simulink model "IEEE118_FULL_seed17_GFOL_RL_percgfor091_PyStable"  (R2023a)
(part 2 of 3)

  To Workspace_NET.vn102d : ToWorkspace  VariableName=vn102d  SampleTime=sim_config.Tsample
  To Workspace_NET.vn102q : ToWorkspace  VariableName=vn102q  SampleTime=sim_config.Tsample
  To Workspace_NET.vn103d : ToWorkspace  VariableName=vn103d  SampleTime=sim_config.Tsample
  To Workspace_NET.vn103q : ToWorkspace  VariableName=vn103q  SampleTime=sim_config.Tsample
  To Workspace_NET.vn104d : ToWorkspace  VariableName=vn104d  SampleTime=sim_config.Tsample
  To Workspace_NET.vn104q : ToWorkspace  VariableName=vn104q  SampleTime=sim_config.Tsample
  To Workspace_NET.vn105d : ToWorkspace  VariableName=vn105d  SampleTime=sim_config.Tsample
  To Workspace_NET.vn105q : ToWorkspace  VariableName=vn105q  SampleTime=sim_config.Tsample
  To Workspace_NET.vn106d : ToWorkspace  VariableName=vn106d  SampleTime=sim_config.Tsample
  To Workspace_NET.vn106q : ToWorkspace  VariableName=vn106q  SampleTime=sim_config.Tsample
  To Workspace_NET.vn107d : ToWorkspace  VariableName=vn107d  SampleTime=sim_config.Tsample
  To Workspace_NET.vn107q : ToWorkspace  VariableName=vn107q  SampleTime=sim_config.Tsample
  To Workspace_NET.vn108d : ToWorkspace  VariableName=vn108d  SampleTime=sim_config.Tsample
  To Workspace_NET.vn108q : ToWorkspace  VariableName=vn108q  SampleTime=sim_config.Tsample
  To Workspace_NET.vn109d : ToWorkspace  VariableName=vn109d  SampleTime=sim_config.Tsample
  To Workspace_NET.vn109q : ToWorkspace  VariableName=vn109q  SampleTime=sim_config.Tsample
  To Workspace_NET.vn110d : ToWorkspace  VariableName=vn110d  SampleTime=sim_config.Tsample
  To Workspace_NET.vn110q : ToWorkspace  VariableName=vn110q  SampleTime=sim_config.Tsample
  To Workspace_NET.vn112d : ToWorkspace  VariableName=vn112d  SampleTime=sim_config.Tsample
  To Workspace_NET.vn112q : ToWorkspace  VariableName=vn112q  SampleTime=sim_config.Tsample
  To Workspace_NET.vn113d : ToWorkspace  VariableName=vn113d  SampleTime=sim_config.Tsample
  To Workspace_NET.vn113q : ToWorkspace  VariableName=vn113q  SampleTime=sim_config.Tsample
  To Workspace_NET.vn114d : ToWorkspace  VariableName=vn114d  SampleTime=sim_config.Tsample
  To Workspace_NET.vn114q : ToWorkspace  VariableName=vn114q  SampleTime=sim_config.Tsample
  To Workspace_NET.vn115d : ToWorkspace  VariableName=vn115d  SampleTime=sim_config.Tsample
  To Workspace_NET.vn115q : ToWorkspace  VariableName=vn115q  SampleTime=sim_config.Tsample
  To Workspace_NET.vn117d : ToWorkspace  VariableName=vn117d  SampleTime=sim_config.Tsample
  To Workspace_NET.vn117q : ToWorkspace  VariableName=vn117q  SampleTime=sim_config.Tsample
  To Workspace_NET.vn118d : ToWorkspace  VariableName=vn118d  SampleTime=sim_config.Tsample
  To Workspace_NET.vn118q : ToWorkspace  VariableName=vn118q  SampleTime=sim_config.Tsample
  To Workspace_NET.vn11d : ToWorkspace  VariableName=vn11d  SampleTime=sim_config.Tsample
  To Workspace_NET.vn11q : ToWorkspace  VariableName=vn11q  SampleTime=sim_config.Tsample
  To Workspace_NET.vn12d : ToWorkspace  VariableName=vn12d  SampleTime=sim_config.Tsample
  To Workspace_NET.vn12q : ToWorkspace  VariableName=vn12q  SampleTime=sim_config.Tsample
  To Workspace_NET.vn13d : ToWorkspace  VariableName=vn13d  SampleTime=sim_config.Tsample
  To Workspace_NET.vn13q : ToWorkspace  VariableName=vn13q  SampleTime=sim_config.Tsample
  To Workspace_NET.vn14d : ToWorkspace  VariableName=vn14d  SampleTime=sim_config.Tsample
  To Workspace_NET.vn14q : ToWorkspace  VariableName=vn14q  SampleTime=sim_config.Tsample
  To Workspace_NET.vn15d : ToWorkspace  VariableName=vn15d  SampleTime=sim_config.Tsample
  To Workspace_NET.vn15q : ToWorkspace  VariableName=vn15q  SampleTime=sim_config.Tsample
  To Workspace_NET.vn16d : ToWorkspace  VariableName=vn16d  SampleTime=sim_config.Tsample
  To Workspace_NET.vn16q : ToWorkspace  VariableName=vn16q  SampleTime=sim_config.Tsample
  To Workspace_NET.vn17d : ToWorkspace  VariableName=vn17d  SampleTime=sim_config.Tsample
  To Workspace_NET.vn17q : ToWorkspace  VariableName=vn17q  SampleTime=sim_config.Tsample
  To Workspace_NET.vn18d : ToWorkspace  VariableName=vn18d  SampleTime=sim_config.Tsample
  To Workspace_NET.vn18q : ToWorkspace  VariableName=vn18q  SampleTime=sim_config.Tsample
  To Workspace_NET.vn19d : ToWorkspace  VariableName=vn19d  SampleTime=sim_config.Tsample
  To Workspace_NET.vn19q : ToWorkspace  VariableName=vn19q  SampleTime=sim_config.Tsample
  To Workspace_NET.vn1d : ToWorkspace  VariableName=vn1d  SampleTime=sim_config.Tsample
  To Workspace_NET.vn1q : ToWorkspace  VariableName=vn1q  SampleTime=sim_config.Tsample
  To Workspace_NET.vn20d : ToWorkspace  VariableName=vn20d  SampleTime=sim_config.Tsample
  To Workspace_NET.vn20q : ToWorkspace  VariableName=vn20q  SampleTime=sim_config.Tsample
  To Workspace_NET.vn21d : ToWorkspace  VariableName=vn21d  SampleTime=sim_config.Tsample
  To Workspace_NET.vn21q : ToWorkspace  VariableName=vn21q  SampleTime=sim_config.Tsample
  To Workspace_NET.vn22d : ToWorkspace  VariableName=vn22d  SampleTime=sim_config.Tsample
  To Workspace_NET.vn22q : ToWorkspace  VariableName=vn22q  SampleTime=sim_config.Tsample
  To Workspace_NET.vn23d : ToWorkspace  VariableName=vn23d  SampleTime=sim_config.Tsample
  To Workspace_NET.vn23q : ToWorkspace  VariableName=vn23q  SampleTime=sim_config.Tsample
  To Workspace_NET.vn24d : ToWorkspace  VariableName=vn24d  SampleTime=sim_config.Tsample
  To Workspace_NET.vn24q : ToWorkspace  VariableName=vn24q  SampleTime=sim_config.Tsample
  To Workspace_NET.vn25d : ToWorkspace  VariableName=vn25d  SampleTime=sim_config.Tsample
  To Workspace_NET.vn25q : ToWorkspace  VariableName=vn25q  SampleTime=sim_config.Tsample
  To Workspace_NET.vn26d : ToWorkspace  VariableName=vn26d  SampleTime=sim_config.Tsample
  To Workspace_NET.vn26q : ToWorkspace  VariableName=vn26q  SampleTime=sim_config.Tsample
  To Workspace_NET.vn27d : ToWorkspace  VariableName=vn27d  SampleTime=sim_config.Tsample
  To Workspace_NET.vn27q : ToWorkspace  VariableName=vn27q  SampleTime=sim_config.Tsample
  To Workspace_NET.vn28d : ToWorkspace  VariableName=vn28d  SampleTime=sim_config.Tsample
  To Workspace_NET.vn28q : ToWorkspace  VariableName=vn28q  SampleTime=sim_config.Tsample
  To Workspace_NET.vn29d : ToWorkspace  VariableName=vn29d  SampleTime=sim_config.Tsample
  To Workspace_NET.vn29q : ToWorkspace  VariableName=vn29q  SampleTime=sim_config.Tsample
  To Workspace_NET.vn2d : ToWorkspace  VariableName=vn2d  SampleTime=sim_config.Tsample
  To Workspace_NET.vn2q : ToWorkspace  VariableName=vn2q  SampleTime=sim_config.Tsample
  To Workspace_NET.vn30d : ToWorkspace  VariableName=vn30d  SampleTime=sim_config.Tsample
  To Workspace_NET.vn30q : ToWorkspace  VariableName=vn30q  SampleTime=sim_config.Tsample
  To Workspace_NET.vn31d : ToWorkspace  VariableName=vn31d  SampleTime=sim_config.Tsample
  To Workspace_NET.vn31q : ToWorkspace  VariableName=vn31q  SampleTime=sim_config.Tsample
  To Workspace_NET.vn32d : ToWorkspace  VariableName=vn32d  SampleTime=sim_config.Tsample
  To Workspace_NET.vn32q : ToWorkspace  VariableName=vn32q  SampleTime=sim_config.Tsample
  To Workspace_NET.vn33d : ToWorkspace  VariableName=vn33d  SampleTime=sim_config.Tsample
  To Workspace_NET.vn33q : ToWorkspace  VariableName=vn33q  SampleTime=sim_config.Tsample
  To Workspace_NET.vn34d : ToWorkspace  VariableName=vn34d  SampleTime=sim_config.Tsample
  To Workspace_NET.vn34q : ToWorkspace  VariableName=vn34q  SampleTime=sim_config.Tsample
  To Workspace_NET.vn35d : ToWorkspace  VariableName=vn35d  SampleTime=sim_config.Tsample
  To Workspace_NET.vn35q : ToWorkspace  VariableName=vn35q  SampleTime=sim_config.Tsample
  To Workspace_NET.vn36d : ToWorkspace  VariableName=vn36d  SampleTime=sim_config.Tsample
  To Workspace_NET.vn36q : ToWorkspace  VariableName=vn36q  SampleTime=sim_config.Tsample
  To Workspace_NET.vn37d : ToWorkspace  VariableName=vn37d  SampleTime=sim_config.Tsample
  To Workspace_NET.vn37q : ToWorkspace  VariableName=vn37q  SampleTime=sim_config.Tsample
  To Workspace_NET.vn38d : ToWorkspace  VariableName=vn38d  SampleTime=sim_config.Tsample
  To Workspace_NET.vn38q : ToWorkspace  VariableName=vn38q  SampleTime=sim_config.Tsample
  To Workspace_NET.vn39d : ToWorkspace  VariableName=vn39d  SampleTime=sim_config.Tsample
  To Workspace_NET.vn39q : ToWorkspace  VariableName=vn39q  SampleTime=sim_config.Tsample
  To Workspace_NET.vn3d : ToWorkspace  VariableName=vn3d  SampleTime=sim_config.Tsample
  To Workspace_NET.vn3q : ToWorkspace  VariableName=vn3q  SampleTime=sim_config.Tsample
  To Workspace_NET.vn40d : ToWorkspace  VariableName=vn40d  SampleTime=sim_config.Tsample
  To Workspace_NET.vn40q : ToWorkspace  VariableName=vn40q  SampleTime=sim_config.Tsample
  To Workspace_NET.vn41d : ToWorkspace  VariableName=vn41d  SampleTime=sim_config.Tsample
  To Workspace_NET.vn41q : ToWorkspace  VariableName=vn41q  SampleTime=sim_config.Tsample
  To Workspace_NET.vn42d : ToWorkspace  VariableName=vn42d  SampleTime=sim_config.Tsample
  To Workspace_NET.vn42q : ToWorkspace  VariableName=vn42q  SampleTime=sim_config.Tsample
  To Workspace_NET.vn43d : ToWorkspace  VariableName=vn43d  SampleTime=sim_config.Tsample
  To Workspace_NET.vn43q : ToWorkspace  VariableName=vn43q  SampleTime=sim_config.Tsample
  To Workspace_NET.vn44d : ToWorkspace  VariableName=vn44d  SampleTime=sim_config.Tsample
  To Workspace_NET.vn44q : ToWorkspace  VariableName=vn44q  SampleTime=sim_config.Tsample
  To Workspace_NET.vn45d : ToWorkspace  VariableName=vn45d  SampleTime=sim_config.Tsample
  To Workspace_NET.vn45q : ToWorkspace  VariableName=vn45q  SampleTime=sim_config.Tsample
  To Workspace_NET.vn46d : ToWorkspace  VariableName=vn46d  SampleTime=sim_config.Tsample
  To Workspace_NET.vn46q : ToWorkspace  VariableName=vn46q  SampleTime=sim_config.Tsample
  To Workspace_NET.vn47d : ToWorkspace  VariableName=vn47d  SampleTime=sim_config.Tsample
  To Workspace_NET.vn47q : ToWorkspace  VariableName=vn47q  SampleTime=sim_config.Tsample
  To Workspace_NET.vn48d : ToWorkspace  VariableName=vn48d  SampleTime=sim_config.Tsample
  To Workspace_NET.vn48q : ToWorkspace  VariableName=vn48q  SampleTime=sim_config.Tsample
  To Workspace_NET.vn49d : ToWorkspace  VariableName=vn49d  SampleTime=sim_config.Tsample
  To Workspace_NET.vn49q : ToWorkspace  VariableName=vn49q  SampleTime=sim_config.Tsample
  To Workspace_NET.vn4d : ToWorkspace  VariableName=vn4d  SampleTime=sim_config.Tsample
  To Workspace_NET.vn4q : ToWorkspace  VariableName=vn4q  SampleTime=sim_config.Tsample
  To Workspace_NET.vn50d : ToWorkspace  VariableName=vn50d  SampleTime=sim_config.Tsample
  To Workspace_NET.vn50q : ToWorkspace  VariableName=vn50q  SampleTime=sim_config.Tsample
  To Workspace_NET.vn51d : ToWorkspace  VariableName=vn51d  SampleTime=sim_config.Tsample
  To Workspace_NET.vn51q : ToWorkspace  VariableName=vn51q  SampleTime=sim_config.Tsample
  To Workspace_NET.vn52d : ToWorkspace  VariableName=vn52d  SampleTime=sim_config.Tsample
  To Workspace_NET.vn52q : ToWorkspace  VariableName=vn52q  SampleTime=sim_config.Tsample
  To Workspace_NET.vn53d : ToWorkspace  VariableName=vn53d  SampleTime=sim_config.Tsample
  To Workspace_NET.vn53q : ToWorkspace  VariableName=vn53q  SampleTime=sim_config.Tsample
  To Workspace_NET.vn54d : ToWorkspace  VariableName=vn54d  SampleTime=sim_config.Tsample
  To Workspace_NET.vn54q : ToWorkspace  VariableName=vn54q  SampleTime=sim_config.Tsample
  To Workspace_NET.vn55d : ToWorkspace  VariableName=vn55d  SampleTime=sim_config.Tsample
  To Workspace_NET.vn55q : ToWorkspace  VariableName=vn55q  SampleTime=sim_config.Tsample
  To Workspace_NET.vn56d : ToWorkspace  VariableName=vn56d  SampleTime=sim_config.Tsample
  To Workspace_NET.vn56q : ToWorkspace  VariableName=vn56q  SampleTime=sim_config.Tsample
  To Workspace_NET.vn57d : ToWorkspace  VariableName=vn57d  SampleTime=sim_config.Tsample
  To Workspace_NET.vn57q : ToWorkspace  VariableName=vn57q  SampleTime=sim_config.Tsample
  To Workspace_NET.vn58d : ToWorkspace  VariableName=vn58d  SampleTime=sim_config.Tsample
  To Workspace_NET.vn58q : ToWorkspace  VariableName=vn58q  SampleTime=sim_config.Tsample
  To Workspace_NET.vn59d : ToWorkspace  VariableName=vn59d  SampleTime=sim_config.Tsample
  To Workspace_NET.vn59q : ToWorkspace  VariableName=vn59q  SampleTime=sim_config.Tsample
  To Workspace_NET.vn5d : ToWorkspace  VariableName=vn5d  SampleTime=sim_config.Tsample
  To Workspace_NET.vn5q : ToWorkspace  VariableName=vn5q  SampleTime=sim_config.Tsample
  To Workspace_NET.vn60d : ToWorkspace  VariableName=vn60d  SampleTime=sim_config.Tsample
  To Workspace_NET.vn60q : ToWorkspace  VariableName=vn60q  SampleTime=sim_config.Tsample
  To Workspace_NET.vn61d : ToWorkspace  VariableName=vn61d  SampleTime=sim_config.Tsample
  To Workspace_NET.vn61q : ToWorkspace  VariableName=vn61q  SampleTime=sim_config.Tsample
  To Workspace_NET.vn62d : ToWorkspace  VariableName=vn62d  SampleTime=sim_config.Tsample
  To Workspace_NET.vn62q : ToWorkspace  VariableName=vn62q  SampleTime=sim_config.Tsample
  To Workspace_NET.vn63d : ToWorkspace  VariableName=vn63d  SampleTime=sim_config.Tsample
  To Workspace_NET.vn63q : ToWorkspace  VariableName=vn63q  SampleTime=sim_config.Tsample
  To Workspace_NET.vn64d : ToWorkspace  VariableName=vn64d  SampleTime=sim_config.Tsample
  To Workspace_NET.vn64q : ToWorkspace  VariableName=vn64q  SampleTime=sim_config.Tsample
  To Workspace_NET.vn65d : ToWorkspace  VariableName=vn65d  SampleTime=sim_config.Tsample
  To Workspace_NET.vn65q : ToWorkspace  VariableName=vn65q  SampleTime=sim_config.Tsample
  To Workspace_NET.vn66d : ToWorkspace  VariableName=vn66d  SampleTime=sim_config.Tsample
  To Workspace_NET.vn66q : ToWorkspace  VariableName=vn66q  SampleTime=sim_config.Tsample
  To Workspace_NET.vn67d : ToWorkspace  VariableName=vn67d  SampleTime=sim_config.Tsample
  To Workspace_NET.vn67q : ToWorkspace  VariableName=vn67q  SampleTime=sim_config.Tsample
  To Workspace_NET.vn68d : ToWorkspace  VariableName=vn68d  SampleTime=sim_config.Tsample
  To Workspace_NET.vn68q : ToWorkspace  VariableName=vn68q  SampleTime=sim_config.Tsample
  To Workspace_NET.vn69d : ToWorkspace  VariableName=vn69d  SampleTime=sim_config.Tsample
  To Workspace_NET.vn69q : ToWorkspace  VariableName=vn69q  SampleTime=sim_config.Tsample
  To Workspace_NET.vn6d : ToWorkspace  VariableName=vn6d  SampleTime=sim_config.Tsample
  To Workspace_NET.vn6q : ToWorkspace  VariableName=vn6q  SampleTime=sim_config.Tsample
  To Workspace_NET.vn70d : ToWorkspace  VariableName=vn70d  SampleTime=sim_config.Tsample
  To Workspace_NET.vn70q : ToWorkspace  VariableName=vn70q  SampleTime=sim_config.Tsample
  To Workspace_NET.vn71d : ToWorkspace  VariableName=vn71d  SampleTime=sim_config.Tsample
  To Workspace_NET.vn71q : ToWorkspace  VariableName=vn71q  SampleTime=sim_config.Tsample
  To Workspace_NET.vn72d : ToWorkspace  VariableName=vn72d  SampleTime=sim_config.Tsample
  To Workspace_NET.vn72q : ToWorkspace  VariableName=vn72q  SampleTime=sim_config.Tsample
  To Workspace_NET.vn73d : ToWorkspace  VariableName=vn73d  SampleTime=sim_config.Tsample
  To Workspace_NET.vn73q : ToWorkspace  VariableName=vn73q  SampleTime=sim_config.Tsample
  To Workspace_NET.vn74d : ToWorkspace  VariableName=vn74d  SampleTime=sim_config.Tsample
  To Workspace_NET.vn74q : ToWorkspace  VariableName=vn74q  SampleTime=sim_config.Tsample
  To Workspace_NET.vn75d : ToWorkspace  VariableName=vn75d  SampleTime=sim_config.Tsample
  To Workspace_NET.vn75q : ToWorkspace  VariableName=vn75q  SampleTime=sim_config.Tsample
  To Workspace_NET.vn76d : ToWorkspace  VariableName=vn76d  SampleTime=sim_config.Tsample
  To Workspace_NET.vn76q : ToWorkspace  VariableName=vn76q  SampleTime=sim_config.Tsample
  To Workspace_NET.vn77d : ToWorkspace  VariableName=vn77d  SampleTime=sim_config.Tsample
  To Workspace_NET.vn77q : ToWorkspace  VariableName=vn77q  SampleTime=sim_config.Tsample
  To Workspace_NET.vn78d : ToWorkspace  VariableName=vn78d  SampleTime=sim_config.Tsample
  To Workspace_NET.vn78q : ToWorkspace  VariableName=vn78q  SampleTime=sim_config.Tsample
  To Workspace_NET.vn79d : ToWorkspace  VariableName=vn79d  SampleTime=sim_config.Tsample
  To Workspace_NET.vn79q : ToWorkspace  VariableName=vn79q  SampleTime=sim_config.Tsample
  To Workspace_NET.vn7d : ToWorkspace  VariableName=vn7d  SampleTime=sim_config.Tsample
  To Workspace_NET.vn7q : ToWorkspace  VariableName=vn7q  SampleTime=sim_config.Tsample
  To Workspace_NET.vn80d : ToWorkspace  VariableName=vn80d  SampleTime=sim_config.Tsample
  To Workspace_NET.vn80q : ToWorkspace  VariableName=vn80q  SampleTime=sim_config.Tsample
  To Workspace_NET.vn81d : ToWorkspace  VariableName=vn81d  SampleTime=sim_config.Tsample
  To Workspace_NET.vn81q : ToWorkspace  VariableName=vn81q  SampleTime=sim_config.Tsample
  To Workspace_NET.vn82d : ToWorkspace  VariableName=vn82d  SampleTime=sim_config.Tsample
  To Workspace_NET.vn82q : ToWorkspace  VariableName=vn82q  SampleTime=sim_config.Tsample
  To Workspace_NET.vn83d : ToWorkspace  VariableName=vn83d  SampleTime=sim_config.Tsample
  To Workspace_NET.vn83q : ToWorkspace  VariableName=vn83q  SampleTime=sim_config.Tsample
  To Workspace_NET.vn84d : ToWorkspace  VariableName=vn84d  SampleTime=sim_config.Tsample
  To Workspace_NET.vn84q : ToWorkspace  VariableName=vn84q  SampleTime=sim_config.Tsample
  To Workspace_NET.vn85d : ToWorkspace  VariableName=vn85d  SampleTime=sim_config.Tsample
  To Workspace_NET.vn85q : ToWorkspace  VariableName=vn85q  SampleTime=sim_config.Tsample
  To Workspace_NET.vn86d : ToWorkspace  VariableName=vn86d  SampleTime=sim_config.Tsample
  To Workspace_NET.vn86q : ToWorkspace  VariableName=vn86q  SampleTime=sim_config.Tsample
  To Workspace_NET.vn88d : ToWorkspace  VariableName=vn88d  SampleTime=sim_config.Tsample
  To Workspace_NET.vn88q : ToWorkspace  VariableName=vn88q  SampleTime=sim_config.Tsample
  To Workspace_NET.vn89d : ToWorkspace  VariableName=vn89d  SampleTime=sim_config.Tsample
  To Workspace_NET.vn89q : ToWorkspace  VariableName=vn89q  SampleTime=sim_config.Tsample
  To Workspace_NET.vn8d : ToWorkspace  VariableName=vn8d  SampleTime=sim_config.Tsample
  To Workspace_NET.vn8q : ToWorkspace  VariableName=vn8q  SampleTime=sim_config.Tsample
  To Workspace_NET.vn90d : ToWorkspace  VariableName=vn90d  SampleTime=sim_config.Tsample
  To Workspace_NET.vn90q : ToWorkspace  VariableName=vn90q  SampleTime=sim_config.Tsample
  To Workspace_NET.vn91d : ToWorkspace  VariableName=vn91d  SampleTime=sim_config.Tsample
  To Workspace_NET.vn91q : ToWorkspace  VariableName=vn91q  SampleTime=sim_config.Tsample
  To Workspace_NET.vn92d : ToWorkspace  VariableName=vn92d  SampleTime=sim_config.Tsample
  To Workspace_NET.vn92q : ToWorkspace  VariableName=vn92q  SampleTime=sim_config.Tsample
  To Workspace_NET.vn93d : ToWorkspace  VariableName=vn93d  SampleTime=sim_config.Tsample
  To Workspace_NET.vn93q : ToWorkspace  VariableName=vn93q  SampleTime=sim_config.Tsample
  To Workspace_NET.vn94d : ToWorkspace  VariableName=vn94d  SampleTime=sim_config.Tsample
  To Workspace_NET.vn94q : ToWorkspace  VariableName=vn94q  SampleTime=sim_config.Tsample
  To Workspace_NET.vn95d : ToWorkspace  VariableName=vn95d  SampleTime=sim_config.Tsample
  To Workspace_NET.vn95q : ToWorkspace  VariableName=vn95q  SampleTime=sim_config.Tsample
  To Workspace_NET.vn96d : ToWorkspace  VariableName=vn96d  SampleTime=sim_config.Tsample
  To Workspace_NET.vn96q : ToWorkspace  VariableName=vn96q  SampleTime=sim_config.Tsample
  To Workspace_NET.vn97d : ToWorkspace  VariableName=vn97d  SampleTime=sim_config.Tsample
  To Workspace_NET.vn97q : ToWorkspace  VariableName=vn97q  SampleTime=sim_config.Tsample
  To Workspace_NET.vn98d : ToWorkspace  VariableName=vn98d  SampleTime=sim_config.Tsample
  To Workspace_NET.vn98q : ToWorkspace  VariableName=vn98q  SampleTime=sim_config.Tsample
  To Workspace_NET.vn99d : ToWorkspace  VariableName=vn99d  SampleTime=sim_config.Tsample
  To Workspace_NET.vn99q : ToWorkspace  VariableName=vn99q  SampleTime=sim_config.Tsample
  To Workspace_P_Load1 : ToWorkspace  VariableName=P_Load1  SampleTime=sim_config.Tsample
  To Workspace_P_Load10 : ToWorkspace  VariableName=P_Load10  SampleTime=sim_config.Tsample
  To Workspace_P_Load11 : ToWorkspace  VariableName=P_Load11  SampleTime=sim_config.Tsample
  To Workspace_P_Load12 : ToWorkspace  VariableName=P_Load12  SampleTime=sim_config.Tsample
  To Workspace_P_Load13 : ToWorkspace  VariableName=P_Load13  SampleTime=sim_config.Tsample
  To Workspace_P_Load14 : ToWorkspace  VariableName=P_Load14  SampleTime=sim_config.Tsample
  To Workspace_P_Load15 : ToWorkspace  VariableName=P_Load15  SampleTime=sim_config.Tsample
  To Workspace_P_Load16 : ToWorkspace  VariableName=P_Load16  SampleTime=sim_config.Tsample
  To Workspace_P_Load17 : ToWorkspace  VariableName=P_Load17  SampleTime=sim_config.Tsample
  To Workspace_P_Load18 : ToWorkspace  VariableName=P_Load18  SampleTime=sim_config.Tsample
  To Workspace_P_Load19 : ToWorkspace  VariableName=P_Load19  SampleTime=sim_config.Tsample
  To Workspace_P_Load2 : ToWorkspace  VariableName=P_Load2  SampleTime=sim_config.Tsample
  To Workspace_P_Load20 : ToWorkspace  VariableName=P_Load20  SampleTime=sim_config.Tsample
  To Workspace_P_Load21 : ToWorkspace  VariableName=P_Load21  SampleTime=sim_config.Tsample
  To Workspace_P_Load22 : ToWorkspace  VariableName=P_Load22  SampleTime=sim_config.Tsample
  To Workspace_P_Load23 : ToWorkspace  VariableName=P_Load23  SampleTime=sim_config.Tsample
  To Workspace_P_Load24 : ToWorkspace  VariableName=P_Load24  SampleTime=sim_config.Tsample
  To Workspace_P_Load25 : ToWorkspace  VariableName=P_Load25  SampleTime=sim_config.Tsample
  To Workspace_P_Load26 : ToWorkspace  VariableName=P_Load26  SampleTime=sim_config.Tsample
  To Workspace_P_Load27 : ToWorkspace  VariableName=P_Load27  SampleTime=sim_config.Tsample
  To Workspace_P_Load28 : ToWorkspace  VariableName=P_Load28  SampleTime=sim_config.Tsample
  To Workspace_P_Load29 : ToWorkspace  VariableName=P_Load29  SampleTime=sim_config.Tsample
  To Workspace_P_Load3 : ToWorkspace  VariableName=P_Load3  SampleTime=sim_config.Tsample
  To Workspace_P_Load30 : ToWorkspace  VariableName=P_Load30  SampleTime=sim_config.Tsample
  To Workspace_P_Load31 : ToWorkspace  VariableName=P_Load31  SampleTime=sim_config.Tsample
  To Workspace_P_Load32 : ToWorkspace  VariableName=P_Load32  SampleTime=sim_config.Tsample
  To Workspace_P_Load33 : ToWorkspace  VariableName=P_Load33  SampleTime=sim_config.Tsample
  To Workspace_P_Load34 : ToWorkspace  VariableName=P_Load34  SampleTime=sim_config.Tsample
  To Workspace_P_Load35 : ToWorkspace  VariableName=P_Load35  SampleTime=sim_config.Tsample
  To Workspace_P_Load36 : ToWorkspace  VariableName=P_Load36  SampleTime=sim_config.Tsample
  To Workspace_P_Load37 : ToWorkspace  VariableName=P_Load37  SampleTime=sim_config.Tsample
  To Workspace_P_Load38 : ToWorkspace  VariableName=P_Load38  SampleTime=sim_config.Tsample
  To Workspace_P_Load39 : ToWorkspace  VariableName=P_Load39  SampleTime=sim_config.Tsample
  To Workspace_P_Load4 : ToWorkspace  VariableName=P_Load4  SampleTime=sim_config.Tsample
  To Workspace_P_Load40 : ToWorkspace  VariableName=P_Load40  SampleTime=sim_config.Tsample
  To Workspace_P_Load41 : ToWorkspace  VariableName=P_Load41  SampleTime=sim_config.Tsample
  To Workspace_P_Load42 : ToWorkspace  VariableName=P_Load42  SampleTime=sim_config.Tsample
  To Workspace_P_Load43 : ToWorkspace  VariableName=P_Load43  SampleTime=sim_config.Tsample
  To Workspace_P_Load44 : ToWorkspace  VariableName=P_Load44  SampleTime=sim_config.Tsample
  To Workspace_P_Load45 : ToWorkspace  VariableName=P_Load45  SampleTime=sim_config.Tsample
  To Workspace_P_Load46 : ToWorkspace  VariableName=P_Load46  SampleTime=sim_config.Tsample
  To Workspace_P_Load47 : ToWorkspace  VariableName=P_Load47  SampleTime=sim_config.Tsample
  To Workspace_P_Load48 : ToWorkspace  VariableName=P_Load48  SampleTime=sim_config.Tsample
  To Workspace_P_Load49 : ToWorkspace  VariableName=P_Load49  SampleTime=sim_config.Tsample
  To Workspace_P_Load5 : ToWorkspace  VariableName=P_Load5  SampleTime=sim_config.Tsample
  To Workspace_P_Load50 : ToWorkspace  VariableName=P_Load50  SampleTime=sim_config.Tsample
  To Workspace_P_Load51 : ToWorkspace  VariableName=P_Load51  SampleTime=sim_config.Tsample
  To Workspace_P_Load52 : ToWorkspace  VariableName=P_Load52  SampleTime=sim_config.Tsample
  To Workspace_P_Load53 : ToWorkspace  VariableName=P_Load53  SampleTime=sim_config.Tsample
  To Workspace_P_Load54 : ToWorkspace  VariableName=P_Load54  SampleTime=sim_config.Tsample
  To Workspace_P_Load55 : ToWorkspace  VariableName=P_Load55  SampleTime=sim_config.Tsample
  To Workspace_P_Load56 : ToWorkspace  VariableName=P_Load56  SampleTime=sim_config.Tsample
  To Workspace_P_Load57 : ToWorkspace  VariableName=P_Load57  SampleTime=sim_config.Tsample
  To Workspace_P_Load58 : ToWorkspace  VariableName=P_Load58  SampleTime=sim_config.Tsample
  To Workspace_P_Load59 : ToWorkspace  VariableName=P_Load59  SampleTime=sim_config.Tsample
  To Workspace_P_Load6 : ToWorkspace  VariableName=P_Load6  SampleTime=sim_config.Tsample
  To Workspace_P_Load60 : ToWorkspace  VariableName=P_Load60  SampleTime=sim_config.Tsample
  To Workspace_P_Load61 : ToWorkspace  VariableName=P_Load61  SampleTime=sim_config.Tsample
  To Workspace_P_Load62 : ToWorkspace  VariableName=P_Load62  SampleTime=sim_config.Tsample
  To Workspace_P_Load63 : ToWorkspace  VariableName=P_Load63  SampleTime=sim_config.Tsample
  To Workspace_P_Load64 : ToWorkspace  VariableName=P_Load64  SampleTime=sim_config.Tsample
  To Workspace_P_Load65 : ToWorkspace  VariableName=P_Load65  SampleTime=sim_config.Tsample
  To Workspace_P_Load66 : ToWorkspace  VariableName=P_Load66  SampleTime=sim_config.Tsample
  To Workspace_P_Load67 : ToWorkspace  VariableName=P_Load67  SampleTime=sim_config.Tsample
  To Workspace_P_Load68 : ToWorkspace  VariableName=P_Load68  SampleTime=sim_config.Tsample
  To Workspace_P_Load69 : ToWorkspace  VariableName=P_Load69  SampleTime=sim_config.Tsample
  To Workspace_P_Load7 : ToWorkspace  VariableName=P_Load7  SampleTime=sim_config.Tsample
  To Workspace_P_Load70 : ToWorkspace  VariableName=P_Load70  SampleTime=sim_config.Tsample
  To Workspace_P_Load71 : ToWorkspace  VariableName=P_Load71  SampleTime=sim_config.Tsample
  To Workspace_P_Load72 : ToWorkspace  VariableName=P_Load72  SampleTime=sim_config.Tsample
  To Workspace_P_Load73 : ToWorkspace  VariableName=P_Load73  SampleTime=sim_config.Tsample
  To Workspace_P_Load74 : ToWorkspace  VariableName=P_Load74  SampleTime=sim_config.Tsample
  To Workspace_P_Load75 : ToWorkspace  VariableName=P_Load75  SampleTime=sim_config.Tsample
  To Workspace_P_Load76 : ToWorkspace  VariableName=P_Load76  SampleTime=sim_config.Tsample
  To Workspace_P_Load77 : ToWorkspace  VariableName=P_Load77  SampleTime=sim_config.Tsample
  To Workspace_P_Load78 : ToWorkspace  VariableName=P_Load78  SampleTime=sim_config.Tsample
  To Workspace_P_Load79 : ToWorkspace  VariableName=P_Load79  SampleTime=sim_config.Tsample
  To Workspace_P_Load8 : ToWorkspace  VariableName=P_Load8  SampleTime=sim_config.Tsample
  To Workspace_P_Load80 : ToWorkspace  VariableName=P_Load80  SampleTime=sim_config.Tsample
  To Workspace_P_Load81 : ToWorkspace  VariableName=P_Load81  SampleTime=sim_config.Tsample
  To Workspace_P_Load82 : ToWorkspace  VariableName=P_Load82  SampleTime=sim_config.Tsample
  To Workspace_P_Load83 : ToWorkspace  VariableName=P_Load83  SampleTime=sim_config.Tsample
  To Workspace_P_Load84 : ToWorkspace  VariableName=P_Load84  SampleTime=sim_config.Tsample
  To Workspace_P_Load85 : ToWorkspace  VariableName=P_Load85  SampleTime=sim_config.Tsample
  To Workspace_P_Load86 : ToWorkspace  VariableName=P_Load86  SampleTime=sim_config.Tsample
  To Workspace_P_Load87 : ToWorkspace  VariableName=P_Load87  SampleTime=sim_config.Tsample
  To Workspace_P_Load88 : ToWorkspace  VariableName=P_Load88  SampleTime=sim_config.Tsample
  To Workspace_P_Load89 : ToWorkspace  VariableName=P_Load89  SampleTime=sim_config.Tsample
  To Workspace_P_Load9 : ToWorkspace  VariableName=P_Load9  SampleTime=sim_config.Tsample
  To Workspace_P_Load90 : ToWorkspace  VariableName=P_Load90  SampleTime=sim_config.Tsample
  To Workspace_P_Load91 : ToWorkspace  VariableName=P_Load91  SampleTime=sim_config.Tsample
  To Workspace_P_SG1 : ToWorkspace  VariableName=P_SG1  SampleTime=sim_config.Tsample
  To Workspace_P_SG10 : ToWorkspace  VariableName=P_SG10  SampleTime=sim_config.Tsample
  To Workspace_P_SG11 : ToWorkspace  VariableName=P_SG11  SampleTime=sim_config.Tsample
  To Workspace_P_SG12 : ToWorkspace  VariableName=P_SG12  SampleTime=sim_config.Tsample
  To Workspace_P_SG13 : ToWorkspace  VariableName=P_SG13  SampleTime=sim_config.Tsample
  To Workspace_P_SG14 : ToWorkspace  VariableName=P_SG14  SampleTime=sim_config.Tsample
  To Workspace_P_SG15 : ToWorkspace  VariableName=P_SG15  SampleTime=sim_config.Tsample
  To Workspace_P_SG16 : ToWorkspace  VariableName=P_SG16  SampleTime=sim_config.Tsample
  To Workspace_P_SG17 : ToWorkspace  VariableName=P_SG17  SampleTime=sim_config.Tsample
  To Workspace_P_SG18 : ToWorkspace  VariableName=P_SG18  SampleTime=sim_config.Tsample
  To Workspace_P_SG19 : ToWorkspace  VariableName=P_SG19  SampleTime=sim_config.Tsample
  To Workspace_P_SG2 : ToWorkspace  VariableName=P_SG2  SampleTime=sim_config.Tsample
  To Workspace_P_SG20 : ToWorkspace  VariableName=P_SG20  SampleTime=sim_config.Tsample
  To Workspace_P_SG21 : ToWorkspace  VariableName=P_SG21  SampleTime=sim_config.Tsample
  To Workspace_P_SG22 : ToWorkspace  VariableName=P_SG22  SampleTime=sim_config.Tsample
  To Workspace_P_SG23 : ToWorkspace  VariableName=P_SG23  SampleTime=sim_config.Tsample
  To Workspace_P_SG24 : ToWorkspace  VariableName=P_SG24  SampleTime=sim_config.Tsample
  To Workspace_P_SG25 : ToWorkspace  VariableName=P_SG25  SampleTime=sim_config.Tsample
  To Workspace_P_SG26 : ToWorkspace  VariableName=P_SG26  SampleTime=sim_config.Tsample
  To Workspace_P_SG3 : ToWorkspace  VariableName=P_SG3  SampleTime=sim_config.Tsample
  To Workspace_P_SG4 : ToWorkspace  VariableName=P_SG4  SampleTime=sim_config.Tsample
  To Workspace_P_SG5 : ToWorkspace  VariableName=P_SG5  SampleTime=sim_config.Tsample
  To Workspace_P_SG6 : ToWorkspace  VariableName=P_SG6  SampleTime=sim_config.Tsample
  To Workspace_P_SG7 : ToWorkspace  VariableName=P_SG7  SampleTime=sim_config.Tsample
  To Workspace_P_SG8 : ToWorkspace  VariableName=P_SG8  SampleTime=sim_config.Tsample
  To Workspace_P_SG9 : ToWorkspace  VariableName=P_SG9  SampleTime=sim_config.Tsample
  To Workspace_P_VSC1 : ToWorkspace  VariableName=P_VSC1  SampleTime=sim_config.Tsample
  To Workspace_P_VSC10 : ToWorkspace  VariableName=P_VSC10  SampleTime=sim_config.Tsample
  To Workspace_P_VSC11 : ToWorkspace  VariableName=P_VSC11  SampleTime=sim_config.Tsample
  To Workspace_P_VSC12 : ToWorkspace  VariableName=P_VSC12  SampleTime=sim_config.Tsample
  To Workspace_P_VSC13 : ToWorkspace  VariableName=P_VSC13  SampleTime=sim_config.Tsample
  To Workspace_P_VSC14 : ToWorkspace  VariableName=P_VSC14  SampleTime=sim_config.Tsample
  To Workspace_P_VSC15 : ToWorkspace  VariableName=P_VSC15  SampleTime=sim_config.Tsample
  To Workspace_P_VSC16 : ToWorkspace  VariableName=P_VSC16  SampleTime=sim_config.Tsample
  To Workspace_P_VSC17 : ToWorkspace  VariableName=P_VSC17  SampleTime=sim_config.Tsample
  To Workspace_P_VSC18 : ToWorkspace  VariableName=P_VSC18  SampleTime=sim_config.Tsample
  To Workspace_P_VSC19 : ToWorkspace  VariableName=P_VSC19  SampleTime=sim_config.Tsample
  To Workspace_P_VSC2 : ToWorkspace  VariableName=P_VSC2  SampleTime=sim_config.Tsample
  To Workspace_P_VSC20 : ToWorkspace  VariableName=P_VSC20  SampleTime=sim_config.Tsample
  To Workspace_P_VSC3 : ToWorkspace  VariableName=P_VSC3  SampleTime=sim_config.Tsample
  To Workspace_P_VSC4 : ToWorkspace  VariableName=P_VSC4  SampleTime=sim_config.Tsample
  To Workspace_P_VSC5 : ToWorkspace  VariableName=P_VSC5  SampleTime=sim_config.Tsample
  To Workspace_P_VSC6 : ToWorkspace  VariableName=P_VSC6  SampleTime=sim_config.Tsample
  To Workspace_P_VSC7 : ToWorkspace  VariableName=P_VSC7  SampleTime=sim_config.Tsample
  To Workspace_P_VSC8 : ToWorkspace  VariableName=P_VSC8  SampleTime=sim_config.Tsample
  To Workspace_P_VSC9 : ToWorkspace  VariableName=P_VSC9  SampleTime=sim_config.Tsample
  To Workspace_Q_Load1 : ToWorkspace  VariableName=Q_Load1  SampleTime=sim_config.Tsample
  To Workspace_Q_Load10 : ToWorkspace  VariableName=Q_Load10  SampleTime=sim_config.Tsample
  To Workspace_Q_Load11 : ToWorkspace  VariableName=Q_Load11  SampleTime=sim_config.Tsample
  To Workspace_Q_Load12 : ToWorkspace  VariableName=Q_Load12  SampleTime=sim_config.Tsample
  To Workspace_Q_Load13 : ToWorkspace  VariableName=Q_Load13  SampleTime=sim_config.Tsample
  To Workspace_Q_Load14 : ToWorkspace  VariableName=Q_Load14  SampleTime=sim_config.Tsample
  To Workspace_Q_Load15 : ToWorkspace  VariableName=Q_Load15  SampleTime=sim_config.Tsample
  To Workspace_Q_Load16 : ToWorkspace  VariableName=Q_Load16  SampleTime=sim_config.Tsample
  To Workspace_Q_Load17 : ToWorkspace  VariableName=Q_Load17  SampleTime=sim_config.Tsample
  To Workspace_Q_Load18 : ToWorkspace  VariableName=Q_Load18  SampleTime=sim_config.Tsample
  To Workspace_Q_Load19 : ToWorkspace  VariableName=Q_Load19  SampleTime=sim_config.Tsample
  To Workspace_Q_Load2 : ToWorkspace  VariableName=Q_Load2  SampleTime=sim_config.Tsample
  To Workspace_Q_Load20 : ToWorkspace  VariableName=Q_Load20  SampleTime=sim_config.Tsample
  To Workspace_Q_Load21 : ToWorkspace  VariableName=Q_Load21  SampleTime=sim_config.Tsample
  To Workspace_Q_Load22 : ToWorkspace  VariableName=Q_Load22  SampleTime=sim_config.Tsample
  To Workspace_Q_Load23 : ToWorkspace  VariableName=Q_Load23  SampleTime=sim_config.Tsample
  To Workspace_Q_Load24 : ToWorkspace  VariableName=Q_Load24  SampleTime=sim_config.Tsample
  To Workspace_Q_Load25 : ToWorkspace  VariableName=Q_Load25  SampleTime=sim_config.Tsample
  To Workspace_Q_Load26 : ToWorkspace  VariableName=Q_Load26  SampleTime=sim_config.Tsample
  To Workspace_Q_Load27 : ToWorkspace  VariableName=Q_Load27  SampleTime=sim_config.Tsample
  To Workspace_Q_Load28 : ToWorkspace  VariableName=Q_Load28  SampleTime=sim_config.Tsample
  To Workspace_Q_Load29 : ToWorkspace  VariableName=Q_Load29  SampleTime=sim_config.Tsample
  To Workspace_Q_Load3 : ToWorkspace  VariableName=Q_Load3  SampleTime=sim_config.Tsample
  To Workspace_Q_Load30 : ToWorkspace  VariableName=Q_Load30  SampleTime=sim_config.Tsample
  To Workspace_Q_Load31 : ToWorkspace  VariableName=Q_Load31  SampleTime=sim_config.Tsample
  To Workspace_Q_Load32 : ToWorkspace  VariableName=Q_Load32  SampleTime=sim_config.Tsample
  To Workspace_Q_Load33 : ToWorkspace  VariableName=Q_Load33  SampleTime=sim_config.Tsample
  To Workspace_Q_Load34 : ToWorkspace  VariableName=Q_Load34  SampleTime=sim_config.Tsample
  To Workspace_Q_Load35 : ToWorkspace  VariableName=Q_Load35  SampleTime=sim_config.Tsample
  To Workspace_Q_Load36 : ToWorkspace  VariableName=Q_Load36  SampleTime=sim_config.Tsample
  To Workspace_Q_Load37 : ToWorkspace  VariableName=Q_Load37  SampleTime=sim_config.Tsample
  To Workspace_Q_Load38 : ToWorkspace  VariableName=Q_Load38  SampleTime=sim_config.Tsample
  To Workspace_Q_Load39 : ToWorkspace  VariableName=Q_Load39  SampleTime=sim_config.Tsample
  To Workspace_Q_Load4 : ToWorkspace  VariableName=Q_Load4  SampleTime=sim_config.Tsample
  To Workspace_Q_Load40 : ToWorkspace  VariableName=Q_Load40  SampleTime=sim_config.Tsample
  To Workspace_Q_Load41 : ToWorkspace  VariableName=Q_Load41  SampleTime=sim_config.Tsample
  To Workspace_Q_Load42 : ToWorkspace  VariableName=Q_Load42  SampleTime=sim_config.Tsample
  To Workspace_Q_Load43 : ToWorkspace  VariableName=Q_Load43  SampleTime=sim_config.Tsample
  To Workspace_Q_Load44 : ToWorkspace  VariableName=Q_Load44  SampleTime=sim_config.Tsample
  To Workspace_Q_Load45 : ToWorkspace  VariableName=Q_Load45  SampleTime=sim_config.Tsample
  To Workspace_Q_Load46 : ToWorkspace  VariableName=Q_Load46  SampleTime=sim_config.Tsample
  To Workspace_Q_Load47 : ToWorkspace  VariableName=Q_Load47  SampleTime=sim_config.Tsample
  To Workspace_Q_Load48 : ToWorkspace  VariableName=Q_Load48  SampleTime=sim_config.Tsample
  To Workspace_Q_Load49 : ToWorkspace  VariableName=Q_Load49  SampleTime=sim_config.Tsample
  To Workspace_Q_Load5 : ToWorkspace  VariableName=Q_Load5  SampleTime=sim_config.Tsample
  To Workspace_Q_Load50 : ToWorkspace  VariableName=Q_Load50  SampleTime=sim_config.Tsample
  To Workspace_Q_Load51 : ToWorkspace  VariableName=Q_Load51  SampleTime=sim_config.Tsample
  To Workspace_Q_Load52 : ToWorkspace  VariableName=Q_Load52  SampleTime=sim_config.Tsample
  To Workspace_Q_Load53 : ToWorkspace  VariableName=Q_Load53  SampleTime=sim_config.Tsample
  To Workspace_Q_Load54 : ToWorkspace  VariableName=Q_Load54  SampleTime=sim_config.Tsample
  To Workspace_Q_Load55 : ToWorkspace  VariableName=Q_Load55  SampleTime=sim_config.Tsample
  To Workspace_Q_Load56 : ToWorkspace  VariableName=Q_Load56  SampleTime=sim_config.Tsample
  To Workspace_Q_Load57 : ToWorkspace  VariableName=Q_Load57  SampleTime=sim_config.Tsample
  To Workspace_Q_Load58 : ToWorkspace  VariableName=Q_Load58  SampleTime=sim_config.Tsample
  To Workspace_Q_Load59 : ToWorkspace  VariableName=Q_Load59  SampleTime=sim_config.Tsample
  To Workspace_Q_Load6 : ToWorkspace  VariableName=Q_Load6  SampleTime=sim_config.Tsample
  To Workspace_Q_Load60 : ToWorkspace  VariableName=Q_Load60  SampleTime=sim_config.Tsample
  To Workspace_Q_Load61 : ToWorkspace  VariableName=Q_Load61  SampleTime=sim_config.Tsample
  To Workspace_Q_Load62 : ToWorkspace  VariableName=Q_Load62  SampleTime=sim_config.Tsample
  To Workspace_Q_Load63 : ToWorkspace  VariableName=Q_Load63  SampleTime=sim_config.Tsample
  To Workspace_Q_Load64 : ToWorkspace  VariableName=Q_Load64  SampleTime=sim_config.Tsample
  To Workspace_Q_Load65 : ToWorkspace  VariableName=Q_Load65  SampleTime=sim_config.Tsample
  To Workspace_Q_Load66 : ToWorkspace  VariableName=Q_Load66  SampleTime=sim_config.Tsample
  To Workspace_Q_Load67 : ToWorkspace  VariableName=Q_Load67  SampleTime=sim_config.Tsample
  To Workspace_Q_Load68 : ToWorkspace  VariableName=Q_Load68  SampleTime=sim_config.Tsample
  To Workspace_Q_Load69 : ToWorkspace  VariableName=Q_Load69  SampleTime=sim_config.Tsample
  To Workspace_Q_Load7 : ToWorkspace  VariableName=Q_Load7  SampleTime=sim_config.Tsample
  To Workspace_Q_Load70 : ToWorkspace  VariableName=Q_Load70  SampleTime=sim_config.Tsample
  To Workspace_Q_Load71 : ToWorkspace  VariableName=Q_Load71  SampleTime=sim_config.Tsample
  To Workspace_Q_Load72 : ToWorkspace  VariableName=Q_Load72  SampleTime=sim_config.Tsample
  To Workspace_Q_Load73 : ToWorkspace  VariableName=Q_Load73  SampleTime=sim_config.Tsample
  To Workspace_Q_Load74 : ToWorkspace  VariableName=Q_Load74  SampleTime=sim_config.Tsample
  To Workspace_Q_Load75 : ToWorkspace  VariableName=Q_Load75  SampleTime=sim_config.Tsample
  To Workspace_Q_Load76 : ToWorkspace  VariableName=Q_Load76  SampleTime=sim_config.Tsample
  To Workspace_Q_Load77 : ToWorkspace  VariableName=Q_Load77  SampleTime=sim_config.Tsample
  To Workspace_Q_Load78 : ToWorkspace  VariableName=Q_Load78  SampleTime=sim_config.Tsample
  To Workspace_Q_Load79 : ToWorkspace  VariableName=Q_Load79  SampleTime=sim_config.Tsample
  To Workspace_Q_Load8 : ToWorkspace  VariableName=Q_Load8  SampleTime=sim_config.Tsample
  To Workspace_Q_Load80 : ToWorkspace  VariableName=Q_Load80  SampleTime=sim_config.Tsample
  To Workspace_Q_Load81 : ToWorkspace  VariableName=Q_Load81  SampleTime=sim_config.Tsample
  To Workspace_Q_Load82 : ToWorkspace  VariableName=Q_Load82  SampleTime=sim_config.Tsample
  To Workspace_Q_Load83 : ToWorkspace  VariableName=Q_Load83  SampleTime=sim_config.Tsample
  To Workspace_Q_Load84 : ToWorkspace  VariableName=Q_Load84  SampleTime=sim_config.Tsample
  To Workspace_Q_Load85 : ToWorkspace  VariableName=Q_Load85  SampleTime=sim_config.Tsample
  To Workspace_Q_Load86 : ToWorkspace  VariableName=Q_Load86  SampleTime=sim_config.Tsample
  To Workspace_Q_Load87 : ToWorkspace  VariableName=Q_Load87  SampleTime=sim_config.Tsample
  To Workspace_Q_Load88 : ToWorkspace  VariableName=Q_Load88  SampleTime=sim_config.Tsample
  To Workspace_Q_Load89 : ToWorkspace  VariableName=Q_Load89  SampleTime=sim_config.Tsample
  To Workspace_Q_Load9 : ToWorkspace  VariableName=Q_Load9  SampleTime=sim_config.Tsample
  To Workspace_Q_Load90 : ToWorkspace  VariableName=Q_Load90  SampleTime=sim_config.Tsample
  To Workspace_Q_Load91 : ToWorkspace  VariableName=Q_Load91  SampleTime=sim_config.Tsample
  To Workspace_Q_SG1 : ToWorkspace  VariableName=Q_SG1  SampleTime=sim_config.Tsample
  To Workspace_Q_SG10 : ToWorkspace  VariableName=Q_SG10  SampleTime=sim_config.Tsample
  To Workspace_Q_SG11 : ToWorkspace  VariableName=Q_SG11  SampleTime=sim_config.Tsample
  To Workspace_Q_SG12 : ToWorkspace  VariableName=Q_SG12  SampleTime=sim_config.Tsample
  To Workspace_Q_SG13 : ToWorkspace  VariableName=Q_SG13  SampleTime=sim_config.Tsample
  To Workspace_Q_SG14 : ToWorkspace  VariableName=Q_SG14  SampleTime=sim_config.Tsample
  To Workspace_Q_SG15 : ToWorkspace  VariableName=Q_SG15  SampleTime=sim_config.Tsample
  To Workspace_Q_SG16 : ToWorkspace  VariableName=Q_SG16  SampleTime=sim_config.Tsample
  To Workspace_Q_SG17 : ToWorkspace  VariableName=Q_SG17  SampleTime=sim_config.Tsample
  To Workspace_Q_SG18 : ToWorkspace  VariableName=Q_SG18  SampleTime=sim_config.Tsample
  To Workspace_Q_SG19 : ToWorkspace  VariableName=Q_SG19  SampleTime=sim_config.Tsample
  To Workspace_Q_SG2 : ToWorkspace  VariableName=Q_SG2  SampleTime=sim_config.Tsample
  To Workspace_Q_SG20 : ToWorkspace  VariableName=Q_SG20  SampleTime=sim_config.Tsample
  To Workspace_Q_SG21 : ToWorkspace  VariableName=Q_SG21  SampleTime=sim_config.Tsample
  To Workspace_Q_SG22 : ToWorkspace  VariableName=Q_SG22  SampleTime=sim_config.Tsample
  To Workspace_Q_SG23 : ToWorkspace  VariableName=Q_SG23  SampleTime=sim_config.Tsample
  To Workspace_Q_SG24 : ToWorkspace  VariableName=Q_SG24  SampleTime=sim_config.Tsample
  To Workspace_Q_SG25 : ToWorkspace  VariableName=Q_SG25  SampleTime=sim_config.Tsample
  To Workspace_Q_SG26 : ToWorkspace  VariableName=Q_SG26  SampleTime=sim_config.Tsample
  To Workspace_Q_SG3 : ToWorkspace  VariableName=Q_SG3  SampleTime=sim_config.Tsample
  To Workspace_Q_SG4 : ToWorkspace  VariableName=Q_SG4  SampleTime=sim_config.Tsample
  To Workspace_Q_SG5 : ToWorkspace  VariableName=Q_SG5  SampleTime=sim_config.Tsample
  To Workspace_Q_SG6 : ToWorkspace  VariableName=Q_SG6  SampleTime=sim_config.Tsample
  To Workspace_Q_SG7 : ToWorkspace  VariableName=Q_SG7  SampleTime=sim_config.Tsample
  To Workspace_Q_SG8 : ToWorkspace  VariableName=Q_SG8  SampleTime=sim_config.Tsample
  To Workspace_Q_SG9 : ToWorkspace  VariableName=Q_SG9  SampleTime=sim_config.Tsample
  To Workspace_Q_VSC1 : ToWorkspace  VariableName=Q_VSC1  SampleTime=sim_config.Tsample
  To Workspace_Q_VSC10 : ToWorkspace  VariableName=Q_VSC10  SampleTime=sim_config.Tsample
  To Workspace_Q_VSC11 : ToWorkspace  VariableName=Q_VSC11  SampleTime=sim_config.Tsample
  To Workspace_Q_VSC12 : ToWorkspace  VariableName=Q_VSC12  SampleTime=sim_config.Tsample
  To Workspace_Q_VSC13 : ToWorkspace  VariableName=Q_VSC13  SampleTime=sim_config.Tsample
  To Workspace_Q_VSC14 : ToWorkspace  VariableName=Q_VSC14  SampleTime=sim_config.Tsample
  To Workspace_Q_VSC15 : ToWorkspace  VariableName=Q_VSC15  SampleTime=sim_config.Tsample
  To Workspace_Q_VSC16 : ToWorkspace  VariableName=Q_VSC16  SampleTime=sim_config.Tsample
  To Workspace_Q_VSC17 : ToWorkspace  VariableName=Q_VSC17  SampleTime=sim_config.Tsample
  To Workspace_Q_VSC18 : ToWorkspace  VariableName=Q_VSC18  SampleTime=sim_config.Tsample
  To Workspace_Q_VSC19 : ToWorkspace  VariableName=Q_VSC19  SampleTime=sim_config.Tsample
  To Workspace_Q_VSC2 : ToWorkspace  VariableName=Q_VSC2  SampleTime=sim_config.Tsample
  To Workspace_Q_VSC20 : ToWorkspace  VariableName=Q_VSC20  SampleTime=sim_config.Tsample
  To Workspace_Q_VSC3 : ToWorkspace  VariableName=Q_VSC3  SampleTime=sim_config.Tsample
  To Workspace_Q_VSC4 : ToWorkspace  VariableName=Q_VSC4  SampleTime=sim_config.Tsample
  To Workspace_Q_VSC5 : ToWorkspace  VariableName=Q_VSC5  SampleTime=sim_config.Tsample
  To Workspace_Q_VSC6 : ToWorkspace  VariableName=Q_VSC6  SampleTime=sim_config.Tsample
  To Workspace_Q_VSC7 : ToWorkspace  VariableName=Q_VSC7  SampleTime=sim_config.Tsample
  To Workspace_Q_VSC8 : ToWorkspace  VariableName=Q_VSC8  SampleTime=sim_config.Tsample
  To Workspace_Q_VSC9 : ToWorkspace  VariableName=Q_VSC9  SampleTime=sim_config.Tsample
  VSC-1 : myLibrary/GFOL_RL  T_VSC_global=T_VSC  initVSC_global=init_VSC  num=1
  VSC-10 : myLibrary/GFOL_RL  T_VSC_global=T_VSC  initVSC_global=init_VSC  num=10
  VSC-11 : myLibrary/GFOR  T_VSC_global=T_VSC  initVSC_global=init_VSC  num=11
  VSC-12 : myLibrary/GFOR  T_VSC_global=T_VSC  initVSC_global=init_VSC  num=12
  VSC-13 : myLibrary/GFOR  T_VSC_global=T_VSC  initVSC_global=init_VSC  num=13
  VSC-14 : myLibrary/GFOR  T_VSC_global=T_VSC  initVSC_global=init_VSC  num=14
  VSC-15 : myLibrary/GFOR  T_VSC_global=T_VSC  initVSC_global=init_VSC  num=15
  VSC-16 : myLibrary/GFOR  T_VSC_global=T_VSC  initVSC_global=init_VSC  num=16
  VSC-17 : myLibrary/GFOR  T_VSC_global=T_VSC  initVSC_global=init_VSC  num=17
  VSC-18 : myLibrary/GFOR  T_VSC_global=T_VSC  initVSC_global=init_VSC  num=18
  VSC-19 : myLibrary/GFOR  T_VSC_global=T_VSC  initVSC_global=init_VSC  num=19
  VSC-2 : myLibrary/GFOL_RL  T_VSC_global=T_VSC  initVSC_global=init_VSC  num=2
  VSC-20 : myLibrary/GFOR  T_VSC_global=T_VSC  initVSC_global=init_VSC  num=20
  VSC-3 : myLibrary/GFOL_RL  T_VSC_global=T_VSC  initVSC_global=init_VSC  num=3
  VSC-4 : myLibrary/GFOL_RL  T_VSC_global=T_VSC  initVSC_global=init_VSC  num=4
  VSC-5 : myLibrary/GFOL_RL  T_VSC_global=T_VSC  initVSC_global=init_VSC  num=5
  VSC-6 : myLibrary/GFOL_RL  T_VSC_global=T_VSC  initVSC_global=init_VSC  num=6
  VSC-7 : myLibrary/GFOL_RL  T_VSC_global=T_VSC  initVSC_global=init_VSC  num=7
  VSC-8 : myLibrary/GFOL_RL  T_VSC_global=T_VSC  initVSC_global=init_VSC  num=8
  VSC-9 : myLibrary/GFOL_RL  T_VSC_global=T_VSC  initVSC_global=init_VSC  num=9
  clock : Clock
  display : Display
  mtx{,1..112} (113 alike) : Product  Multiplication=Matrix(*)
  powergui : spspowerguiLib/powergui  Priority=1  SimulationMode=Discrete  SampleTime=sim_config.Ts  frequency=60  Iterations=50  frequencyindice=60  Pbase=100e6  ErrMax=1e-4  UnitsV=kV  UnitsW=MW  buscounter=0  FunctionMessages=off  echomessages=off  EnableUseOfTLC=off  CurrentSourceSwitches=off  DisableSnubberDevices=off  DisableRonSwitches=off  DisableVfSwitches=off  DisplayEquations=off  AutomaticDiscreteSolvers=off  SolverType=Tustin/Backward Euler (TBE)  Interpol=off  ExternalGateDelay=off  methode=off  Ts=100  x0status=blocks  SPID=on  SwTol=0  HookPort=off  NonlinearTolerance=1e-4  nMaxIteration=100  ContinueOnMaxIteration=off  RestoreLinks=warning  ResistiveCurrentMeasurement=off  Frange=[0:2:500]  Ylog=off  Xlog=on  ShowGrid=off  save=off  variable=ZData  structure=0  ZoomFFT=off  StartTime=0.0  cycles=1  DisplayStyle=1  fundamental=60  FreqAxis=off  MaxFrequency=1000  frequencyindicesteady=1  RmsSteady=1  display=off
  qd{,1..249} (250 alike) : myLibrary/qd transform  SystemSampleTime=-1  VariantActivationTime=update diagram  Latency=0  AutoFrameSizeCalculation=off
  tag scope: V_fn_100=global, V_fn_101=global, V_fn_102=global, V_fn_103=global, V_fn_104=global, V_fn_105=global, V_fn_106=global, V_fn_107=global, V_fn_108=global, V_fn_109=global, V_fn_110=global, V_fn_112=global, V_fn_113=global, V_fn_114=global, V_fn_115=global, V_fn_117=global, V_fn_118=global, V_fn_11=global, V_fn_12=global, V_fn_13=global, V_fn_14=global, V_fn_15=global, V_fn_16=global, V_fn_17=global, V_fn_18=global, V_fn_19=global, V_fn_1=global, V_fn_20=global, V_fn_21=global, V_fn_22=global, V_fn_23=global, V_fn_24=global, V_fn_25=global, V_fn_26=global, V_fn_27=global, V_fn_28=global, V_fn_29=global, V_fn_2=global, V_fn_30=global, V_fn_31=global, V_fn_32=global, V_fn_33=global, V_fn_34=global, V_fn_35=global, V_fn_36=global, V_fn_37=global, V_fn_38=global, V_fn_39=global, V_fn_3=global, V_fn_40=global, V_fn_41=global, V_fn_42=global, V_fn_43=global, V_fn_44=global, V_fn_45=global, V_fn_46=global, V_fn_47=global, V_fn_48=global, V_fn_49=global, V_fn_4=global, V_fn_50=global, V_fn_51=global, V_fn_52=global, V_fn_53=global, V_fn_54=global, V_fn_55=global, V_fn_56=global, V_fn_57=global, V_fn_58=global, V_fn_59=global, V_fn_5=global, V_fn_60=global, V_fn_61=global, V_fn_62=global, V_fn_63=global, V_fn_64=global, V_fn_65=global, V_fn_66=global, V_fn_67=global, V_fn_68=global, V_fn_69=global, V_fn_6=global, V_fn_70=global, V_fn_71=global, V_fn_72=global, V_fn_73=global, V_fn_74=global, V_fn_75=global, V_fn_76=global, V_fn_77=global, V_fn_78=global, V_fn_79=global, V_fn_7=global, V_fn_80=global, V_fn_81=global, V_fn_82=global, V_fn_83=global, V_fn_84=global, V_fn_85=global, V_fn_86=global, V_fn_88=global, V_fn_89=global, V_fn_8=global, V_fn_90=global, V_fn_91=global, V_fn_92=global, V_fn_93=global, V_fn_94=global, V_fn_95=global, V_fn_96=global, V_fn_97=global, V_fn_98=global, V_fn_99=global, angle_ref=global
  wires:
  clock/1 -> display/1
  [theta_SG10] -> [angle_ref]
  [V_ll_1] -> Scope/1
  [V_ll_2] -> Scope1/1
  [V_ll_3] -> Scope2/1
  [V_ll_4] -> Scope3/1
  [V_ll_5] -> Scope4/1
  [V_ll_6] -> Scope5/1
  [V_ll_7] -> Scope6/1
  [V_ll_8] -> Scope7/1
  [V_ll_11] -> Scope8/1
  [V_ll_12] -> Scope9/1
  [V_ll_13] -> Scope10/1
  [V_ll_14] -> Scope11/1
  [V_ll_15] -> Scope12/1
  [V_ll_16] -> Scope13/1
  [V_ll_17] -> Scope14/1
  [V_ll_18] -> Scope15/1
  [V_ll_19] -> Scope16/1
  [V_ll_20] -> Scope17/1
  [V_ll_21] -> Scope18/1
  [V_ll_22] -> Scope19/1
  [V_ll_23] -> Scope20/1
  [V_ll_24] -> Scope21/1
  [V_ll_25] -> Scope22/1
  [V_ll_26] -> Scope23/1
  [V_ll_27] -> Scope24/1
  [V_ll_28] -> Scope25/1
  [V_ll_29] -> Scope26/1
  [V_ll_30] -> Scope27/1
  [V_ll_31] -> Scope28/1
  [V_ll_32] -> Scope29/1
  [V_ll_33] -> Scope30/1
  [V_ll_34] -> Scope31/1
  [V_ll_35] -> Scope32/1
  [V_ll_36] -> Scope33/1
  [V_ll_37] -> Scope34/1
  [V_ll_38] -> Scope35/1
  [V_ll_39] -> Scope36/1
  [V_ll_40] -> Scope37/1
  [V_ll_41] -> Scope38/1
  [V_ll_42] -> Scope39/1
  [V_ll_43] -> Scope40/1
  [V_ll_44] -> Scope41/1
  [V_ll_45] -> Scope42/1
  [V_ll_46] -> Scope43/1
  [V_ll_47] -> Scope44/1
  [V_ll_48] -> Scope45/1
  [V_ll_49] -> Scope46/1
  [V_ll_50] -> Scope47/1
  [V_ll_51] -> Scope48/1
  [V_ll_52] -> Scope49/1
  [V_ll_53] -> Scope50/1
  [V_ll_54] -> Scope51/1
  [V_ll_55] -> Scope52/1
  [V_ll_56] -> Scope53/1
  [V_ll_57] -> Scope54/1
  [V_ll_58] -> Scope55/1
  [V_ll_59] -> Scope56/1
  [V_ll_60] -> Scope57/1
  [V_ll_61] -> Scope58/1
  [V_ll_62] -> Scope59/1
  [V_ll_63] -> Scope60/1
  [V_ll_64] -> Scope61/1
  [V_ll_65] -> Scope62/1
  [V_ll_66] -> Scope63/1
  [V_ll_67] -> Scope64/1
  [V_ll_68] -> Scope65/1
  [V_ll_69] -> Scope66/1
  [V_ll_70] -> Scope67/1
  [V_ll_71] -> Scope68/1
  [V_ll_72] -> Scope69/1
  [V_ll_73] -> Scope70/1
  [V_ll_74] -> Scope71/1
  [V_ll_75] -> Scope72/1
  [V_ll_76] -> Scope73/1
  [V_ll_77] -> Scope74/1
  [V_ll_78] -> Scope75/1
  [V_ll_79] -> Scope76/1
  [V_ll_80] -> Scope77/1
  [V_ll_81] -> Scope78/1
  [V_ll_82] -> Scope79/1
  [V_ll_83] -> Scope80/1
  [V_ll_84] -> Scope81/1
  [V_ll_85] -> Scope82/1
  [V_ll_86] -> Scope83/1
  [V_ll_88] -> Scope84/1
  [V_ll_89] -> Scope85/1
  [V_ll_90] -> Scope86/1
  [V_ll_91] -> Scope87/1
  [V_ll_92] -> Scope88/1
  [V_ll_93] -> Scope89/1
  [V_ll_94] -> Scope90/1
  [V_ll_95] -> Scope91/1
  [V_ll_96] -> Scope92/1
  [V_ll_97] -> Scope93/1
  [V_ll_98] -> Scope94/1
  [V_ll_99] -> Scope95/1
  [V_ll_100] -> Scope96/1
  [V_ll_101] -> Scope97/1
  [V_ll_102] -> Scope98/1
  [V_ll_103] -> Scope99/1
  [V_ll_104] -> Scope100/1
  [V_ll_105] -> Scope101/1
  [V_ll_106] -> Scope102/1
  [V_ll_107] -> Scope103/1
  [V_ll_108] -> Scope104/1
  [V_ll_109] -> Scope105/1
  [V_ll_110] -> Scope106/1
  [V_ll_112] -> Scope107/1
  [V_ll_113] -> Scope108/1
  [V_ll_114] -> Scope109/1
  [V_ll_115] -> Scope110/1
  [V_ll_117] -> Scope111/1
  [V_ll_118] -> Scope112/1
  [V_ll_1] -> Demux/1
  Demux/1 -> Mux/1
  Demux/2 -> Mux/2
  Mux/1 -> mtx/2
  Constant/1 -> mtx/1
  mtx/1 -> [V_fn_1], Scope113/1
  [V_ll_2] -> Demux1/1
  Demux1/1 -> Mux1/1
  Demux1/2 -> Mux1/2
  Mux1/1 -> mtx1/2
  Constant1/1 -> mtx1/1
  mtx1/1 -> [V_fn_2], Scope114/1
  [V_ll_3] -> Demux2/1
  Demux2/1 -> Mux2/1
  Demux2/2 -> Mux2/2
  Mux2/1 -> mtx2/2
  Constant2/1 -> mtx2/1
  mtx2/1 -> [V_fn_3], Scope115/1
  [V_ll_4] -> Demux3/1
  Demux3/1 -> Mux3/1
  Demux3/2 -> Mux3/2
  Mux3/1 -> mtx3/2
  Constant3/1 -> mtx3/1
  mtx3/1 -> [V_fn_4], Scope116/1
  [V_ll_5] -> Demux4/1
  Demux4/1 -> Mux4/1
  Demux4/2 -> Mux4/2
  Mux4/1 -> mtx4/2
  Constant4/1 -> mtx4/1
  mtx4/1 -> [V_fn_5], Scope117/1
  [V_ll_6] -> Demux5/1
  Demux5/1 -> Mux5/1
  Demux5/2 -> Mux5/2
  Mux5/1 -> mtx5/2
  Constant5/1 -> mtx5/1
  mtx5/1 -> [V_fn_6], Scope118/1
  [V_ll_7] -> Demux6/1
  Demux6/1 -> Mux6/1
  Demux6/2 -> Mux6/2
  Mux6/1 -> mtx6/2
  Constant6/1 -> mtx6/1
  mtx6/1 -> [V_fn_7], Scope119/1
  [V_ll_8] -> Demux7/1
  Demux7/1 -> Mux7/1
  Demux7/2 -> Mux7/2
  Mux7/1 -> mtx7/2
  Constant7/1 -> mtx7/1
  mtx7/1 -> [V_fn_8], Scope120/1
  [V_ll_11] -> Demux8/1
  Demux8/1 -> Mux8/1
  Demux8/2 -> Mux8/2
  Mux8/1 -> mtx8/2
  Constant8/1 -> mtx8/1
  mtx8/1 -> [V_fn_11], Scope121/1
  [V_ll_12] -> Demux9/1
  Demux9/1 -> Mux9/1
  Demux9/2 -> Mux9/2
  Mux9/1 -> mtx9/2
  Constant9/1 -> mtx9/1
  mtx9/1 -> [V_fn_12], Scope122/1
  [V_ll_13] -> Demux10/1
  Demux10/1 -> Mux10/1
  Demux10/2 -> Mux10/2
  Mux10/1 -> mtx10/2
  Constant10/1 -> mtx10/1
  mtx10/1 -> [V_fn_13], Scope123/1
  [V_ll_14] -> Demux11/1
  Demux11/1 -> Mux11/1
  Demux11/2 -> Mux11/2
  Mux11/1 -> mtx11/2
  Constant11/1 -> mtx11/1
  mtx11/1 -> [V_fn_14], Scope124/1
  [V_ll_15] -> Demux12/1
  Demux12/1 -> Mux12/1
  Demux12/2 -> Mux12/2
  Mux12/1 -> mtx12/2
  Constant12/1 -> mtx12/1
  mtx12/1 -> [V_fn_15], Scope125/1
  [V_ll_16] -> Demux13/1
  Demux13/1 -> Mux13/1
  Demux13/2 -> Mux13/2
  Mux13/1 -> mtx13/2
  Constant13/1 -> mtx13/1
  mtx13/1 -> [V_fn_16], Scope126/1
  [V_ll_17] -> Demux14/1
  Demux14/1 -> Mux14/1
  Demux14/2 -> Mux14/2
  Mux14/1 -> mtx14/2
  Constant14/1 -> mtx14/1
  mtx14/1 -> [V_fn_17], Scope127/1
  [V_ll_18] -> Demux15/1
  Demux15/1 -> Mux15/1
  Demux15/2 -> Mux15/2
  Mux15/1 -> mtx15/2
  Constant15/1 -> mtx15/1
  mtx15/1 -> [V_fn_18], Scope128/1
  [V_ll_19] -> Demux16/1
  Demux16/1 -> Mux16/1
  Demux16/2 -> Mux16/2
  Mux16/1 -> mtx16/2
  Constant16/1 -> mtx16/1
  mtx16/1 -> [V_fn_19], Scope129/1
  [V_ll_20] -> Demux17/1
  Demux17/1 -> Mux17/1
  Demux17/2 -> Mux17/2
  Mux17/1 -> mtx17/2
  Constant17/1 -> mtx17/1
  mtx17/1 -> [V_fn_20], Scope130/1
  [V_ll_21] -> Demux18/1
  Demux18/1 -> Mux18/1
  Demux18/2 -> Mux18/2
  Mux18/1 -> mtx18/2
  Constant18/1 -> mtx18/1
  mtx18/1 -> [V_fn_21], Scope131/1
  [V_ll_22] -> Demux19/1
  Demux19/1 -> Mux19/1
  Demux19/2 -> Mux19/2
  Mux19/1 -> mtx19/2
  Constant19/1 -> mtx19/1
  mtx19/1 -> [V_fn_22], Scope132/1
  [V_ll_23] -> Demux20/1
  Demux20/1 -> Mux20/1
  Demux20/2 -> Mux20/2
  Mux20/1 -> mtx20/2
  Constant20/1 -> mtx20/1
  mtx20/1 -> [V_fn_23], Scope133/1
  [V_ll_24] -> Demux21/1
  Demux21/1 -> Mux21/1
  Demux21/2 -> Mux21/2
  Mux21/1 -> mtx21/2
  Constant21/1 -> mtx21/1
  mtx21/1 -> [V_fn_24], Scope134/1
  [V_ll_25] -> Demux22/1
  Demux22/1 -> Mux22/1
  Demux22/2 -> Mux22/2
  Mux22/1 -> mtx22/2
  Constant22/1 -> mtx22/1
  mtx22/1 -> [V_fn_25], Scope135/1
  [V_ll_26] -> Demux23/1
  Demux23/1 -> Mux23/1
  Demux23/2 -> Mux23/2
  Mux23/1 -> mtx23/2
  Constant23/1 -> mtx23/1
  mtx23/1 -> [V_fn_26], Scope136/1
  [V_ll_27] -> Demux24/1
  Demux24/1 -> Mux24/1
  Demux24/2 -> Mux24/2
  Mux24/1 -> mtx24/2
  Constant24/1 -> mtx24/1
  mtx24/1 -> [V_fn_27], Scope137/1
  [V_ll_28] -> Demux25/1
  Demux25/1 -> Mux25/1
  Demux25/2 -> Mux25/2
  Mux25/1 -> mtx25/2
  Constant25/1 -> mtx25/1
  mtx25/1 -> [V_fn_28], Scope138/1
  [V_ll_29] -> Demux26/1
  Demux26/1 -> Mux26/1
  Demux26/2 -> Mux26/2
  Mux26/1 -> mtx26/2
  Constant26/1 -> mtx26/1
  mtx26/1 -> [V_fn_29], Scope139/1
  [V_ll_30] -> Demux27/1
  Demux27/1 -> Mux27/1
  Demux27/2 -> Mux27/2
  Mux27/1 -> mtx27/2
  Constant27/1 -> mtx27/1
  mtx27/1 -> [V_fn_30], Scope140/1
  [V_ll_31] -> Demux28/1
  Demux28/1 -> Mux28/1
  Demux28/2 -> Mux28/2
  Mux28/1 -> mtx28/2
  Constant28/1 -> mtx28/1
  mtx28/1 -> [V_fn_31], Scope141/1
  [V_ll_32] -> Demux29/1
  Demux29/1 -> Mux29/1
  Demux29/2 -> Mux29/2
  Mux29/1 -> mtx29/2
  Constant29/1 -> mtx29/1
  mtx29/1 -> [V_fn_32], Scope142/1
  [V_ll_33] -> Demux30/1
  Demux30/1 -> Mux30/1
  Demux30/2 -> Mux30/2
  Mux30/1 -> mtx30/2
  Constant30/1 -> mtx30/1
  mtx30/1 -> [V_fn_33], Scope143/1
  [V_ll_34] -> Demux31/1
  Demux31/1 -> Mux31/1
  Demux31/2 -> Mux31/2
  Mux31/1 -> mtx31/2
  Constant31/1 -> mtx31/1
  mtx31/1 -> [V_fn_34], Scope144/1
  [V_ll_35] -> Demux32/1
  Demux32/1 -> Mux32/1
  Demux32/2 -> Mux32/2
  Mux32/1 -> mtx32/2
  Constant32/1 -> mtx32/1
  mtx32/1 -> [V_fn_35], Scope145/1
  [V_ll_36] -> Demux33/1
  Demux33/1 -> Mux33/1
  Demux33/2 -> Mux33/2
  Mux33/1 -> mtx33/2
  Constant33/1 -> mtx33/1
  mtx33/1 -> [V_fn_36], Scope146/1
  [V_ll_37] -> Demux34/1
  Demux34/1 -> Mux34/1
  Demux34/2 -> Mux34/2
  Mux34/1 -> mtx34/2
  Constant34/1 -> mtx34/1
  mtx34/1 -> [V_fn_37], Scope147/1
  [V_ll_38] -> Demux35/1
  Demux35/1 -> Mux35/1
  Demux35/2 -> Mux35/2
  Mux35/1 -> mtx35/2
  Constant35/1 -> mtx35/1
  mtx35/1 -> [V_fn_38], Scope148/1
  [V_ll_39] -> Demux36/1
  Demux36/1 -> Mux36/1
  Demux36/2 -> Mux36/2
  Mux36/1 -> mtx36/2
  Constant36/1 -> mtx36/1
  mtx36/1 -> [V_fn_39], Scope149/1
  [V_ll_40] -> Demux37/1
  Demux37/1 -> Mux37/1
  Demux37/2 -> Mux37/2
  Mux37/1 -> mtx37/2
  Constant37/1 -> mtx37/1
  mtx37/1 -> [V_fn_40], Scope150/1
  [V_ll_41] -> Demux38/1
  Demux38/1 -> Mux38/1
  Demux38/2 -> Mux38/2
  Mux38/1 -> mtx38/2
  Constant38/1 -> mtx38/1
  mtx38/1 -> [V_fn_41], Scope151/1
  [V_ll_42] -> Demux39/1
  Demux39/1 -> Mux39/1
  Demux39/2 -> Mux39/2
  Mux39/1 -> mtx39/2
  Constant39/1 -> mtx39/1
  mtx39/1 -> [V_fn_42], Scope152/1
  [V_ll_43] -> Demux40/1
  Demux40/1 -> Mux40/1
  Demux40/2 -> Mux40/2
  Mux40/1 -> mtx40/2
  Constant40/1 -> mtx40/1
  mtx40/1 -> [V_fn_43], Scope153/1
  [V_ll_44] -> Demux41/1
  Demux41/1 -> Mux41/1
  Demux41/2 -> Mux41/2
  Mux41/1 -> mtx41/2
  Constant41/1 -> mtx41/1
  mtx41/1 -> [V_fn_44], Scope154/1
  [V_ll_45] -> Demux42/1
  Demux42/1 -> Mux42/1
  Demux42/2 -> Mux42/2
  Mux42/1 -> mtx42/2
  Constant42/1 -> mtx42/1
  mtx42/1 -> [V_fn_45], Scope155/1
  [V_ll_46] -> Demux43/1
  Demux43/1 -> Mux43/1
  Demux43/2 -> Mux43/2
  Mux43/1 -> mtx43/2
  Constant43/1 -> mtx43/1
  mtx43/1 -> [V_fn_46], Scope156/1
  [V_ll_47] -> Demux44/1
  Demux44/1 -> Mux44/1
  Demux44/2 -> Mux44/2
  Mux44/1 -> mtx44/2
  Constant44/1 -> mtx44/1
  mtx44/1 -> [V_fn_47], Scope157/1
  [V_ll_48] -> Demux45/1
  Demux45/1 -> Mux45/1
  Demux45/2 -> Mux45/2
  Mux45/1 -> mtx45/2
  Constant45/1 -> mtx45/1
  mtx45/1 -> [V_fn_48], Scope158/1
  [V_ll_49] -> Demux46/1
  Demux46/1 -> Mux46/1
  Demux46/2 -> Mux46/2
  Mux46/1 -> mtx46/2
  Constant46/1 -> mtx46/1
  mtx46/1 -> [V_fn_49], Scope159/1
  [V_ll_50] -> Demux47/1
  Demux47/1 -> Mux47/1
  Demux47/2 -> Mux47/2
  Mux47/1 -> mtx47/2
  Constant47/1 -> mtx47/1
  mtx47/1 -> [V_fn_50], Scope160/1
  [V_ll_51] -> Demux48/1
  Demux48/1 -> Mux48/1
  Demux48/2 -> Mux48/2
  Mux48/1 -> mtx48/2
  Constant48/1 -> mtx48/1
  mtx48/1 -> [V_fn_51], Scope161/1
  [V_ll_52] -> Demux49/1
  Demux49/1 -> Mux49/1
  Demux49/2 -> Mux49/2
  Mux49/1 -> mtx49/2
  Constant49/1 -> mtx49/1
  mtx49/1 -> [V_fn_52], Scope162/1
  [V_ll_53] -> Demux50/1
  Demux50/1 -> Mux50/1
  Demux50/2 -> Mux50/2
  Mux50/1 -> mtx50/2
  Constant50/1 -> mtx50/1
  mtx50/1 -> [V_fn_53], Scope163/1
  [V_ll_54] -> Demux51/1
  Demux51/1 -> Mux51/1
  Demux51/2 -> Mux51/2
  Mux51/1 -> mtx51/2
  Constant51/1 -> mtx51/1
  mtx51/1 -> [V_fn_54], Scope164/1
  [V_ll_55] -> Demux52/1
  Demux52/1 -> Mux52/1
  Demux52/2 -> Mux52/2
  Mux52/1 -> mtx52/2
  Constant52/1 -> mtx52/1
  mtx52/1 -> [V_fn_55], Scope165/1
  [V_ll_56] -> Demux53/1
  Demux53/1 -> Mux53/1
  Demux53/2 -> Mux53/2
  Mux53/1 -> mtx53/2
  Constant53/1 -> mtx53/1
  mtx53/1 -> [V_fn_56], Scope166/1
  [V_ll_57] -> Demux54/1
  Demux54/1 -> Mux54/1
  Demux54/2 -> Mux54/2
  Mux54/1 -> mtx54/2
  Constant54/1 -> mtx54/1
  mtx54/1 -> [V_fn_57], Scope167/1
  [V_ll_58] -> Demux55/1
  Demux55/1 -> Mux55/1
  Demux55/2 -> Mux55/2
  Mux55/1 -> mtx55/2
  Constant55/1 -> mtx55/1
  mtx55/1 -> [V_fn_58], Scope168/1
  [V_ll_59] -> Demux56/1
  Demux56/1 -> Mux56/1
  Demux56/2 -> Mux56/2
  Mux56/1 -> mtx56/2
  Constant56/1 -> mtx56/1
  mtx56/1 -> [V_fn_59], Scope169/1
  [V_ll_60] -> Demux57/1
  Demux57/1 -> Mux57/1
  Demux57/2 -> Mux57/2
  Mux57/1 -> mtx57/2
  Constant57/1 -> mtx57/1
  mtx57/1 -> [V_fn_60], Scope170/1
  [V_ll_61] -> Demux58/1
  Demux58/1 -> Mux58/1
  Demux58/2 -> Mux58/2
  Mux58/1 -> mtx58/2
  Constant58/1 -> mtx58/1
  mtx58/1 -> [V_fn_61], Scope171/1
  [V_ll_62] -> Demux59/1
  Demux59/1 -> Mux59/1
  Demux59/2 -> Mux59/2
  Mux59/1 -> mtx59/2
  Constant59/1 -> mtx59/1
  mtx59/1 -> [V_fn_62], Scope172/1
  [V_ll_63] -> Demux60/1
  Demux60/1 -> Mux60/1
  Demux60/2 -> Mux60/2
  Mux60/1 -> mtx60/2
  Constant60/1 -> mtx60/1
  mtx60/1 -> [V_fn_63], Scope173/1
  [V_ll_64] -> Demux61/1
  Demux61/1 -> Mux61/1
  Demux61/2 -> Mux61/2
  Mux61/1 -> mtx61/2
  Constant61/1 -> mtx61/1
  mtx61/1 -> [V_fn_64], Scope174/1
  [V_ll_65] -> Demux62/1
  Demux62/1 -> Mux62/1
  Demux62/2 -> Mux62/2
  Mux62/1 -> mtx62/2
  Constant62/1 -> mtx62/1
  mtx62/1 -> [V_fn_65], Scope175/1
  [V_ll_66] -> Demux63/1
  Demux63/1 -> Mux63/1
  Demux63/2 -> Mux63/2
  Mux63/1 -> mtx63/2
  Constant63/1 -> mtx63/1
  mtx63/1 -> [V_fn_66], Scope176/1
  [V_ll_67] -> Demux64/1
  Demux64/1 -> Mux64/1
  Demux64/2 -> Mux64/2
  Mux64/1 -> mtx64/2
  Constant64/1 -> mtx64/1
  mtx64/1 -> [V_fn_67], Scope177/1
  [V_ll_68] -> Demux65/1
  Demux65/1 -> Mux65/1
  Demux65/2 -> Mux65/2
  Mux65/1 -> mtx65/2
  Constant65/1 -> mtx65/1
  mtx65/1 -> [V_fn_68], Scope178/1
  [V_ll_69] -> Demux66/1
  Demux66/1 -> Mux66/1
  Demux66/2 -> Mux66/2
  Mux66/1 -> mtx66/2
  Constant66/1 -> mtx66/1
  mtx66/1 -> [V_fn_69], Scope179/1
  [V_ll_70] -> Demux67/1
  Demux67/1 -> Mux67/1
  Demux67/2 -> Mux67/2
  Mux67/1 -> mtx67/2
  Constant67/1 -> mtx67/1
  mtx67/1 -> [V_fn_70], Scope180/1
  [V_ll_71] -> Demux68/1
  Demux68/1 -> Mux68/1
  Demux68/2 -> Mux68/2
  Mux68/1 -> mtx68/2
  Constant68/1 -> mtx68/1
  mtx68/1 -> [V_fn_71], Scope181/1
  [V_ll_72] -> Demux69/1
  Demux69/1 -> Mux69/1
  Demux69/2 -> Mux69/2
  Mux69/1 -> mtx69/2
  Constant69/1 -> mtx69/1
  mtx69/1 -> [V_fn_72], Scope182/1
  [V_ll_73] -> Demux70/1
  Demux70/1 -> Mux70/1
  Demux70/2 -> Mux70/2
  Mux70/1 -> mtx70/2
  Constant70/1 -> mtx70/1
  mtx70/1 -> [V_fn_73], Scope183/1
  [V_ll_74] -> Demux71/1
  Demux71/1 -> Mux71/1
  Demux71/2 -> Mux71/2
  Mux71/1 -> mtx71/2
  Constant71/1 -> mtx71/1
  mtx71/1 -> [V_fn_74], Scope184/1
  [V_ll_75] -> Demux72/1
  Demux72/1 -> Mux72/1
  Demux72/2 -> Mux72/2
  Mux72/1 -> mtx72/2
  Constant72/1 -> mtx72/1
  mtx72/1 -> [V_fn_75], Scope185/1
  [V_ll_76] -> Demux73/1
  Demux73/1 -> Mux73/1
  Demux73/2 -> Mux73/2
  Mux73/1 -> mtx73/2
  Constant73/1 -> mtx73/1
  mtx73/1 -> [V_fn_76], Scope186/1
  [V_ll_77] -> Demux74/1
  Demux74/1 -> Mux74/1
  Demux74/2 -> Mux74/2
  Mux74/1 -> mtx74/2
  Constant74/1 -> mtx74/1
  mtx74/1 -> [V_fn_77], Scope187/1
  [V_ll_78] -> Demux75/1
  Demux75/1 -> Mux75/1
  Demux75/2 -> Mux75/2
  Mux75/1 -> mtx75/2
  Constant75/1 -> mtx75/1
  mtx75/1 -> [V_fn_78], Scope188/1
  [V_ll_79] -> Demux76/1
  Demux76/1 -> Mux76/1
  Demux76/2 -> Mux76/2
  Mux76/1 -> mtx76/2
  Constant76/1 -> mtx76/1
  mtx76/1 -> [V_fn_79], Scope189/1
  [V_ll_80] -> Demux77/1
  Demux77/1 -> Mux77/1
  Demux77/2 -> Mux77/2
  Mux77/1 -> mtx77/2
  Constant77/1 -> mtx77/1
  mtx77/1 -> [V_fn_80], Scope190/1
  [V_ll_81] -> Demux78/1
  Demux78/1 -> Mux78/1
  Demux78/2 -> Mux78/2
  Mux78/1 -> mtx78/2
  Constant78/1 -> mtx78/1
  mtx78/1 -> [V_fn_81], Scope191/1
  [V_ll_82] -> Demux79/1
  Demux79/1 -> Mux79/1
  Demux79/2 -> Mux79/2
  Mux79/1 -> mtx79/2
  Constant79/1 -> mtx79/1
  mtx79/1 -> [V_fn_82], Scope192/1
  [V_ll_83] -> Demux80/1
  Demux80/1 -> Mux80/1
  Demux80/2 -> Mux80/2
  Mux80/1 -> mtx80/2
  Constant80/1 -> mtx80/1
  mtx80/1 -> [V_fn_83], Scope193/1
  [V_ll_84] -> Demux81/1
  Demux81/1 -> Mux81/1
  Demux81/2 -> Mux81/2
  Mux81/1 -> mtx81/2
  Constant81/1 -> mtx81/1
  mtx81/1 -> [V_fn_84], Scope194/1
  [V_ll_85] -> Demux82/1
  Demux82/1 -> Mux82/1
  Demux82/2 -> Mux82/2
  Mux82/1 -> mtx82/2
  Constant82/1 -> mtx82/1
  mtx82/1 -> [V_fn_85], Scope195/1
  [V_ll_86] -> Demux83/1
  Demux83/1 -> Mux83/1
  Demux83/2 -> Mux83/2
  Mux83/1 -> mtx83/2
  Constant83/1 -> mtx83/1
  mtx83/1 -> [V_fn_86], Scope196/1
  [V_ll_88] -> Demux84/1
  Demux84/1 -> Mux84/1
  Demux84/2 -> Mux84/2
  Mux84/1 -> mtx84/2
  Constant84/1 -> mtx84/1
  mtx84/1 -> [V_fn_88], Scope197/1
  [V_ll_89] -> Demux85/1
  Demux85/1 -> Mux85/1
  Demux85/2 -> Mux85/2
  Mux85/1 -> mtx85/2
  Constant85/1 -> mtx85/1
  mtx85/1 -> [V_fn_89], Scope198/1
  [V_ll_90] -> Demux86/1
  Demux86/1 -> Mux86/1
  Demux86/2 -> Mux86/2
  Mux86/1 -> mtx86/2
  Constant86/1 -> mtx86/1
  mtx86/1 -> [V_fn_90], Scope199/1
  [V_ll_91] -> Demux87/1
  Demux87/1 -> Mux87/1
  Demux87/2 -> Mux87/2
  Mux87/1 -> mtx87/2
  Constant87/1 -> mtx87/1
  mtx87/1 -> [V_fn_91], Scope200/1
  [V_ll_92] -> Demux88/1
  Demux88/1 -> Mux88/1
  Demux88/2 -> Mux88/2
  Mux88/1 -> mtx88/2
  Constant88/1 -> mtx88/1
  mtx88/1 -> [V_fn_92], Scope201/1
  [V_ll_93] -> Demux89/1
  Demux89/1 -> Mux89/1
  Demux89/2 -> Mux89/2
  Mux89/1 -> mtx89/2
  Constant89/1 -> mtx89/1
  mtx89/1 -> [V_fn_93], Scope202/1
  [V_ll_94] -> Demux90/1
  Demux90/1 -> Mux90/1
  Demux90/2 -> Mux90/2
  Mux90/1 -> mtx90/2
  Constant90/1 -> mtx90/1
  mtx90/1 -> [V_fn_94], Scope203/1
  [V_ll_95] -> Demux91/1
  Demux91/1 -> Mux91/1
  Demux91/2 -> Mux91/2
  Mux91/1 -> mtx91/2
  Constant91/1 -> mtx91/1
  mtx91/1 -> [V_fn_95], Scope204/1
  [V_ll_96] -> Demux92/1
  Demux92/1 -> Mux92/1
  Demux92/2 -> Mux92/2
  Mux92/1 -> mtx92/2
  Constant92/1 -> mtx92/1
  mtx92/1 -> [V_fn_96], Scope205/1
  [V_ll_97] -> Demux93/1
  Demux93/1 -> Mux93/1
  Demux93/2 -> Mux93/2
  Mux93/1 -> mtx93/2
  Constant93/1 -> mtx93/1
  mtx93/1 -> [V_fn_97], Scope206/1
  [V_ll_98] -> Demux94/1
  Demux94/1 -> Mux94/1
  Demux94/2 -> Mux94/2
  Mux94/1 -> mtx94/2
  Constant94/1 -> mtx94/1
  mtx94/1 -> [V_fn_98], Scope207/1
  [V_ll_99] -> Demux95/1
  Demux95/1 -> Mux95/1
  Demux95/2 -> Mux95/2
  Mux95/1 -> mtx95/2
  Constant95/1 -> mtx95/1
  mtx95/1 -> [V_fn_99], Scope208/1
  [V_ll_100] -> Demux96/1
  Demux96/1 -> Mux96/1
  Demux96/2 -> Mux96/2
  Mux96/1 -> mtx96/2
  Constant96/1 -> mtx96/1
  mtx96/1 -> [V_fn_100], Scope209/1
  [V_ll_101] -> Demux97/1
  Demux97/1 -> Mux97/1
  Demux97/2 -> Mux97/2
  Mux97/1 -> mtx97/2
  Constant97/1 -> mtx97/1
  mtx97/1 -> [V_fn_101], Scope210/1
  [V_ll_102] -> Demux98/1
  Demux98/1 -> Mux98/1
  Demux98/2 -> Mux98/2
  Mux98/1 -> mtx98/2
  Constant98/1 -> mtx98/1
  mtx98/1 -> [V_fn_102], Scope211/1
  [V_ll_103] -> Demux99/1
  Demux99/1 -> Mux99/1
  Demux99/2 -> Mux99/2
  Mux99/1 -> mtx99/2
  Constant99/1 -> mtx99/1
  mtx99/1 -> [V_fn_103], Scope212/1
  [V_ll_104] -> Demux100/1
  Demux100/1 -> Mux100/1
  Demux100/2 -> Mux100/2
  Mux100/1 -> mtx100/2
  Constant100/1 -> mtx100/1
  mtx100/1 -> [V_fn_104], Scope213/1
  [V_ll_105] -> Demux101/1
  Demux101/1 -> Mux101/1
  Demux101/2 -> Mux101/2
  Mux101/1 -> mtx101/2
  Constant101/1 -> mtx101/1
  mtx101/1 -> [V_fn_105], Scope214/1
  [V_ll_106] -> Demux102/1
  Demux102/1 -> Mux102/1
  Demux102/2 -> Mux102/2
  Mux102/1 -> mtx102/2
  Constant102/1 -> mtx102/1
  mtx102/1 -> [V_fn_106], Scope215/1
  [V_ll_107] -> Demux103/1
  Demux103/1 -> Mux103/1
  Demux103/2 -> Mux103/2
  Mux103/1 -> mtx103/2
  Constant103/1 -> mtx103/1
  mtx103/1 -> [V_fn_107], Scope216/1
  [V_ll_108] -> Demux104/1
  Demux104/1 -> Mux104/1
  Demux104/2 -> Mux104/2
  Mux104/1 -> mtx104/2
  Constant104/1 -> mtx104/1
  mtx104/1 -> [V_fn_108], Scope217/1
  [V_ll_109] -> Demux105/1
  Demux105/1 -> Mux105/1
  Demux105/2 -> Mux105/2
  Mux105/1 -> mtx105/2
  Constant105/1 -> mtx105/1
  mtx105/1 -> [V_fn_109], Scope218/1
  [V_ll_110] -> Demux106/1
  Demux106/1 -> Mux106/1
  Demux106/2 -> Mux106/2
  Mux106/1 -> mtx106/2
  Constant106/1 -> mtx106/1
  mtx106/1 -> [V_fn_110], Scope219/1
  [V_ll_112] -> Demux107/1
  Demux107/1 -> Mux107/1
  Demux107/2 -> Mux107/2
  Mux107/1 -> mtx107/2
  Constant107/1 -> mtx107/1
  mtx107/1 -> [V_fn_112], Scope220/1
  [V_ll_113] -> Demux108/1
  Demux108/1 -> Mux108/1
  Demux108/2 -> Mux108/2
  Mux108/1 -> mtx108/2
  Constant108/1 -> mtx108/1
  mtx108/1 -> [V_fn_113], Scope221/1
  [V_ll_114] -> Demux109/1
  Demux109/1 -> Mux109/1
  Demux109/2 -> Mux109/2
  Mux109/1 -> mtx109/2
  Constant109/1 -> mtx109/1
  mtx109/1 -> [V_fn_114], Scope222/1
  [V_ll_115] -> Demux110/1
  Demux110/1 -> Mux110/1
  Demux110/2 -> Mux110/2
  Mux110/1 -> mtx110/2
  Constant110/1 -> mtx110/1
  mtx110/1 -> [V_fn_115], Scope223/1
  [V_ll_117] -> Demux111/1
  Demux111/1 -> Mux111/1
  Demux111/2 -> Mux111/2
  Mux111/1 -> mtx111/2
  Constant111/1 -> mtx111/1
  mtx111/1 -> [V_fn_117], Scope224/1
  [V_ll_118] -> Demux112/1
  Demux112/1 -> Mux112/1
  Demux112/2 -> Mux112/2
  Mux112/1 -> mtx112/2
  Constant112/1 -> mtx112/1
  mtx112/1 -> [V_fn_118], Scope225/1
  [V_fn_1] -> Power/1
  [I_Load1] -> Power/2
  Power/1 -> To Workspace_P_Load1/1, Scope226/1, Scope228/1
  Power/2 -> To Workspace_Q_Load1/1, Scope227/1, Scope228/2
  [V_fn_12] -> Power1/1
  [I_SG1] -> Power1/2
  Power1/1 -> To Workspace_P_SG1/1, Scope229/1, Scope231/1
  Power1/2 -> To Workspace_Q_SG1/1, Scope230/1, Scope231/2
  [V_fn_19] -> Power2/1
  [I_VSC1] -> Power2/2
  Power2/1 -> To Workspace_P_VSC1/1, Scope232/1, Scope234/1
  Power2/2 -> To Workspace_Q_VSC1/1, Scope233/1, Scope234/2
  [V_fn_2] -> Power3/1
  [I_Load2] -> Power3/2
  Power3/1 -> To Workspace_P_Load2/1, Scope235/1, Scope237/1
  Power3/2 -> To Workspace_Q_Load2/1, Scope236/1, Scope237/2
  [V_fn_19] -> Power4/1
  [I_SG2] -> Power4/2
  Power4/1 -> To Workspace_P_SG2/1, Scope238/1, Scope240/1
  Power4/2 -> To Workspace_Q_SG2/1, Scope239/1, Scope240/2
  [V_fn_31] -> Power5/1
  [I_VSC2] -> Power5/2
  Power5/1 -> To Workspace_P_VSC2/1, Scope241/1, Scope243/1
  Power5/2 -> To Workspace_Q_VSC2/1, Scope242/1, Scope243/2
  [V_fn_3] -> Power6/1
  [I_Load3] -> Power6/2
  Power6/1 -> To Workspace_P_Load3/1, Scope244/1, Scope246/1
  Power6/2 -> To Workspace_Q_Load3/1, Scope245/1, Scope246/2
  [V_fn_32] -> Power7/1
  [I_SG3] -> Power7/2
  Power7/1 -> To Workspace_P_SG3/1, Scope247/1, Scope249/1
  Power7/2 -> To Workspace_Q_SG3/1, Scope248/1, Scope249/2
  [V_fn_32] -> Power8/1
  [I_VSC3] -> Power8/2
  Power8/1 -> To Workspace_P_VSC3/1, Scope250/1, Scope252/1
  Power8/2 -> To Workspace_Q_VSC3/1, Scope251/1, Scope252/2
  [V_fn_4] -> Power9/1
  [I_Load4] -> Power9/2
  Power9/1 -> To Workspace_P_Load4/1, Scope253/1, Scope255/1
  Power9/2 -> To Workspace_Q_Load4/1, Scope254/1, Scope255/2
  [V_fn_34] -> Power10/1
  [I_SG4] -> Power10/2
  Power10/1 -> To Workspace_P_SG4/1, Scope256/1, Scope258/1
  Power10/2 -> To Workspace_Q_SG4/1, Scope257/1, Scope258/2
  [V_fn_54] -> Power11/1
  [I_VSC4] -> Power11/2
  Power11/1 -> To Workspace_P_VSC4/1, Scope259/1, Scope261/1
  Power11/2 -> To Workspace_Q_VSC4/1, Scope260/1, Scope261/2
  [V_fn_6] -> Power12/1
  [I_Load5] -> Power12/2
  Power12/1 -> To Workspace_P_Load5/1, Scope262/1, Scope264/1
  Power12/2 -> To Workspace_Q_Load5/1, Scope263/1, Scope264/2
  [V_fn_36] -> Power13/1
  [I_SG5] -> Power13/2
  Power13/1 -> To Workspace_P_SG5/1, Scope265/1, Scope267/1
  Power13/2 -> To Workspace_Q_SG5/1, Scope266/1, Scope267/2
  [V_fn_76] -> Power14/1
  [I_VSC5] -> Power14/2
  Power14/1 -> To Workspace_P_VSC5/1, Scope268/1, Scope270/1
  Power14/2 -> To Workspace_Q_VSC5/1, Scope269/1, Scope270/2
  [V_fn_7] -> Power15/1
  [I_Load6] -> Power15/2
  Power15/1 -> To Workspace_P_Load6/1, Scope271/1, Scope273/1
  Power15/2 -> To Workspace_Q_Load6/1, Scope272/1, Scope273/2
  [V_fn_40] -> Power16/1
  [I_SG6] -> Power16/2
  Power16/1 -> To Workspace_P_SG6/1, Scope274/1, Scope276/1
  Power16/2 -> To Workspace_Q_SG6/1, Scope275/1, Scope276/2
  [V_fn_92] -> Power17/1
  [I_VSC6] -> Power17/2
  Power17/1 -> To Workspace_P_VSC6/1, Scope277/1, Scope279/1
  Power17/2 -> To Workspace_Q_VSC6/1, Scope278/1, Scope279/2
  [V_fn_11] -> Power18/1
  [I_Load7] -> Power18/2
  Power18/1 -> To Workspace_P_Load7/1, Scope280/1, Scope282/1
  Power18/2 -> To Workspace_Q_Load7/1, Scope281/1, Scope282/2
  [V_fn_46] -> Power19/1
  [I_SG7] -> Power19/2
  Power19/1 -> To Workspace_P_SG7/1, Scope283/1, Scope285/1
  Power19/2 -> To Workspace_Q_SG7/1, Scope284/1, Scope285/2
  [V_fn_100] -> Power20/1
  [I_VSC7] -> Power20/2
  Power20/1 -> To Workspace_P_VSC7/1, Scope286/1, Scope288/1
  Power20/2 -> To Workspace_Q_VSC7/1, Scope287/1, Scope288/2
  [V_fn_12] -> Power21/1
  [I_Load8] -> Power21/2
  Power21/1 -> To Workspace_P_Load8/1, Scope289/1, Scope291/1
  Power21/2 -> To Workspace_Q_Load8/1, Scope290/1, Scope291/2
  [V_fn_49] -> Power22/1
  [I_SG8] -> Power22/2
  Power22/1 -> To Workspace_P_SG8/1, Scope292/1, Scope294/1
  Power22/2 -> To Workspace_Q_SG8/1, Scope293/1, Scope294/2
  [V_fn_105] -> Power23/1
  [I_VSC8] -> Power23/2
  Power23/1 -> To Workspace_P_VSC8/1, Scope295/1, Scope297/1
  Power23/2 -> To Workspace_Q_VSC8/1, Scope296/1, Scope297/2
  [V_fn_13] -> Power24/1
  [I_Load9] -> Power24/2
  Power24/1 -> To Workspace_P_Load9/1, Scope298/1, Scope300/1
  Power24/2 -> To Workspace_Q_Load9/1, Scope299/1, Scope300/2
  [V_fn_54] -> Power25/1
  [I_SG9] -> Power25/2
  Power25/1 -> To Workspace_P_SG9/1, Scope301/1, Scope303/1
  Power25/2 -> To Workspace_Q_SG9/1, Scope302/1, Scope303/2
  [V_fn_110] -> Power26/1
  [I_VSC9] -> Power26/2
  Power26/1 -> To Workspace_P_VSC9/1, Scope304/1, Scope306/1
  Power26/2 -> To Workspace_Q_VSC9/1, Scope305/1, Scope306/2
  [V_fn_14] -> Power27/1
  [I_Load10] -> Power27/2
  Power27/1 -> To Workspace_P_Load10/1, Scope307/1, Scope309/1
  Power27/2 -> To Workspace_Q_Load10/1, Scope308/1, Scope309/2
  [V_fn_59] -> Power28/1
  [I_SG10] -> Power28/2
  Power28/1 -> To Workspace_P_SG10/1, Scope310/1, Scope312/1
  Power28/2 -> To Workspace_Q_SG10/1, Scope311/1, Scope312/2
  [V_fn_112] -> Power29/1
  [I_VSC10] -> Power29/2
  Power29/1 -> To Workspace_P_VSC10/1, Scope313/1, Scope315/1
  Power29/2 -> To Workspace_Q_VSC10/1, Scope314/1, Scope315/2
  [V_fn_15] -> Power30/1
  [I_Load11] -> Power30/2
  Power30/1 -> To Workspace_P_Load11/1, Scope316/1, Scope318/1
  Power30/2 -> To Workspace_Q_Load11/1, Scope317/1, Scope318/2
  [V_fn_19] -> Power31/1
  [I_VSC11] -> Power31/2
  Power31/1 -> To Workspace_P_VSC11/1, Scope319/1, Scope321/1
  Power31/2 -> To Workspace_Q_VSC11/1, Scope320/1, Scope321/2
  [V_fn_65] -> Power32/1
  [I_SG11] -> Power32/2
  Power32/1 -> To Workspace_P_SG11/1, Scope322/1, Scope324/1
  Power32/2 -> To Workspace_Q_SG11/1, Scope323/1, Scope324/2
  [V_fn_16] -> Power33/1
  [I_Load12] -> Power33/2
  Power33/1 -> To Workspace_P_Load12/1, Scope325/1, Scope327/1
  Power33/2 -> To Workspace_Q_Load12/1, Scope326/1, Scope327/2
  [V_fn_31] -> Power34/1
  [I_VSC12] -> Power34/2
  Power34/1 -> To Workspace_P_VSC12/1, Scope328/1, Scope330/1
  Power34/2 -> To Workspace_Q_VSC12/1, Scope329/1, Scope330/2
  [V_fn_70] -> Power35/1
  [I_SG12] -> Power35/2
  Power35/1 -> To Workspace_P_SG12/1, Scope331/1, Scope333/1
  Power35/2 -> To Workspace_Q_SG12/1, Scope332/1, Scope333/2
  [V_fn_17] -> Power36/1
  [I_Load13] -> Power36/2
  Power36/1 -> To Workspace_P_Load13/1, Scope334/1, Scope336/1
  Power36/2 -> To Workspace_Q_Load13/1, Scope335/1, Scope336/2
  [V_fn_32] -> Power37/1
  [I_VSC13] -> Power37/2
  Power37/1 -> To Workspace_P_VSC13/1, Scope337/1, Scope339/1
  Power37/2 -> To Workspace_Q_VSC13/1, Scope338/1, Scope339/2
  [V_fn_72] -> Power38/1
  [I_SG13] -> Power38/2
  Power38/1 -> To Workspace_P_SG13/1, Scope340/1, Scope342/1
  Power38/2 -> To Workspace_Q_SG13/1, Scope341/1, Scope342/2
  [V_fn_18] -> Power39/1
  [I_Load14] -> Power39/2
  Power39/1 -> To Workspace_P_Load14/1, Scope343/1, Scope345/1
  Power39/2 -> To Workspace_Q_Load14/1, Scope344/1, Scope345/2
  [V_fn_54] -> Power40/1
  [I_VSC14] -> Power40/2
  Power40/1 -> To Workspace_P_VSC14/1, Scope346/1, Scope348/1
  Power40/2 -> To Workspace_Q_VSC14/1, Scope347/1, Scope348/2
  [V_fn_73] -> Power41/1
  [I_SG14] -> Power41/2
  Power41/1 -> To Workspace_P_SG14/1, Scope349/1, Scope351/1
  Power41/2 -> To Workspace_Q_SG14/1, Scope350/1, Scope351/2
  [V_fn_19] -> Power42/1
  [I_Load15] -> Power42/2
  Power42/1 -> To Workspace_P_Load15/1, Scope352/1, Scope354/1
  Power42/2 -> To Workspace_Q_Load15/1, Scope353/1, Scope354/2
  [V_fn_76] -> Power43/1
  [I_SG15] -> Power43/2
  Power43/1 -> To Workspace_P_SG15/1, Scope355/1, Scope357/1
  Power43/2 -> To Workspace_Q_SG15/1, Scope356/1, Scope357/2
  [V_fn_76] -> Power44/1
  [I_VSC15] -> Power44/2
  Power44/1 -> To Workspace_P_VSC15/1, Scope358/1, Scope360/1
  Power44/2 -> To Workspace_Q_VSC15/1, Scope359/1, Scope360/2
  [V_fn_20] -> Power45/1
  [I_Load16] -> Power45/2
  Power45/1 -> To Workspace_P_Load16/1, Scope361/1, Scope363/1
  Power45/2 -> To Workspace_Q_Load16/1, Scope362/1, Scope363/2
  [V_fn_77] -> Power46/1
  [I_SG16] -> Power46/2
  Power46/1 -> To Workspace_P_SG16/1, Scope364/1, Scope366/1
  Power46/2 -> To Workspace_Q_SG16/1, Scope365/1, Scope366/2
  [V_fn_92] -> Power47/1
  [I_VSC16] -> Power47/2
  Power47/1 -> To Workspace_P_VSC16/1, Scope367/1, Scope369/1
  Power47/2 -> To Workspace_Q_VSC16/1, Scope368/1, Scope369/2
  [V_fn_21] -> Power48/1
  [I_Load17] -> Power48/2
  Power48/1 -> To Workspace_P_Load17/1, Scope370/1, Scope372/1
  Power48/2 -> To Workspace_Q_Load17/1, Scope371/1, Scope372/2
  [V_fn_80] -> Power49/1
  [I_SG17] -> Power49/2
  Power49/1 -> To Workspace_P_SG17/1, Scope373/1, Scope375/1
  Power49/2 -> To Workspace_Q_SG17/1, Scope374/1, Scope375/2
  [V_fn_100] -> Power50/1
  [I_VSC17] -> Power50/2
  Power50/1 -> To Workspace_P_VSC17/1, Scope376/1, Scope378/1
  Power50/2 -> To Workspace_Q_VSC17/1, Scope377/1, Scope378/2
  [V_fn_22] -> Power51/1
  [I_Load18] -> Power51/2
  Power51/1 -> To Workspace_P_Load18/1, Scope379/1, Scope381/1
  Power51/2 -> To Workspace_Q_Load18/1, Scope380/1, Scope381/2
  [V_fn_85] -> Power52/1
  [I_SG18] -> Power52/2
  Power52/1 -> To Workspace_P_SG18/1, Scope382/1, Scope384/1
  Power52/2 -> To Workspace_Q_SG18/1, Scope383/1, Scope384/2
  [V_fn_105] -> Power53/1
  [I_VSC18] -> Power53/2
  Power53/1 -> To Workspace_P_VSC18/1, Scope385/1, Scope387/1
  Power53/2 -> To Workspace_Q_VSC18/1, Scope386/1, Scope387/2
  [V_fn_23] -> Power54/1
  [I_Load19] -> Power54/2
  Power54/1 -> To Workspace_P_Load19/1, Scope388/1, Scope390/1
  Power54/2 -> To Workspace_Q_Load19/1, Scope389/1, Scope390/2
  [V_fn_89] -> Power55/1
  [I_SG19] -> Power55/2
  Power55/1 -> To Workspace_P_SG19/1, Scope391/1, Scope393/1
  Power55/2 -> To Workspace_Q_SG19/1, Scope392/1, Scope393/2
  [V_fn_110] -> Power56/1
  [I_VSC19] -> Power56/2
  Power56/1 -> To Workspace_P_VSC19/1, Scope394/1, Scope396/1
  Power56/2 -> To Workspace_Q_VSC19/1, Scope395/1, Scope396/2
  [V_fn_27] -> Power57/1
  [I_Load20] -> Power57/2
  Power57/1 -> To Workspace_P_Load20/1, Scope397/1, Scope399/1
  Power57/2 -> To Workspace_Q_Load20/1, Scope398/1, Scope399/2
  [V_fn_90] -> Power58/1
  [I_SG20] -> Power58/2
  Power58/1 -> To Workspace_P_SG20/1, Scope400/1, Scope402/1
  Power58/2 -> To Workspace_Q_SG20/1, Scope401/1, Scope402/2
  [V_fn_112] -> Power59/1
  [I_VSC20] -> Power59/2
  Power59/1 -> To Workspace_P_VSC20/1, Scope403/1, Scope405/1
  Power59/2 -> To Workspace_Q_VSC20/1, Scope404/1, Scope405/2
  [V_fn_28] -> Power60/1
  [I_Load21] -> Power60/2
  Power60/1 -> To Workspace_P_Load21/1, Scope406/1, Scope408/1
  Power60/2 -> To Workspace_Q_Load21/1, Scope407/1, Scope408/2
  [V_fn_92] -> Power61/1
  [I_SG21] -> Power61/2
  Power61/1 -> To Workspace_P_SG21/1, Scope409/1, Scope411/1
  Power61/2 -> To Workspace_Q_SG21/1, Scope410/1, Scope411/2
  [V_fn_29] -> Power62/1
  [I_Load22] -> Power62/2
  Power62/1 -> To Workspace_P_Load22/1, Scope412/1, Scope414/1
  Power62/2 -> To Workspace_Q_Load22/1, Scope413/1, Scope414/2
  [V_fn_100] -> Power63/1
  [I_SG22] -> Power63/2
  Power63/1 -> To Workspace_P_SG22/1, Scope415/1, Scope417/1
  Power63/2 -> To Workspace_Q_SG22/1, Scope416/1, Scope417/2
  [V_fn_31] -> Power64/1
  [I_Load23] -> Power64/2
  Power64/1 -> To Workspace_P_Load23/1, Scope418/1, Scope420/1
  Power64/2 -> To Workspace_Q_Load23/1, Scope419/1, Scope420/2
  [V_fn_105] -> Power65/1
  [I_SG23] -> Power65/2
  Power65/1 -> To Workspace_P_SG23/1, Scope421/1, Scope423/1
  Power65/2 -> To Workspace_Q_SG23/1, Scope422/1, Scope423/2
  [V_fn_32] -> Power66/1
  [I_Load24] -> Power66/2
  Power66/1 -> To Workspace_P_Load24/1, Scope424/1, Scope426/1
  Power66/2 -> To Workspace_Q_Load24/1, Scope425/1, Scope426/2
  [V_fn_107] -> Power67/1
  [I_SG24] -> Power67/2
  Power67/1 -> To Workspace_P_SG24/1, Scope427/1, Scope429/1
  Power67/2 -> To Workspace_Q_SG24/1, Scope428/1, Scope429/2
  [V_fn_33] -> Power68/1
  [I_Load25] -> Power68/2
  Power68/1 -> To Workspace_P_Load25/1, Scope430/1, Scope432/1
  Power68/2 -> To Workspace_Q_Load25/1, Scope431/1, Scope432/2
  [V_fn_112] -> Power69/1
  [I_SG25] -> Power69/2
  Power69/1 -> To Workspace_P_SG25/1, Scope433/1, Scope435/1
  Power69/2 -> To Workspace_Q_SG25/1, Scope434/1, Scope435/2
  [V_fn_34] -> Power70/1
  [I_Load26] -> Power70/2
  Power70/1 -> To Workspace_P_Load26/1, Scope436/1, Scope438/1
  Power70/2 -> To Workspace_Q_Load26/1, Scope437/1, Scope438/2
  [V_fn_113] -> Power71/1
  [I_SG26] -> Power71/2
  Power71/1 -> To Workspace_P_SG26/1, Scope439/1, Scope441/1
  Power71/2 -> To Workspace_Q_SG26/1, Scope440/1, Scope441/2
  [V_fn_35] -> Power72/1
  [I_Load27] -> Power72/2
  Power72/1 -> To Workspace_P_Load27/1, Scope442/1, Scope444/1
  Power72/2 -> To Workspace_Q_Load27/1, Scope443/1, Scope444/2
  [V_fn_36] -> Power73/1
  [I_Load28] -> Power73/2
  Power73/1 -> To Workspace_P_Load28/1, Scope445/1, Scope447/1
  Power73/2 -> To Workspace_Q_Load28/1, Scope446/1, Scope447/2
  [V_fn_37] -> Power74/1
  [I_Load29] -> Power74/2
  Power74/1 -> To Workspace_P_Load29/1, Scope448/1, Scope450/1
  Power74/2 -> To Workspace_Q_Load29/1, Scope449/1, Scope450/2
  [V_fn_40] -> Power75/1
  [I_Load30] -> Power75/2
  Power75/1 -> To Workspace_P_Load30/1, Scope451/1, Scope453/1
  Power75/2 -> To Workspace_Q_Load30/1, Scope452/1, Scope453/2
  [V_fn_41] -> Power76/1
  [I_Load31] -> Power76/2
  Power76/1 -> To Workspace_P_Load31/1, Scope454/1, Scope456/1
  Power76/2 -> To Workspace_Q_Load31/1, Scope455/1, Scope456/2
  [V_fn_42] -> Power77/1
  [I_Load32] -> Power77/2
  Power77/1 -> To Workspace_P_Load32/1, Scope457/1, Scope459/1
  Power77/2 -> To Workspace_Q_Load32/1, Scope458/1, Scope459/2
  [V_fn_43] -> Power78/1
  [I_Load33] -> Power78/2
  Power78/1 -> To Workspace_P_Load33/1, Scope460/1, Scope462/1
  Power78/2 -> To Workspace_Q_Load33/1, Scope461/1, Scope462/2
  [V_fn_44] -> Power79/1
  [I_Load34] -> Power79/2
  Power79/1 -> To Workspace_P_Load34/1, Scope463/1, Scope465/1
  Power79/2 -> To Workspace_Q_Load34/1, Scope464/1, Scope465/2
  [V_fn_45] -> Power80/1
  [I_Load35] -> Power80/2
  Power80/1 -> To Workspace_P_Load35/1, Scope466/1, Scope468/1
  Power80/2 -> To Workspace_Q_Load35/1, Scope467/1, Scope468/2
  [V_fn_46] -> Power81/1
  [I_Load36] -> Power81/2
  Power81/1 -> To Workspace_P_Load36/1, Scope469/1, Scope471/1
  Power81/2 -> To Workspace_Q_Load36/1, Scope470/1, Scope471/2
  [V_fn_47] -> Power82/1
  [I_Load37] -> Power82/2
  Power82/1 -> To Workspace_P_Load37/1, Scope472/1, Scope474/1
  Power82/2 -> To Workspace_Q_Load37/1, Scope473/1, Scope474/2
  [V_fn_48] -> Power83/1
  [I_Load38] -> Power83/2
  Power83/1 -> To Workspace_P_Load38/1, Scope475/1, Scope477/1
  Power83/2 -> To Workspace_Q_Load38/1, Scope476/1, Scope477/2
  [V_fn_49] -> Power84/1
  [I_Load39] -> Power84/2
  Power84/1 -> To Workspace_P_Load39/1, Scope478/1, Scope480/1
  Power84/2 -> To Workspace_Q_Load39/1, Scope479/1, Scope480/2
  [V_fn_50] -> Power85/1
  [I_Load40] -> Power85/2
  Power85/1 -> To Workspace_P_Load40/1, Scope481/1, Scope483/1
  Power85/2 -> To Workspace_Q_Load40/1, Scope482/1, Scope483/2
  [V_fn_51] -> Power86/1
  [I_Load41] -> Power86/2
  Power86/1 -> To Workspace_P_Load41/1, Scope484/1, Scope486/1
  Power86/2 -> To Workspace_Q_Load41/1, Scope485/1, Scope486/2
  [V_fn_52] -> Power87/1
  [I_Load42] -> Power87/2
  Power87/1 -> To Workspace_P_Load42/1, Scope487/1, Scope489/1
  Power87/2 -> To Workspace_Q_Load42/1, Scope488/1, Scope489/2
  [V_fn_53] -> Power88/1
  [I_Load43] -> Power88/2
  Power88/1 -> To Workspace_P_Load43/1, Scope490/1, Scope492/1
  Power88/2 -> To Workspace_Q_Load43/1, Scope491/1, Scope492/2
  [V_fn_54] -> Power89/1
  [I_Load44] -> Power89/2
  Power89/1 -> To Workspace_P_Load44/1, Scope493/1, Scope495/1
  Power89/2 -> To Workspace_Q_Load44/1, Scope494/1, Scope495/2
  [V_fn_55] -> Power90/1
  [I_Load45] -> Power90/2
  Power90/1 -> To Workspace_P_Load45/1, Scope496/1, Scope498/1
  Power90/2 -> To Workspace_Q_Load45/1, Scope497/1, Scope498/2
  [V_fn_56] -> Power91/1
  [I_Load46] -> Power91/2
  Power91/1 -> To Workspace_P_Load46/1, Scope499/1, Scope501/1
  Power91/2 -> To Workspace_Q_Load46/1, Scope500/1, Scope501/2
  [V_fn_57] -> Power92/1
  [I_Load47] -> Power92/2
  Power92/1 -> To Workspace_P_Load47/1, Scope502/1, Scope504/1
  Power92/2 -> To Workspace_Q_Load47/1, Scope503/1, Scope504/2
  [V_fn_58] -> Power93/1
  [I_Load48] -> Power93/2
  Power93/1 -> To Workspace_P_Load48/1, Scope505/1, Scope507/1
  Power93/2 -> To Workspace_Q_Load48/1, Scope506/1, Scope507/2
  [V_fn_59] -> Power94/1
  [I_Load49] -> Power94/2
  Power94/1 -> To Workspace_P_Load49/1, Scope508/1, Scope510/1
  Power94/2 -> To Workspace_Q_Load49/1, Scope509/1, Scope510/2
  [V_fn_60] -> Power95/1
  [I_Load50] -> Power95/2
  Power95/1 -> To Workspace_P_Load50/1, Scope511/1, Scope513/1
  Power95/2 -> To Workspace_Q_Load50/1, Scope512/1, Scope513/2
  [V_fn_62] -> Power96/1
  [I_Load51] -> Power96/2
  Power96/1 -> To Workspace_P_Load51/1, Scope514/1, Scope516/1
  Power96/2 -> To Workspace_Q_Load51/1, Scope515/1, Scope516/2
  [V_fn_66] -> Power97/1
  [I_Load52] -> Power97/2
  Power97/1 -> To Workspace_P_Load52/1, Scope517/1, Scope519/1
  Power97/2 -> To Workspace_Q_Load52/1, Scope518/1, Scope519/2
  [V_fn_67] -> Power98/1
  [I_Load53] -> Power98/2
  Power98/1 -> To Workspace_P_Load53/1, Scope520/1, Scope522/1
  Power98/2 -> To Workspace_Q_Load53/1, Scope521/1, Scope522/2
  [V_fn_70] -> Power99/1
  [I_Load54] -> Power99/2
  Power99/1 -> To Workspace_P_Load54/1, Scope523/1, Scope525/1
  Power99/2 -> To Workspace_Q_Load54/1, Scope524/1, Scope525/2
  [V_fn_74] -> Power100/1
  [I_Load55] -> Power100/2
  Power100/1 -> To Workspace_P_Load55/1, Scope526/1, Scope528/1
  Power100/2 -> To Workspace_Q_Load55/1, Scope527/1, Scope528/2
  [V_fn_75] -> Power101/1
  [I_Load56] -> Power101/2
  Power101/1 -> To Workspace_P_Load56/1, Scope529/1, Scope531/1
  Power101/2 -> To Workspace_Q_Load56/1, Scope530/1, Scope531/2
  [V_fn_76] -> Power102/1
  [I_Load57] -> Power102/2
  Power102/1 -> To Workspace_P_Load57/1, Scope532/1, Scope534/1
  Power102/2 -> To Workspace_Q_Load57/1, Scope533/1, Scope534/2
  [V_fn_77] -> Power103/1
  [I_Load58] -> Power103/2
  Power103/1 -> To Workspace_P_Load58/1, Scope535/1, Scope537/1
  Power103/2 -> To Workspace_Q_Load58/1, Scope536/1, Scope537/2
  [V_fn_78] -> Power104/1
  [I_Load59] -> Power104/2
  Power104/1 -> To Workspace_P_Load59/1, Scope538/1, Scope540/1
  Power104/2 -> To Workspace_Q_Load59/1, Scope539/1, Scope540/2
  [V_fn_79] -> Power105/1
  [I_Load60] -> Power105/2
  Power105/1 -> To Workspace_P_Load60/1, Scope541/1, Scope543/1
  Power105/2 -> To Workspace_Q_Load60/1, Scope542/1, Scope543/2
  [V_fn_80] -> Power106/1
  [I_Load61] -> Power106/2
  Power106/1 -> To Workspace_P_Load61/1, Scope544/1, Scope546/1
  Power106/2 -> To Workspace_Q_Load61/1, Scope545/1, Scope546/2
  [V_fn_82] -> Power107/1
  [I_Load62] -> Power107/2
  Power107/1 -> To Workspace_P_Load62/1, Scope547/1, Scope549/1
  Power107/2 -> To Workspace_Q_Load62/1, Scope548/1, Scope549/2
  [V_fn_83] -> Power108/1
  [I_Load63] -> Power108/2
  Power108/1 -> To Workspace_P_Load63/1, Scope550/1, Scope552/1
  Power108/2 -> To Workspace_Q_Load63/1, Scope551/1, Scope552/2
  [V_fn_84] -> Power109/1
  [I_Load64] -> Power109/2
  Power109/1 -> To Workspace_P_Load64/1, Scope553/1, Scope555/1
  Power109/2 -> To Workspace_Q_Load64/1, Scope554/1, Scope555/2
  [V_fn_85] -> Power110/1
  [I_Load65] -> Power110/2
  Power110/1 -> To Workspace_P_Load65/1, Scope556/1, Scope558/1
  Power110/2 -> To Workspace_Q_Load65/1, Scope557/1, Scope558/2
  [V_fn_86] -> Power111/1
  [I_Load66] -> Power111/2
  Power111/1 -> To Workspace_P_Load66/1, Scope559/1, Scope561/1
  Power111/2 -> To Workspace_Q_Load66/1, Scope560/1, Scope561/2
  [V_fn_88] -> Power112/1
  [I_Load67] -> Power112/2
  Power112/1 -> To Workspace_P_Load67/1, Scope562/1, Scope564/1
  Power112/2 -> To Workspace_Q_Load67/1, Scope563/1, Scope564/2
  [V_fn_90] -> Power113/1
  [I_Load68] -> Power113/2
  Power113/1 -> To Workspace_P_Load68/1, Scope565/1, Scope567/1
  Power113/2 -> To Workspace_Q_Load68/1, Scope566/1, Scope567/2
  [V_fn_92] -> Power114/1
  [I_Load69] -> Power114/2
  Power114/1 -> To Workspace_P_Load69/1, Scope568/1, Scope570/1
  Power114/2 -> To Workspace_Q_Load69/1, Scope569/1, Scope570/2
  [V_fn_93] -> Power115/1
  [I_Load70] -> Power115/2
  Power115/1 -> To Workspace_P_Load70/1, Scope571/1, Scope573/1
  Power115/2 -> To Workspace_Q_Load70/1, Scope572/1, Scope573/2
  [V_fn_94] -> Power116/1
  [I_Load71] -> Power116/2
  Power116/1 -> To Workspace_P_Load71/1, Scope574/1, Scope576/1
  Power116/2 -> To Workspace_Q_Load71/1, Scope575/1, Scope576/2
  [V_fn_95] -> Power117/1
  [I_Load72] -> Power117/2
  Power117/1 -> To Workspace_P_Load72/1, Scope577/1, Scope579/1
  Power117/2 -> To Workspace_Q_Load72/1, Scope578/1, Scope579/2
  [V_fn_96] -> Power118/1
  [I_Load73] -> Power118/2
  Power118/1 -> To Workspace_P_Load73/1, Scope580/1, Scope582/1
  Power118/2 -> To Workspace_Q_Load73/1, Scope581/1, Scope582/2
  [V_fn_97] -> Power119/1
  [I_Load74] -> Power119/2
  Power119/1 -> To Workspace_P_Load74/1, Scope583/1, Scope585/1
  Power119/2 -> To Workspace_Q_Load74/1, Scope584/1, Scope585/2
  [V_fn_98] -> Power120/1
  [I_Load75] -> Power120/2
  Power120/1 -> To Workspace_P_Load75/1, Scope586/1, Scope588/1
  Power120/2 -> To Workspace_Q_Load75/1, Scope587/1, Scope588/2
  [V_fn_100] -> Power121/1
  [I_Load76] -> Power121/2
  Power121/1 -> To Workspace_P_Load76/1, Scope589/1, Scope591/1
  Power121/2 -> To Workspace_Q_Load76/1, Scope590/1, Scope591/2
  [V_fn_101] -> Power122/1
  [I_Load77] -> Power122/2
  Power122/1 -> To Workspace_P_Load77/1, Scope592/1, Scope594/1
  Power122/2 -> To Workspace_Q_Load77/1, Scope593/1, Scope594/2
  [V_fn_102] -> Power123/1
  [I_Load78] -> Power123/2
  Power123/1 -> To Workspace_P_Load78/1, Scope595/1, Scope597/1
  Power123/2 -> To Workspace_Q_Load78/1, Scope596/1, Scope597/2
  [V_fn_103] -> Power124/1
  [I_Load79] -> Power124/2
  Power124/1 -> To Workspace_P_Load79/1, Scope598/1, Scope600/1
  Power124/2 -> To Workspace_Q_Load79/1, Scope599/1, Scope600/2
  [V_fn_104] -> Power125/1
  [I_Load80] -> Power125/2
  Power125/1 -> To Workspace_P_Load80/1, Scope601/1, Scope603/1
  Power125/2 -> To Workspace_Q_Load80/1, Scope602/1, Scope603/2
  [V_fn_105] -> Power126/1
  [I_Load81] -> Power126/2
  Power126/1 -> To Workspace_P_Load81/1, Scope604/1, Scope606/1
  Power126/2 -> To Workspace_Q_Load81/1, Scope605/1, Scope606/2
  [V_fn_106] -> Power127/1
  [I_Load82] -> Power127/2
  Power127/1 -> To Workspace_P_Load82/1, Scope607/1, Scope609/1
  Power127/2 -> To Workspace_Q_Load82/1, Scope608/1, Scope609/2
  [V_fn_107] -> Power128/1
  [I_Load83] -> Power128/2
  Power128/1 -> To Workspace_P_Load83/1, Scope610/1, Scope612/1
  Power128/2 -> To Workspace_Q_Load83/1, Scope611/1, Scope612/2
  [V_fn_108] -> Power129/1
  [I_Load84] -> Power129/2
  Power129/1 -> To Workspace_P_Load84/1, Scope613/1, Scope615/1
  Power129/2 -> To Workspace_Q_Load84/1, Scope614/1, Scope615/2
  [V_fn_109] -> Power130/1
  [I_Load85] -> Power130/2
  Power130/1 -> To Workspace_P_Load85/1, Scope616/1, Scope618/1
  Power130/2 -> To Workspace_Q_Load85/1, Scope617/1, Scope618/2
  [V_fn_110] -> Power131/1
  [I_Load86] -> Power131/2
  Power131/1 -> To Workspace_P_Load86/1, Scope619/1, Scope621/1
  Power131/2 -> To Workspace_Q_Load86/1, Scope620/1, Scope621/2
  [V_fn_112] -> Power132/1
  [I_Load87] -> Power132/2
  Power132/1 -> To Workspace_P_Load87/1, Scope622/1, Scope624/1
  Power132/2 -> To Workspace_Q_Load87/1, Scope623/1, Scope624/2
  [V_fn_114] -> Power133/1
  [I_Load88] -> Power133/2
  Power133/1 -> To Workspace_P_Load88/1, Scope625/1, Scope627/1
  Power133/2 -> To Workspace_Q_Load88/1, Scope626/1, Scope627/2
  [V_fn_115] -> Power134/1
  [I_Load89] -> Power134/2
  Power134/1 -> To Workspace_P_Load89/1, Scope628/1, Scope630/1
  Power134/2 -> To Workspace_Q_Load89/1, Scope629/1, Scope630/2
  [V_fn_117] -> Power135/1
  [I_Load90] -> Power135/2
  Power135/1 -> To Workspace_P_Load90/1, Scope631/1, Scope633/1
  Power135/2 -> To Workspace_Q_Load90/1, Scope632/1, Scope633/2
  [V_fn_118] -> Power136/1
  [I_Load91] -> Power136/2
  Power136/1 -> To Workspace_P_Load91/1, Scope634/1, Scope636/1
  Power136/2 -> To Workspace_Q_Load91/1, Scope635/1, Scope636/2
  [V_fn_1] -> qd/1
  [angle_ref] -> qd/2
  qd/1 -> To Workspace_NET.vn1q/1
  qd/2 -> To Workspace_NET.vn1d/1
  [V_fn_2] -> qd1/1
  [angle_ref] -> qd1/2
  qd1/1 -> To Workspace_NET.vn2q/1
  qd1/2 -> To Workspace_NET.vn2d/1
  [V_fn_3] -> qd2/1
  [angle_ref] -> qd2/2
  qd2/1 -> To Workspace_NET.vn3q/1
  qd2/2 -> To Workspace_NET.vn3d/1
  [V_fn_4] -> qd3/1
  [angle_ref] -> qd3/2
  qd3/1 -> To Workspace_NET.vn4q/1
  qd3/2 -> To Workspace_NET.vn4d/1
  [V_fn_5] -> qd4/1
  [angle_ref] -> qd4/2
  qd4/1 -> To Workspace_NET.vn5q/1
  qd4/2 -> To Workspace_NET.vn5d/1
  [V_fn_6] -> qd5/1
  [angle_ref] -> qd5/2
  qd5/1 -> To Workspace_NET.vn6q/1
  qd5/2 -> To Workspace_NET.vn6d/1
  [V_fn_7] -> qd6/1
  [angle_ref] -> qd6/2
  qd6/1 -> To Workspace_NET.vn7q/1
  qd6/2 -> To Workspace_NET.vn7d/1
  [V_fn_8] -> qd7/1
  [angle_ref] -> qd7/2
  qd7/1 -> To Workspace_NET.vn8q/1
  qd7/2 -> To Workspace_NET.vn8d/1
  [V_fn_11] -> qd8/1
  [angle_ref] -> qd8/2
  qd8/1 -> To Workspace_NET.vn11q/1
  qd8/2 -> To Workspace_NET.vn11d/1
  [V_fn_12] -> qd9/1
  [angle_ref] -> qd9/2
  qd9/1 -> To Workspace_NET.vn12q/1
  qd9/2 -> To Workspace_NET.vn12d/1
  [V_fn_13] -> qd10/1
  [angle_ref] -> qd10/2
  qd10/1 -> To Workspace_NET.vn13q/1
  qd10/2 -> To Workspace_NET.vn13d/1
  [V_fn_14] -> qd11/1
  [angle_ref] -> qd11/2
  qd11/1 -> To Workspace_NET.vn14q/1
  qd11/2 -> To Workspace_NET.vn14d/1
  [V_fn_15] -> qd12/1
  [angle_ref] -> qd12/2
  qd12/1 -> To Workspace_NET.vn15q/1
  qd12/2 -> To Workspace_NET.vn15d/1
  [V_fn_16] -> qd13/1
  [angle_ref] -> qd13/2
  qd13/1 -> To Workspace_NET.vn16q/1
  qd13/2 -> To Workspace_NET.vn16d/1
  [V_fn_17] -> qd14/1
  [angle_ref] -> qd14/2
  qd14/1 -> To Workspace_NET.vn17q/1
  qd14/2 -> To Workspace_NET.vn17d/1
  [V_fn_18] -> qd15/1
  [angle_ref] -> qd15/2
  qd15/1 -> To Workspace_NET.vn18q/1
  qd15/2 -> To Workspace_NET.vn18d/1
  [V_fn_19] -> qd16/1
  [angle_ref] -> qd16/2
  qd16/1 -> To Workspace_NET.vn19q/1
  qd16/2 -> To Workspace_NET.vn19d/1
  [V_fn_20] -> qd17/1
  [angle_ref] -> qd17/2
  qd17/1 -> To Workspace_NET.vn20q/1
  qd17/2 -> To Workspace_NET.vn20d/1
  [V_fn_21] -> qd18/1
  [angle_ref] -> qd18/2
  qd18/1 -> To Workspace_NET.vn21q/1
  qd18/2 -> To Workspace_NET.vn21d/1
  [V_fn_22] -> qd19/1
  [angle_ref] -> qd19/2
  qd19/1 -> To Workspace_NET.vn22q/1
  qd19/2 -> To Workspace_NET.vn22d/1
  [V_fn_23] -> qd20/1
  [angle_ref] -> qd20/2
  qd20/1 -> To Workspace_NET.vn23q/1
  qd20/2 -> To Workspace_NET.vn23d/1
  [V_fn_24] -> qd21/1
  [angle_ref] -> qd21/2
  qd21/1 -> To Workspace_NET.vn24q/1
  qd21/2 -> To Workspace_NET.vn24d/1
  [V_fn_25] -> qd22/1
  [angle_ref] -> qd22/2
  qd22/1 -> To Workspace_NET.vn25q/1
  qd22/2 -> To Workspace_NET.vn25d/1
  [V_fn_26] -> qd23/1
  [angle_ref] -> qd23/2
  qd23/1 -> To Workspace_NET.vn26q/1
  qd23/2 -> To Workspace_NET.vn26d/1
  [V_fn_27] -> qd24/1
  [angle_ref] -> qd24/2
  qd24/1 -> To Workspace_NET.vn27q/1
  qd24/2 -> To Workspace_NET.vn27d/1
  [V_fn_28] -> qd25/1
  [angle_ref] -> qd25/2
  qd25/1 -> To Workspace_NET.vn28q/1
  qd25/2 -> To Workspace_NET.vn28d/1
  [V_fn_29] -> qd26/1
  [angle_ref] -> qd26/2
  qd26/1 -> To Workspace_NET.vn29q/1
  qd26/2 -> To Workspace_NET.vn29d/1
  [V_fn_30] -> qd27/1
  [angle_ref] -> qd27/2
  qd27/1 -> To Workspace_NET.vn30q/1
  qd27/2 -> To Workspace_NET.vn30d/1
  [V_fn_31] -> qd28/1
  [angle_ref] -> qd28/2
  qd28/1 -> To Workspace_NET.vn31q/1
  qd28/2 -> To Workspace_NET.vn31d/1
  [V_fn_32] -> qd29/1
  [angle_ref] -> qd29/2
  qd29/1 -> To Workspace_NET.vn32q/1
  qd29/2 -> To Workspace_NET.vn32d/1
  [V_fn_33] -> qd30/1
  [angle_ref] -> qd30/2
  qd30/1 -> To Workspace_NET.vn33q/1
  qd30/2 -> To Workspace_NET.vn33d/1
  [V_fn_34] -> qd31/1
  [angle_ref] -> qd31/2
  qd31/1 -> To Workspace_NET.vn34q/1
  qd31/2 -> To Workspace_NET.vn34d/1
  [V_fn_35] -> qd32/1
  [angle_ref] -> qd32/2
  qd32/1 -> To Workspace_NET.vn35q/1
  qd32/2 -> To Workspace_NET.vn35d/1
  [V_fn_36] -> qd33/1
  [angle_ref] -> qd33/2
  qd33/1 -> To Workspace_NET.vn36q/1
  qd33/2 -> To Workspace_NET.vn36d/1
  [V_fn_37] -> qd34/1
  [angle_ref] -> qd34/2
  qd34/1 -> To Workspace_NET.vn37q/1
  qd34/2 -> To Workspace_NET.vn37d/1
  [V_fn_38] -> qd35/1
  [angle_ref] -> qd35/2
  qd35/1 -> To Workspace_NET.vn38q/1
  qd35/2 -> To Workspace_NET.vn38d/1
  [V_fn_39] -> qd36/1
  [angle_ref] -> qd36/2
  qd36/1 -> To Workspace_NET.vn39q/1
  qd36/2 -> To Workspace_NET.vn39d/1
  [V_fn_40] -> qd37/1
  [angle_ref] -> qd37/2
  qd37/1 -> To Workspace_NET.vn40q/1
  qd37/2 -> To Workspace_NET.vn40d/1
  [V_fn_41] -> qd38/1
  [angle_ref] -> qd38/2
  qd38/1 -> To Workspace_NET.vn41q/1
  qd38/2 -> To Workspace_NET.vn41d/1
  [V_fn_42] -> qd39/1
  [angle_ref] -> qd39/2
  qd39/1 -> To Workspace_NET.vn42q/1
  qd39/2 -> To Workspace_NET.vn42d/1
  [V_fn_43] -> qd40/1
  [angle_ref] -> qd40/2
  qd40/1 -> To Workspace_NET.vn43q/1
  qd40/2 -> To Workspace_NET.vn43d/1
  [V_fn_44] -> qd41/1
  [angle_ref] -> qd41/2
  qd41/1 -> To Workspace_NET.vn44q/1
  qd41/2 -> To Workspace_NET.vn44d/1
  [V_fn_45] -> qd42/1
  [angle_ref] -> qd42/2
  qd42/1 -> To Workspace_NET.vn45q/1
  qd42/2 -> To Workspace_NET.vn45d/1
  [V_fn_46] -> qd43/1
  [angle_ref] -> qd43/2
  qd43/1 -> To Workspace_NET.vn46q/1
  qd43/2 -> To Workspace_NET.vn46d/1
  [V_fn_47] -> qd44/1
  [angle_ref] -> qd44/2
  qd44/1 -> To Workspace_NET.vn47q/1
  qd44/2 -> To Workspace_NET.vn47d/1
  [V_fn_48] -> qd45/1
  [angle_ref] -> qd45/2
  qd45/1 -> To Workspace_NET.vn48q/1
  qd45/2 -> To Workspace_NET.vn48d/1
  [V_fn_49] -> qd46/1
  [angle_ref] -> qd46/2
  qd46/1 -> To Workspace_NET.vn49q/1
  qd46/2 -> To Workspace_NET.vn49d/1
  [V_fn_50] -> qd47/1
  [angle_ref] -> qd47/2
  qd47/1 -> To Workspace_NET.vn50q/1
  qd47/2 -> To Workspace_NET.vn50d/1
  [V_fn_51] -> qd48/1
  [angle_ref] -> qd48/2
  qd48/1 -> To Workspace_NET.vn51q/1
  qd48/2 -> To Workspace_NET.vn51d/1
  [V_fn_52] -> qd49/1
  [angle_ref] -> qd49/2
  qd49/1 -> To Workspace_NET.vn52q/1
  qd49/2 -> To Workspace_NET.vn52d/1
  [V_fn_53] -> qd50/1
  [angle_ref] -> qd50/2
  qd50/1 -> To Workspace_NET.vn53q/1
  qd50/2 -> To Workspace_NET.vn53d/1
  [V_fn_54] -> qd51/1
  [angle_ref] -> qd51/2
  qd51/1 -> To Workspace_NET.vn54q/1
  qd51/2 -> To Workspace_NET.vn54d/1
  [V_fn_55] -> qd52/1
  [angle_ref] -> qd52/2
  qd52/1 -> To Workspace_NET.vn55q/1
  qd52/2 -> To Workspace_NET.vn55d/1
  [V_fn_56] -> qd53/1
  [angle_ref] -> qd53/2
  qd53/1 -> To Workspace_NET.vn56q/1
  qd53/2 -> To Workspace_NET.vn56d/1
  [V_fn_57] -> qd54/1
  [angle_ref] -> qd54/2
  qd54/1 -> To Workspace_NET.vn57q/1
  qd54/2 -> To Workspace_NET.vn57d/1
  [V_fn_58] -> qd55/1
  [angle_ref] -> qd55/2
  qd55/1 -> To Workspace_NET.vn58q/1
  qd55/2 -> To Workspace_NET.vn58d/1
  [V_fn_59] -> qd56/1
  [angle_ref] -> qd56/2
  qd56/1 -> To Workspace_NET.vn59q/1
  qd56/2 -> To Workspace_NET.vn59d/1
  [V_fn_60] -> qd57/1
  [angle_ref] -> qd57/2
  qd57/1 -> To Workspace_NET.vn60q/1
  qd57/2 -> To Workspace_NET.vn60d/1
  [V_fn_61] -> qd58/1
  [angle_ref] -> qd58/2
  qd58/1 -> To Workspace_NET.vn61q/1
  qd58/2 -> To Workspace_NET.vn61d/1
  [V_fn_62] -> qd59/1
  [angle_ref] -> qd59/2
  qd59/1 -> To Workspace_NET.vn62q/1
  qd59/2 -> To Workspace_NET.vn62d/1
  [V_fn_63] -> qd60/1
  [angle_ref] -> qd60/2
  qd60/1 -> To Workspace_NET.vn63q/1
  qd60/2 -> To Workspace_NET.vn63d/1
  [V_fn_64] -> qd61/1
  [angle_ref] -> qd61/2
  qd61/1 -> To Workspace_NET.vn64q/1
  qd61/2 -> To Workspace_NET.vn64d/1
  [V_fn_65] -> qd62/1
  [angle_ref] -> qd62/2
  qd62/1 -> To Workspace_NET.vn65q/1
  qd62/2 -> To Workspace_NET.vn65d/1
  [V_fn_66] -> qd63/1
  [angle_ref] -> qd63/2
  qd63/1 -> To Workspace_NET.vn66q/1
  qd63/2 -> To Workspace_NET.vn66d/1
  [V_fn_67] -> qd64/1
  [angle_ref] -> qd64/2
  qd64/1 -> To Workspace_NET.vn67q/1
  qd64/2 -> To Workspace_NET.vn67d/1
  [V_fn_68] -> qd65/1
  [angle_ref] -> qd65/2
  qd65/1 -> To Workspace_NET.vn68q/1
  qd65/2 -> To Workspace_NET.vn68d/1
  [V_fn_69] -> qd66/1
  [angle_ref] -> qd66/2
  qd66/1 -> To Workspace_NET.vn69q/1
  qd66/2 -> To Workspace_NET.vn69d/1
  [V_fn_70] -> qd67/1
  [angle_ref] -> qd67/2
  qd67/1 -> To Workspace_NET.vn70q/1
  qd67/2 -> To Workspace_NET.vn70d/1
  [V_fn_71] -> qd68/1
  [angle_ref] -> qd68/2
  qd68/1 -> To Workspace_NET.vn71q/1
  qd68/2 -> To Workspace_NET.vn71d/1
  [V_fn_72] -> qd69/1
  [angle_ref] -> qd69/2
  qd69/1 -> To Workspace_NET.vn72q/1
  qd69/2 -> To Workspace_NET.vn72d/1
  [V_fn_73] -> qd70/1
  [angle_ref] -> qd70/2
  qd70/1 -> To Workspace_NET.vn73q/1
  qd70/2 -> To Workspace_NET.vn73d/1
  [V_fn_74] -> qd71/1
  [angle_ref] -> qd71/2
  qd71/1 -> To Workspace_NET.vn74q/1
  qd71/2 -> To Workspace_NET.vn74d/1
  [V_fn_75] -> qd72/1
  [angle_ref] -> qd72/2
  qd72/1 -> To Workspace_NET.vn75q/1
  qd72/2 -> To Workspace_NET.vn75d/1
  [V_fn_76] -> qd73/1
  [angle_ref] -> qd73/2
  qd73/1 -> To Workspace_NET.vn76q/1
  qd73/2 -> To Workspace_NET.vn76d/1
  [V_fn_77] -> qd74/1
  [angle_ref] -> qd74/2
  qd74/1 -> To Workspace_NET.vn77q/1
  qd74/2 -> To Workspace_NET.vn77d/1
  [V_fn_78] -> qd75/1
  [angle_ref] -> qd75/2
  qd75/1 -> To Workspace_NET.vn78q/1
  qd75/2 -> To Workspace_NET.vn78d/1
  [V_fn_79] -> qd76/1
  [angle_ref] -> qd76/2
  qd76/1 -> To Workspace_NET.vn79q/1
  qd76/2 -> To Workspace_NET.vn79d/1
  [V_fn_80] -> qd77/1
  [angle_ref] -> qd77/2
  qd77/1 -> To Workspace_NET.vn80q/1
  qd77/2 -> To Workspace_NET.vn80d/1
  [V_fn_81] -> qd78/1
  [angle_ref] -> qd78/2
  qd78/1 -> To Workspace_NET.vn81q/1
  qd78/2 -> To Workspace_NET.vn81d/1
  [V_fn_82] -> qd79/1
  [angle_ref] -> qd79/2
  qd79/1 -> To Workspace_NET.vn82q/1
  qd79/2 -> To Workspace_NET.vn82d/1
  [V_fn_83] -> qd80/1
  [angle_ref] -> qd80/2
  qd80/1 -> To Workspace_NET.vn83q/1
  qd80/2 -> To Workspace_NET.vn83d/1
  [V_fn_84] -> qd81/1
  [angle_ref] -> qd81/2
  qd81/1 -> To Workspace_NET.vn84q/1
  qd81/2 -> To Workspace_NET.vn84d/1
  [V_fn_85] -> qd82/1
  [angle_ref] -> qd82/2
  qd82/1 -> To Workspace_NET.vn85q/1
  qd82/2 -> To Workspace_NET.vn85d/1
  [V_fn_86] -> qd83/1
  [angle_ref] -> qd83/2
  qd83/1 -> To Workspace_NET.vn86q/1
  qd83/2 -> To Workspace_NET.vn86d/1
  [V_fn_88] -> qd84/1
  [angle_ref] -> qd84/2
  qd84/1 -> To Workspace_NET.vn88q/1
  qd84/2 -> To Workspace_NET.vn88d/1
  [V_fn_89] -> qd85/1
  [angle_ref] -> qd85/2
  qd85/1 -> To Workspace_NET.vn89q/1
  qd85/2 -> To Workspace_NET.vn89d/1
  [V_fn_90] -> qd86/1
  [angle_ref] -> qd86/2
  qd86/1 -> To Workspace_NET.vn90q/1
  qd86/2 -> To Workspace_NET.vn90d/1
  [V_fn_91] -> qd87/1
  [angle_ref] -> qd87/2
  qd87/1 -> To Workspace_NET.vn91q/1
  qd87/2 -> To Workspace_NET.vn91d/1
  [V_fn_92] -> qd88/1
  [angle_ref] -> qd88/2
  qd88/1 -> To Workspace_NET.vn92q/1
  qd88/2 -> To Workspace_NET.vn92d/1
  [V_fn_93] -> qd89/1
  [angle_ref] -> qd89/2
  qd89/1 -> To Workspace_NET.vn93q/1
  qd89/2 -> To Workspace_NET.vn93d/1
  [V_fn_94] -> qd90/1
  [angle_ref] -> qd90/2
  qd90/1 -> To Workspace_NET.vn94q/1
  qd90/2 -> To Workspace_NET.vn94d/1
  [V_fn_95] -> qd91/1
  [angle_ref] -> qd91/2
  qd91/1 -> To Workspace_NET.vn95q/1
  qd91/2 -> To Workspace_NET.vn95d/1
  [V_fn_96] -> qd92/1
  [angle_ref] -> qd92/2
  qd92/1 -> To Workspace_NET.vn96q/1
  qd92/2 -> To Workspace_NET.vn96d/1
  [V_fn_97] -> qd93/1
  [angle_ref] -> qd93/2
  qd93/1 -> To Workspace_NET.vn97q/1
  qd93/2 -> To Workspace_NET.vn97d/1
  [V_fn_98] -> qd94/1
  [angle_ref] -> qd94/2
  qd94/1 -> To Workspace_NET.vn98q/1
  qd94/2 -> To Workspace_NET.vn98d/1
  [V_fn_99] -> qd95/1
  [angle_ref] -> qd95/2
  qd95/1 -> To Workspace_NET.vn99q/1
  qd95/2 -> To Workspace_NET.vn99d/1
  [V_fn_100] -> qd96/1
  [angle_ref] -> qd96/2
  qd96/1 -> To Workspace_NET.vn100q/1
  qd96/2 -> To Workspace_NET.vn100d/1
  [V_fn_101] -> qd97/1
  [angle_ref] -> qd97/2
  qd97/1 -> To Workspace_NET.vn101q/1
  qd97/2 -> To Workspace_NET.vn101d/1
  [V_fn_102] -> qd98/1
  [angle_ref] -> qd98/2
  qd98/1 -> To Workspace_NET.vn102q/1
  qd98/2 -> To Workspace_NET.vn102d/1
  [V_fn_103] -> qd99/1
  [angle_ref] -> qd99/2
  qd99/1 -> To Workspace_NET.vn103q/1
  qd99/2 -> To Workspace_NET.vn103d/1
  [V_fn_104] -> qd100/1
  [angle_ref] -> qd100/2
  qd100/1 -> To Workspace_NET.vn104q/1
  qd100/2 -> To Workspace_NET.vn104d/1
  [V_fn_105] -> qd101/1
  [angle_ref] -> qd101/2
  qd101/1 -> To Workspace_NET.vn105q/1
  qd101/2 -> To Workspace_NET.vn105d/1
  [V_fn_106] -> qd102/1
  [angle_ref] -> qd102/2
  qd102/1 -> To Workspace_NET.vn106q/1
  qd102/2 -> To Workspace_NET.vn106d/1
  [V_fn_107] -> qd103/1
  [angle_ref] -> qd103/2
  qd103/1 -> To Workspace_NET.vn107q/1
  qd103/2 -> To Workspace_NET.vn107d/1
  [V_fn_108] -> qd104/1
  [angle_ref] -> qd104/2
  qd104/1 -> To Workspace_NET.vn108q/1
  qd104/2 -> To Workspace_NET.vn108d/1
  [V_fn_109] -> qd105/1
  [angle_ref] -> qd105/2
  qd105/1 -> To Workspace_NET.vn109q/1
  qd105/2 -> To Workspace_NET.vn109d/1
  [V_fn_110] -> qd106/1
  [angle_ref] -> qd106/2
  qd106/1 -> To Workspace_NET.vn110q/1
  qd106/2 -> To Workspace_NET.vn110d/1
  [V_fn_112] -> qd107/1
  [angle_ref] -> qd107/2
  qd107/1 -> To Workspace_NET.vn112q/1
  qd107/2 -> To Workspace_NET.vn112d/1
  [V_fn_113] -> qd108/1
  [angle_ref] -> qd108/2
  qd108/1 -> To Workspace_NET.vn113q/1
  qd108/2 -> To Workspace_NET.vn113d/1
  [V_fn_114] -> qd109/1
  [angle_ref] -> qd109/2
  qd109/1 -> To Workspace_NET.vn114q/1
  qd109/2 -> To Workspace_NET.vn114d/1
  [V_fn_115] -> qd110/1
  [angle_ref] -> qd110/2
  qd110/1 -> To Workspace_NET.vn115q/1
  qd110/2 -> To Workspace_NET.vn115d/1
  [V_fn_117] -> qd111/1
  [angle_ref] -> qd111/2
  qd111/1 -> To Workspace_NET.vn117q/1
  qd111/2 -> To Workspace_NET.vn117d/1
  [V_fn_118] -> qd112/1
  [angle_ref] -> qd112/2
  qd112/1 -> To Workspace_NET.vn118q/1
  qd112/2 -> To Workspace_NET.vn118d/1
  [I_Load1] -> qd113/1
  [angle_ref] -> qd113/2
  qd113/1 -> To Workspace_I_Load1_q/1
  qd113/2 -> To Workspace_I_Load1_d/1
  [I_SG1] -> qd114/1
  [angle_ref] -> qd114/2
  qd114/1 -> To Workspace_I_SG1_q/1
  qd114/2 -> To Workspace_I_SG1_d/1
  [I_VSC1] -> qd115/1
  [angle_ref] -> qd115/2
  qd115/1 -> To Workspace_I_VSC1_q/1
  qd115/2 -> To Workspace_I_VSC1_d/1
  [I_Load2] -> qd116/1
  [angle_ref] -> qd116/2
  qd116/1 -> To Workspace_I_Load2_q/1
  qd116/2 -> To Workspace_I_Load2_d/1
  [I_SG2] -> qd117/1
  [angle_ref] -> qd117/2
  qd117/1 -> To Workspace_I_SG2_q/1
  qd117/2 -> To Workspace_I_SG2_d/1
  [I_VSC2] -> qd118/1
  [angle_ref] -> qd118/2
  qd118/1 -> To Workspace_I_VSC2_q/1
  qd118/2 -> To Workspace_I_VSC2_d/1
  [I_Load3] -> qd119/1
  [angle_ref] -> qd119/2
  qd119/1 -> To Workspace_I_Load3_q/1
  qd119/2 -> To Workspace_I_Load3_d/1
  [I_SG3] -> qd120/1
  [angle_ref] -> qd120/2
  qd120/1 -> To Workspace_I_SG3_q/1
  qd120/2 -> To Workspace_I_SG3_d/1
  [I_VSC3] -> qd121/1
  [angle_ref] -> qd121/2
  qd121/1 -> To Workspace_I_VSC3_q/1
  qd121/2 -> To Workspace_I_VSC3_d/1
  [I_Load4] -> qd122/1
  [angle_ref] -> qd122/2
  qd122/1 -> To Workspace_I_Load4_q/1
  qd122/2 -> To Workspace_I_Load4_d/1
  [I_SG4] -> qd123/1
  [angle_ref] -> qd123/2
  qd123/1 -> To Workspace_I_SG4_q/1
  qd123/2 -> To Workspace_I_SG4_d/1
  [I_VSC4] -> qd124/1
  [angle_ref] -> qd124/2
  qd124/1 -> To Workspace_I_VSC4_q/1
  qd124/2 -> To Workspace_I_VSC4_d/1
  [I_Load5] -> qd125/1
  [angle_ref] -> qd125/2
  qd125/1 -> To Workspace_I_Load5_q/1
  qd125/2 -> To Workspace_I_Load5_d/1
  [I_SG5] -> qd126/1
  [angle_ref] -> qd126/2
  qd126/1 -> To Workspace_I_SG5_q/1
  qd126/2 -> To Workspace_I_SG5_d/1
  [I_VSC5] -> qd127/1
  [angle_ref] -> qd127/2
  qd127/1 -> To Workspace_I_VSC5_q/1
  qd127/2 -> To Workspace_I_VSC5_d/1
  [I_Load6] -> qd128/1
  [angle_ref] -> qd128/2
  qd128/1 -> To Workspace_I_Load6_q/1
  qd128/2 -> To Workspace_I_Load6_d/1
  [I_SG6] -> qd129/1
  [angle_ref] -> qd129/2
  qd129/1 -> To Workspace_I_SG6_q/1
  qd129/2 -> To Workspace_I_SG6_d/1
  [I_VSC6] -> qd130/1
  [angle_ref] -> qd130/2
  qd130/1 -> To Workspace_I_VSC6_q/1
  qd130/2 -> To Workspace_I_VSC6_d/1
  [I_Load7] -> qd131/1
  [angle_ref] -> qd131/2
  qd131/1 -> To Workspace_I_Load7_q/1
  qd131/2 -> To Workspace_I_Load7_d/1
  [I_SG7] -> qd132/1
  [angle_ref] -> qd132/2
  qd132/1 -> To Workspace_I_SG7_q/1
  qd132/2 -> To Workspace_I_SG7_d/1
  [I_VSC7] -> qd133/1
  [angle_ref] -> qd133/2
  qd133/1 -> To Workspace_I_VSC7_q/1
  qd133/2 -> To Workspace_I_VSC7_d/1
  [I_Load8] -> qd134/1
  [angle_ref] -> qd134/2
  qd134/1 -> To Workspace_I_Load8_q/1
  qd134/2 -> To Workspace_I_Load8_d/1
  [I_SG8] -> qd135/1
  [angle_ref] -> qd135/2
  qd135/1 -> To Workspace_I_SG8_q/1
  qd135/2 -> To Workspace_I_SG8_d/1
  [I_VSC8] -> qd136/1
  [angle_ref] -> qd136/2
  qd136/1 -> To Workspace_I_VSC8_q/1
  qd136/2 -> To Workspace_I_VSC8_d/1
  [I_Load9] -> qd137/1
  [angle_ref] -> qd137/2
  qd137/1 -> To Workspace_I_Load9_q/1
  qd137/2 -> To Workspace_I_Load9_d/1
  [I_SG9] -> qd138/1
  [angle_ref] -> qd138/2
  qd138/1 -> To Workspace_I_SG9_q/1
  qd138/2 -> To Workspace_I_SG9_d/1
  [I_VSC9] -> qd139/1
  [angle_ref] -> qd139/2
  qd139/1 -> To Workspace_I_VSC9_q/1
  qd139/2 -> To Workspace_I_VSC9_d/1
  [I_Load10] -> qd140/1
  [angle_ref] -> qd140/2
  qd140/1 -> To Workspace_I_Load10_q/1
  qd140/2 -> To Workspace_I_Load10_d/1
  [I_SG10] -> qd141/1
  [angle_ref] -> qd141/2
  qd141/1 -> To Workspace_I_SG10_q/1
  qd141/2 -> To Workspace_I_SG10_d/1
  [I_VSC10] -> qd142/1
  [angle_ref] -> qd142/2
  qd142/1 -> To Workspace_I_VSC10_q/1
  qd142/2 -> To Workspace_I_VSC10_d/1
  [I_Load11] -> qd143/1
  [angle_ref] -> qd143/2
  qd143/1 -> To Workspace_I_Load11_q/1
  qd143/2 -> To Workspace_I_Load11_d/1
  [I_VSC11] -> qd144/1
  [angle_ref] -> qd144/2
  qd144/1 -> To Workspace_I_VSC11_q/1
  qd144/2 -> To Workspace_I_VSC11_d/1
  [I_SG11] -> qd145/1
  [angle_ref] -> qd145/2
  qd145/1 -> To Workspace_I_SG11_q/1
  qd145/2 -> To Workspace_I_SG11_d/1
  [I_Load12] -> qd146/1
  [angle_ref] -> qd146/2
  qd146/1 -> To Workspace_I_Load12_q/1
  qd146/2 -> To Workspace_I_Load12_d/1
  [I_VSC12] -> qd147/1
  [angle_ref] -> qd147/2
  qd147/1 -> To Workspace_I_VSC12_q/1
  qd147/2 -> To Workspace_I_VSC12_d/1
  [I_SG12] -> qd148/1
  [angle_ref] -> qd148/2
  qd148/1 -> To Workspace_I_SG12_q/1
  qd148/2 -> To Workspace_I_SG12_d/1
  [I_Load13] -> qd149/1
  [angle_ref] -> qd149/2
  qd149/1 -> To Workspace_I_Load13_q/1
  qd149/2 -> To Workspace_I_Load13_d/1
  [I_VSC13] -> qd150/1
  [angle_ref] -> qd150/2
  qd150/1 -> To Workspace_I_VSC13_q/1
  qd150/2 -> To Workspace_I_VSC13_d/1
  [I_SG13] -> qd151/1
  [angle_ref] -> qd151/2
  qd151/1 -> To Workspace_I_SG13_q/1
  qd151/2 -> To Workspace_I_SG13_d/1
  [I_Load14] -> qd152/1
  [angle_ref] -> qd152/2
  qd152/1 -> To Workspace_I_Load14_q/1
  qd152/2 -> To Workspace_I_Load14_d/1
  [I_VSC14] -> qd153/1
  [angle_ref] -> qd153/2
  qd153/1 -> To Workspace_I_VSC14_q/1
  qd153/2 -> To Workspace_I_VSC14_d/1
  [I_SG14] -> qd154/1
  [angle_ref] -> qd154/2
  qd154/1 -> To Workspace_I_SG14_q/1
  qd154/2 -> To Workspace_I_SG14_d/1
  [I_Load15] -> qd155/1
  [angle_ref] -> qd155/2
  qd155/1 -> To Workspace_I_Load15_q/1
  qd155/2 -> To Workspace_I_Load15_d/1
  [I_SG15] -> qd156/1
  [angle_ref] -> qd156/2
  qd156/1 -> To Workspace_I_SG15_q/1
  qd156/2 -> To Workspace_I_SG15_d/1
  [I_VSC15] -> qd157/1
  [angle_ref] -> qd157/2
  qd157/1 -> To Workspace_I_VSC15_q/1
  qd157/2 -> To Workspace_I_VSC15_d/1
  [I_Load16] -> qd158/1
  [angle_ref] -> qd158/2
  qd158/1 -> To Workspace_I_Load16_q/1
  qd158/2 -> To Workspace_I_Load16_d/1
  [I_SG16] -> qd159/1
  [angle_ref] -> qd159/2
  qd159/1 -> To Workspace_I_SG16_q/1
  qd159/2 -> To Workspace_I_SG16_d/1
  [I_VSC16] -> qd160/1
  [angle_ref] -> qd160/2
  qd160/1 -> To Workspace_I_VSC16_q/1
  qd160/2 -> To Workspace_I_VSC16_d/1
  [I_Load17] -> qd161/1
  [angle_ref] -> qd161/2
  qd161/1 -> To Workspace_I_Load17_q/1
  qd161/2 -> To Workspace_I_Load17_d/1
  [I_SG17] -> qd162/1
  [angle_ref] -> qd162/2
  qd162/1 -> To Workspace_I_SG17_q/1
  qd162/2 -> To Workspace_I_SG17_d/1
  [I_VSC17] -> qd163/1
  [angle_ref] -> qd163/2
  qd163/1 -> To Workspace_I_VSC17_q/1
  qd163/2 -> To Workspace_I_VSC17_d/1
  [I_Load18] -> qd164/1
  [angle_ref] -> qd164/2
  qd164/1 -> To Workspace_I_Load18_q/1
  qd164/2 -> To Workspace_I_Load18_d/1
  [I_SG18] -> qd165/1
  [angle_ref] -> qd165/2
  qd165/1 -> To Workspace_I_SG18_q/1
  qd165/2 -> To Workspace_I_SG18_d/1
  [I_VSC18] -> qd166/1
  [angle_ref] -> qd166/2
  qd166/1 -> To Workspace_I_VSC18_q/1
  qd166/2 -> To Workspace_I_VSC18_d/1
  [I_Load19] -> qd167/1
  [angle_ref] -> qd167/2
  qd167/1 -> To Workspace_I_Load19_q/1
  qd167/2 -> To Workspace_I_Load19_d/1
  [I_SG19] -> qd168/1
  [angle_ref] -> qd168/2
  qd168/1 -> To Workspace_I_SG19_q/1
  qd168/2 -> To Workspace_I_SG19_d/1
  [I_VSC19] -> qd169/1
  [angle_ref] -> qd169/2
  qd169/1 -> To Workspace_I_VSC19_q/1
  qd169/2 -> To Workspace_I_VSC19_d/1
  [I_Load20] -> qd170/1
  [angle_ref] -> qd170/2
  qd170/1 -> To Workspace_I_Load20_q/1
  qd170/2 -> To Workspace_I_Load20_d/1
  [I_SG20] -> qd171/1
  [angle_ref] -> qd171/2
  qd171/1 -> To Workspace_I_SG20_q/1
  qd171/2 -> To Workspace_I_SG20_d/1
  [I_VSC20] -> qd172/1
  [angle_ref] -> qd172/2
  qd172/1 -> To Workspace_I_VSC20_q/1
  qd172/2 -> To Workspace_I_VSC20_d/1
  [I_Load21] -> qd173/1
  [angle_ref] -> qd173/2
  qd173/1 -> To Workspace_I_Load21_q/1
  qd173/2 -> To Workspace_I_Load21_d/1
  [I_SG21] -> qd174/1
  [angle_ref] -> qd174/2
  qd174/1 -> To Workspace_I_SG21_q/1
  qd174/2 -> To Workspace_I_SG21_d/1
  [I_Load22] -> qd175/1
  [angle_ref] -> qd175/2
  qd175/1 -> To Workspace_I_Load22_q/1
  qd175/2 -> To Workspace_I_Load22_d/1
  [I_SG22] -> qd176/1
  [angle_ref] -> qd176/2
  qd176/1 -> To Workspace_I_SG22_q/1
  qd176/2 -> To Workspace_I_SG22_d/1
  [I_Load23] -> qd177/1
  [angle_ref] -> qd177/2
  qd177/1 -> To Workspace_I_Load23_q/1
  qd177/2 -> To Workspace_I_Load23_d/1
  [I_SG23] -> qd178/1
  [angle_ref] -> qd178/2
  qd178/1 -> To Workspace_I_SG23_q/1
  qd178/2 -> To Workspace_I_SG23_d/1
  [I_Load24] -> qd179/1
  [angle_ref] -> qd179/2
  qd179/1 -> To Workspace_I_Load24_q/1
  qd179/2 -> To Workspace_I_Load24_d/1
  [I_SG24] -> qd180/1
  [angle_ref] -> qd180/2
  qd180/1 -> To Workspace_I_SG24_q/1
  qd180/2 -> To Workspace_I_SG24_d/1
  [I_Load25] -> qd181/1
  [angle_ref] -> qd181/2
  qd181/1 -> To Workspace_I_Load25_q/1
  qd181/2 -> To Workspace_I_Load25_d/1
  [I_SG25] -> qd182/1
  [angle_ref] -> qd182/2
  qd182/1 -> To Workspace_I_SG25_q/1
  qd182/2 -> To Workspace_I_SG25_d/1
  [I_Load26] -> qd183/1
  [angle_ref] -> qd183/2
  qd183/1 -> To Workspace_I_Load26_q/1
  qd183/2 -> To Workspace_I_Load26_d/1
  [I_SG26] -> qd184/1
  [angle_ref] -> qd184/2
  qd184/1 -> To Workspace_I_SG26_q/1
  qd184/2 -> To Workspace_I_SG26_d/1
  [I_Load27] -> qd185/1
  [angle_ref] -> qd185/2
  qd185/1 -> To Workspace_I_Load27_q/1
  qd185/2 -> To Workspace_I_Load27_d/1
  [I_Load28] -> qd186/1
  [angle_ref] -> qd186/2
  qd186/1 -> To Workspace_I_Load28_q/1
  qd186/2 -> To Workspace_I_Load28_d/1
  [I_Load29] -> qd187/1
  [angle_ref] -> qd187/2
  qd187/1 -> To Workspace_I_Load29_q/1
  qd187/2 -> To Workspace_I_Load29_d/1
  [I_Load30] -> qd188/1
  [angle_ref] -> qd188/2
  qd188/1 -> To Workspace_I_Load30_q/1
  qd188/2 -> To Workspace_I_Load30_d/1
  [I_Load31] -> qd189/1
  [angle_ref] -> qd189/2
  qd189/1 -> To Workspace_I_Load31_q/1
  qd189/2 -> To Workspace_I_Load31_d/1
  [I_Load32] -> qd190/1
  [angle_ref] -> qd190/2
  qd190/1 -> To Workspace_I_Load32_q/1
  qd190/2 -> To Workspace_I_Load32_d/1
  [I_Load33] -> qd191/1
  [angle_ref] -> qd191/2
  qd191/1 -> To Workspace_I_Load33_q/1
  qd191/2 -> To Workspace_I_Load33_d/1
  [I_Load34] -> qd192/1
  [angle_ref] -> qd192/2
  qd192/1 -> To Workspace_I_Load34_q/1
  qd192/2 -> To Workspace_I_Load34_d/1
  [I_Load35] -> qd193/1
  [angle_ref] -> qd193/2
  qd193/1 -> To Workspace_I_Load35_q/1
  qd193/2 -> To Workspace_I_Load35_d/1
  [I_Load36] -> qd194/1
  [angle_ref] -> qd194/2
  qd194/1 -> To Workspace_I_Load36_q/1
  qd194/2 -> To Workspace_I_Load36_d/1
  [I_Load37] -> qd195/1
  [angle_ref] -> qd195/2
  qd195/1 -> To Workspace_I_Load37_q/1
  qd195/2 -> To Workspace_I_Load37_d/1
  [I_Load38] -> qd196/1
  [angle_ref] -> qd196/2
  qd196/1 -> To Workspace_I_Load38_q/1
  qd196/2 -> To Workspace_I_Load38_d/1
  [I_Load39] -> qd197/1
  [angle_ref] -> qd197/2
  qd197/1 -> To Workspace_I_Load39_q/1
  qd197/2 -> To Workspace_I_Load39_d/1
  [I_Load40] -> qd198/1
  [angle_ref] -> qd198/2
  qd198/1 -> To Workspace_I_Load40_q/1
  qd198/2 -> To Workspace_I_Load40_d/1
  [I_Load41] -> qd199/1
  [angle_ref] -> qd199/2
  qd199/1 -> To Workspace_I_Load41_q/1
  qd199/2 -> To Workspace_I_Load41_d/1
  [I_Load42] -> qd200/1
  [angle_ref] -> qd200/2
  qd200/1 -> To Workspace_I_Load42_q/1
  qd200/2 -> To Workspace_I_Load42_d/1
  [I_Load43] -> qd201/1
  [angle_ref] -> qd201/2
  qd201/1 -> To Workspace_I_Load43_q/1
  qd201/2 -> To Workspace_I_Load43_d/1
  [I_Load44] -> qd202/1
  [angle_ref] -> qd202/2
  qd202/1 -> To Workspace_I_Load44_q/1
  qd202/2 -> To Workspace_I_Load44_d/1
  [I_Load45] -> qd203/1
  [angle_ref] -> qd203/2
  qd203/1 -> To Workspace_I_Load45_q/1
  qd203/2 -> To Workspace_I_Load45_d/1
  [I_Load46] -> qd204/1
  [angle_ref] -> qd204/2
  qd204/1 -> To Workspace_I_Load46_q/1
  qd204/2 -> To Workspace_I_Load46_d/1
  [I_Load47] -> qd205/1
  [angle_ref] -> qd205/2
  qd205/1 -> To Workspace_I_Load47_q/1
  qd205/2 -> To Workspace_I_Load47_d/1
  [I_Load48] -> qd206/1
  [angle_ref] -> qd206/2
  qd206/1 -> To Workspace_I_Load48_q/1
  qd206/2 -> To Workspace_I_Load48_d/1
  [I_Load49] -> qd207/1
  [angle_ref] -> qd207/2
  qd207/1 -> To Workspace_I_Load49_q/1
  qd207/2 -> To Workspace_I_Load49_d/1
  [I_Load50] -> qd208/1
  [angle_ref] -> qd208/2
  qd208/1 -> To Workspace_I_Load50_q/1
  qd208/2 -> To Workspace_I_Load50_d/1
  [I_Load51] -> qd209/1
  [angle_ref] -> qd209/2
  qd209/1 -> To Workspace_I_Load51_q/1
  qd209/2 -> To Workspace_I_Load51_d/1
  [I_Load52] -> qd210/1
  [angle_ref] -> qd210/2
  qd210/1 -> To Workspace_I_Load52_q/1
  qd210/2 -> To Workspace_I_Load52_d/1
  [I_Load53] -> qd211/1
  [angle_ref] -> qd211/2
  qd211/1 -> To Workspace_I_Load53_q/1
  qd211/2 -> To Workspace_I_Load53_d/1
  [I_Load54] -> qd212/1
  [angle_ref] -> qd212/2
  qd212/1 -> To Workspace_I_Load54_q/1
  qd212/2 -> To Workspace_I_Load54_d/1
  [I_Load55] -> qd213/1
  [angle_ref] -> qd213/2
  qd213/1 -> To Workspace_I_Load55_q/1
  qd213/2 -> To Workspace_I_Load55_d/1
  [I_Load56] -> qd214/1
  [angle_ref] -> qd214/2
  qd214/1 -> To Workspace_I_Load56_q/1
  qd214/2 -> To Workspace_I_Load56_d/1
  [I_Load57] -> qd215/1
  [angle_ref] -> qd215/2
  qd215/1 -> To Workspace_I_Load57_q/1
  qd215/2 -> To Workspace_I_Load57_d/1
  [I_Load58] -> qd216/1
  [angle_ref] -> qd216/2
  qd216/1 -> To Workspace_I_Load58_q/1
  qd216/2 -> To Workspace_I_Load58_d/1
  [I_Load59] -> qd217/1
  [angle_ref] -> qd217/2
  qd217/1 -> To Workspace_I_Load59_q/1
  qd217/2 -> To Workspace_I_Load59_d/1
  [I_Load60] -> qd218/1
  [angle_ref] -> qd218/2
  qd218/1 -> To Workspace_I_Load60_q/1
  qd218/2 -> To Workspace_I_Load60_d/1
  [I_Load61] -> qd219/1
  [angle_ref] -> qd219/2
  qd219/1 -> To Workspace_I_Load61_q/1
  qd219/2 -> To Workspace_I_Load61_d/1
  [I_Load62] -> qd220/1
  [angle_ref] -> qd220/2
  qd220/1 -> To Workspace_I_Load62_q/1
  qd220/2 -> To Workspace_I_Load62_d/1
  [I_Load63] -> qd221/1
  [angle_ref] -> qd221/2
  qd221/1 -> To Workspace_I_Load63_q/1
  qd221/2 -> To Workspace_I_Load63_d/1
  [I_Load64] -> qd222/1
  [angle_ref] -> qd222/2
  qd222/1 -> To Workspace_I_Load64_q/1
  qd222/2 -> To Workspace_I_Load64_d/1
  [I_Load65] -> qd223/1
  [angle_ref] -> qd223/2
  qd223/1 -> To Workspace_I_Load65_q/1
  qd223/2 -> To Workspace_I_Load65_d/1
  [I_Load66] -> qd224/1
  [angle_ref] -> qd224/2
  qd224/1 -> To Workspace_I_Load66_q/1
  qd224/2 -> To Workspace_I_Load66_d/1
  [I_Load67] -> qd225/1
  [angle_ref] -> qd225/2
  qd225/1 -> To Workspace_I_Load67_q/1
  qd225/2 -> To Workspace_I_Load67_d/1
  [I_Load68] -> qd226/1
  [angle_ref] -> qd226/2
  qd226/1 -> To Workspace_I_Load68_q/1
  qd226/2 -> To Workspace_I_Load68_d/1
  [I_Load69] -> qd227/1
  [angle_ref] -> qd227/2
  qd227/1 -> To Workspace_I_Load69_q/1
  qd227/2 -> To Workspace_I_Load69_d/1
  [I_Load70] -> qd228/1
  [angle_ref] -> qd228/2
  qd228/1 -> To Workspace_I_Load70_q/1
  qd228/2 -> To Workspace_I_Load70_d/1
  [I_Load71] -> qd229/1
  [angle_ref] -> qd229/2
  qd229/1 -> To Workspace_I_Load71_q/1
  qd229/2 -> To Workspace_I_Load71_d/1
  [I_Load72] -> qd230/1
  [angle_ref] -> qd230/2
  qd230/1 -> To Workspace_I_Load72_q/1
  qd230/2 -> To Workspace_I_Load72_d/1
  [I_Load73] -> qd231/1
  [angle_ref] -> qd231/2
  qd231/1 -> To Workspace_I_Load73_q/1
  qd231/2 -> To Workspace_I_Load73_d/1
  [I_Load74] -> qd232/1
  [angle_ref] -> qd232/2
  qd232/1 -> To Workspace_I_Load74_q/1
  qd232/2 -> To Workspace_I_Load74_d/1
  [I_Load75] -> qd233/1
  [angle_ref] -> qd233/2
  qd233/1 -> To Workspace_I_Load75_q/1
  qd233/2 -> To Workspace_I_Load75_d/1
  [I_Load76] -> qd234/1
  [angle_ref] -> qd234/2
  qd234/1 -> To Workspace_I_Load76_q/1
  qd234/2 -> To Workspace_I_Load76_d/1
  [I_Load77] -> qd235/1
  [angle_ref] -> qd235/2
  qd235/1 -> To Workspace_I_Load77_q/1
  qd235/2 -> To Workspace_I_Load77_d/1
  [I_Load78] -> qd236/1
  [angle_ref] -> qd236/2
  qd236/1 -> To Workspace_I_Load78_q/1
  qd236/2 -> To Workspace_I_Load78_d/1
  [I_Load79] -> qd237/1
  [angle_ref] -> qd237/2
  qd237/1 -> To Workspace_I_Load79_q/1
  qd237/2 -> To Workspace_I_Load79_d/1
  [I_Load80] -> qd238/1
  [angle_ref] -> qd238/2
  qd238/1 -> To Workspace_I_Load80_q/1
  qd238/2 -> To Workspace_I_Load80_d/1
  [I_Load81] -> qd239/1
  [angle_ref] -> qd239/2
  qd239/1 -> To Workspace_I_Load81_q/1
  qd239/2 -> To Workspace_I_Load81_d/1
  [I_Load82] -> qd240/1
  [angle_ref] -> qd240/2
  qd240/1 -> To Workspace_I_Load82_q/1
  qd240/2 -> To Workspace_I_Load82_d/1
  [I_Load83] -> qd241/1
  [angle_ref] -> qd241/2
  qd241/1 -> To Workspace_I_Load83_q/1
  qd241/2 -> To Workspace_I_Load83_d/1
  [I_Load84] -> qd242/1
  [angle_ref] -> qd242/2
  qd242/1 -> To Workspace_I_Load84_q/1
  qd242/2 -> To Workspace_I_Load84_d/1
  [I_Load85] -> qd243/1
  [angle_ref] -> qd243/2
  qd243/1 -> To Workspace_I_Load85_q/1
  qd243/2 -> To Workspace_I_Load85_d/1
  [I_Load86] -> qd244/1
  [angle_ref] -> qd244/2
  qd244/1 -> To Workspace_I_Load86_q/1
  qd244/2 -> To Workspace_I_Load86_d/1
  [I_Load87] -> qd245/1
  [angle_ref] -> qd245/2
  qd245/1 -> To Workspace_I_Load87_q/1
  qd245/2 -> To Workspace_I_Load87_d/1
  [I_Load88] -> qd246/1
  [angle_ref] -> qd246/2
  qd246/1 -> To Workspace_I_Load88_q/1
  qd246/2 -> To Workspace_I_Load88_d/1
  [I_Load89] -> qd247/1
  [angle_ref] -> qd247/2
  qd247/1 -> To Workspace_I_Load89_q/1
  qd247/2 -> To Workspace_I_Load89_d/1
  [I_Load90] -> qd248/1
  [angle_ref] -> qd248/2
  qd248/1 -> To Workspace_I_Load90_q/1
  qd248/2 -> To Workspace_I_Load90_d/1
  [I_Load91] -> qd249/1
  [angle_ref] -> qd249/2
  qd249/1 -> To Workspace_I_Load91_q/1
  qd249/2 -> To Workspace_I_Load91_d/1
  [w_SG1] -> To WorkspaceSG1_w/1
  [w_GFOL_RL1] -> To WorkspaceGFOL_RL1_w/1
  [w_SG2] -> To WorkspaceSG2_w/1
  [w_GFOL_RL2] -> To WorkspaceGFOL_RL2_w/1
  [w_SG3] -> To WorkspaceSG3_w/1
  [w_GFOL_RL3] -> To WorkspaceGFOL_RL3_w/1
  [w_SG4] -> To WorkspaceSG4_w/1
  [w_GFOL_RL4] -> To WorkspaceGFOL_RL4_w/1
  [w_SG5] -> To WorkspaceSG5_w/1
  [w_GFOL_RL5] -> To WorkspaceGFOL_RL5_w/1
  [w_SG6] -> To WorkspaceSG6_w/1
  [w_GFOL_RL6] -> To WorkspaceGFOL_RL6_w/1
  [w_SG7] -> To WorkspaceSG7_w/1
  [w_GFOL_RL7] -> To WorkspaceGFOL_RL7_w/1
  [w_SG8] -> To WorkspaceSG8_w/1
  [w_GFOL_RL8] -> To WorkspaceGFOL_RL8_w/1
  [w_SG9] -> To WorkspaceSG9_w/1
  [w_GFOL_RL9] -> To WorkspaceGFOL_RL9_w/1
  [w_SG10] -> To WorkspaceSG10_w/1
  [w_GFOL_RL10] -> To WorkspaceGFOL_RL10_w/1
  [w_GFOR11] -> To WorkspaceGFOR11_w/1
  [w_SG11] -> To WorkspaceSG11_w/1
  [w_GFOR12] -> To WorkspaceGFOR12_w/1
  [w_SG12] -> To WorkspaceSG12_w/1
  [w_GFOR13] -> To WorkspaceGFOR13_w/1
  [w_SG13] -> To WorkspaceSG13_w/1
  [w_GFOR14] -> To WorkspaceGFOR14_w/1
  [w_SG14] -> To WorkspaceSG14_w/1
  [w_SG15] -> To WorkspaceSG15_w/1
  [w_GFOR15] -> To WorkspaceGFOR15_w/1
  [w_SG16] -> To WorkspaceSG16_w/1
  [w_GFOR16] -> To WorkspaceGFOR16_w/1
  [w_SG17] -> To WorkspaceSG17_w/1
  [w_GFOR17] -> To WorkspaceGFOR17_w/1
  [w_SG18] -> To WorkspaceSG18_w/1
  [w_GFOR18] -> To WorkspaceGFOR18_w/1
  [w_SG19] -> To WorkspaceSG19_w/1
  [w_GFOR19] -> To WorkspaceGFOR19_w/1
  [w_SG20] -> To WorkspaceSG20_w/1
  [w_GFOR20] -> To WorkspaceGFOR20_w/1
  [w_SG21] -> To WorkspaceSG21_w/1
  [w_SG22] -> To WorkspaceSG22_w/1
  [w_SG23] -> To WorkspaceSG23_w/1
  [w_SG24] -> To WorkspaceSG24_w/1
  [w_SG25] -> To WorkspaceSG25_w/1
  [w_SG26] -> To WorkspaceSG26_w/1
  connections:
  BUS-Load-39/LConn1 -- BUS-49/RConn1 -- Line-75/LConn1 -- Line-62/RConn1 -- Line-69/RConn1 -- Line-66/RConn1
  BUS-Load-39/LConn2 -- BUS-49/RConn2 -- Line-75/LConn2 -- Line-62/RConn2 -- Line-69/RConn2 -- Line-66/RConn2
  BUS-Load-39/LConn3 -- BUS-49/RConn3 -- Line-75/LConn3 -- Line-62/RConn3 -- Line-69/RConn3 -- Line-66/RConn3
  BUS-Load-39/RConn1 -- Load-39/LConn1
  BUS-Load-39/RConn2 -- Load-39/LConn2
  BUS-Load-39/RConn3 -- Load-39/LConn3
  BUS-SG-8/RConn1 -- BUS-49/LConn1 -- Line-72/LConn1 -- Line-76/LConn1 -- Line-71/RConn1 -- Line-74/LConn1 -- Line-73/LConn1
  BUS-SG-8/RConn2 -- BUS-49/LConn2 -- Line-72/LConn2 -- Line-76/LConn2 -- Line-71/RConn2 -- Line-74/LConn2 -- Line-73/LConn2
  BUS-SG-8/RConn3 -- BUS-49/LConn3 -- Line-72/LConn3 -- Line-76/LConn3 -- Line-71/RConn3 -- Line-74/LConn3 -- Line-73/LConn3
  BUS-SG-8/LConn1 -- SG-8/RConn1
  BUS-SG-8/LConn2 -- SG-8/RConn2
  BUS-SG-8/LConn3 -- SG-8/RConn3
  Line-72/RConn1 -- BUS-50/RConn1
  Line-72/RConn2 -- BUS-50/RConn2
  Line-72/RConn3 -- BUS-50/RConn3
  BUS-Load-40/LConn1 -- BUS-50/LConn1 -- Line-77/LConn1
  BUS-Load-40/LConn2 -- BUS-50/LConn2 -- Line-77/LConn2
  BUS-Load-40/LConn3 -- BUS-50/LConn3 -- Line-77/LConn3
  BUS-Load-40/RConn1 -- Load-40/LConn1
  BUS-Load-40/RConn2 -- Load-40/LConn2
  BUS-Load-40/RConn3 -- Load-40/LConn3
  BUS-57/RConn1 -- Line-77/RConn1 -- Line-87/RConn1
  BUS-57/RConn2 -- Line-77/RConn2 -- Line-87/RConn2
  BUS-57/RConn3 -- Line-77/RConn3 -- Line-87/RConn3
  BUS-57/LConn1 -- BUS-Load-47/LConn1
  BUS-57/LConn2 -- BUS-Load-47/LConn2
  BUS-57/LConn3 -- BUS-Load-47/LConn3
  BUS-Load-47/RConn1 -- Load-47/LConn1
  BUS-Load-47/RConn2 -- Load-47/LConn2
  BUS-Load-47/RConn3 -- Load-47/LConn3
  Line-87/LConn1 -- BUS-56/LConn1 -- BUS-Load-46/LConn1 -- Line-88/LConn1
  Line-87/LConn2 -- BUS-56/LConn2 -- BUS-Load-46/LConn2 -- Line-88/LConn2
  Line-87/LConn3 -- BUS-56/LConn3 -- BUS-Load-46/LConn3 -- Line-88/LConn3
  BUS-Load-46/RConn1 -- Load-46/LConn1
  BUS-Load-46/RConn2 -- Load-46/LConn2
  BUS-Load-46/RConn3 -- Load-46/LConn3
  BUS-58/RConn1 -- Line-88/RConn1 -- Line-79/RConn1
  BUS-58/RConn2 -- Line-88/RConn2 -- Line-79/RConn2
  BUS-58/RConn3 -- Line-88/RConn3 -- Line-79/RConn3
  BUS-58/LConn1 -- BUS-Load-48/LConn1
  BUS-58/LConn2 -- BUS-Load-48/LConn2
  BUS-58/LConn3 -- BUS-Load-48/LConn3
  BUS-Load-48/RConn1 -- Load-48/LConn1
  BUS-Load-48/RConn2 -- Load-48/LConn2
  BUS-Load-48/RConn3 -- Load-48/LConn3
  Line-79/LConn1 -- BUS-51/LConn1 -- Line-78/LConn1
  Line-79/LConn2 -- BUS-51/LConn2 -- Line-78/LConn2
  Line-79/LConn3 -- BUS-51/LConn3 -- Line-78/LConn3
  BUS-Load-41/LConn1 -- BUS-51/RConn1 -- Line-73/RConn1
  BUS-Load-41/LConn2 -- BUS-51/RConn2 -- Line-73/RConn2
  BUS-Load-41/LConn3 -- BUS-51/RConn3 -- Line-73/RConn3
  BUS-Load-41/RConn1 -- Load-41/LConn1
  BUS-Load-41/RConn2 -- Load-41/LConn2
  BUS-Load-41/RConn3 -- Load-41/LConn3
  BUS-52/RConn1 -- Line-78/RConn1 -- Line-80/LConn1
  BUS-52/RConn2 -- Line-78/RConn2 -- Line-80/LConn2
  BUS-52/RConn3 -- Line-78/RConn3 -- Line-80/LConn3
  BUS-52/LConn1 -- BUS-Load-42/LConn1
  BUS-52/LConn2 -- BUS-Load-42/LConn2
  BUS-52/LConn3 -- BUS-Load-42/LConn3
  BUS-Load-42/RConn1 -- Load-42/LConn1
  BUS-Load-42/RConn2 -- Load-42/LConn2
  BUS-Load-42/RConn3 -- Load-42/LConn3
  BUS-53/LConn1 -- Line-80/RConn1 -- BUS-Load-43/LConn1
  BUS-53/LConn2 -- Line-80/RConn2 -- BUS-Load-43/LConn2
  BUS-53/LConn3 -- Line-80/RConn3 -- BUS-Load-43/LConn3
  BUS-Load-43/RConn1 -- Load-43/LConn1
  BUS-Load-43/RConn2 -- Load-43/LConn2
  BUS-Load-43/RConn3 -- Load-43/LConn3
  BUS-53/RConn1 -- Line-81/LConn1
  BUS-53/RConn2 -- Line-81/LConn2
  BUS-53/RConn3 -- Line-81/LConn3
  Line-81/RConn1 -- BUS-SG-9/RConn1 -- BUS-VSC-4/RConn1 -- BUS-VSC-14/RConn1 -- Line-82/LConn1 -- BUS-54/LConn1 -- Line-83/LConn1
  Line-81/RConn2 -- BUS-SG-9/RConn2 -- BUS-VSC-4/RConn2 -- BUS-VSC-14/RConn2 -- Line-82/LConn2 -- BUS-54/LConn2 -- Line-83/LConn2
  Line-81/RConn3 -- BUS-SG-9/RConn3 -- BUS-VSC-4/RConn3 -- BUS-VSC-14/RConn3 -- Line-82/LConn3 -- BUS-54/LConn3 -- Line-83/LConn3
  BUS-Load-44/LConn1 -- BUS-54/RConn1 -- Line-84/LConn1 -- Line-74/RConn1
  BUS-Load-44/LConn2 -- BUS-54/RConn2 -- Line-84/LConn2 -- Line-74/RConn2
  BUS-Load-44/LConn3 -- BUS-54/RConn3 -- Line-84/LConn3 -- Line-74/RConn3
  BUS-Load-44/RConn1 -- Load-44/LConn1
  BUS-Load-44/RConn2 -- Load-44/LConn2
  BUS-Load-44/RConn3 -- Load-44/LConn3
  BUS-SG-9/LConn1 -- SG-9/RConn1
  BUS-SG-9/LConn2 -- SG-9/RConn2
  BUS-SG-9/LConn3 -- SG-9/RConn3
  BUS-VSC-4/LConn1 -- VSC-4/RConn1
  BUS-VSC-4/LConn2 -- VSC-4/RConn2
  BUS-VSC-4/LConn3 -- VSC-4/RConn3
  BUS-VSC-14/LConn1 -- VSC-14/RConn1
  BUS-VSC-14/LConn2 -- VSC-14/RConn2
  BUS-VSC-14/LConn3 -- VSC-14/RConn3
  BUS-55/RConn1 -- Line-82/RConn1 -- Line-86/LConn1
  BUS-55/RConn2 -- Line-82/RConn2 -- Line-86/LConn2
  BUS-55/RConn3 -- Line-82/RConn3 -- Line-86/LConn3
  BUS-Load-45/LConn1 -- BUS-55/LConn1 -- Line-85/LConn1
  BUS-Load-45/LConn2 -- BUS-55/LConn2 -- Line-85/LConn2
  BUS-Load-45/LConn3 -- BUS-55/LConn3 -- Line-85/LConn3
  BUS-Load-45/RConn1 -- Load-45/LConn1
  BUS-Load-45/RConn2 -- Load-45/LConn2
  BUS-Load-45/RConn3 -- Load-45/LConn3
  Line-85/RConn1 -- Line-89/LConn1 -- BUS-56/RConn1 -- Line-83/RConn1
  Line-85/RConn2 -- Line-89/LConn2 -- BUS-56/RConn2 -- Line-83/RConn2
  Line-85/RConn3 -- Line-89/LConn3 -- BUS-56/RConn3 -- Line-83/RConn3
  Line-89/RConn1 -- BUS-SG-10/RConn1 -- Line-84/RConn1 -- BUS-59/LConn1 -- Line-86/RConn1
  Line-89/RConn2 -- BUS-SG-10/RConn2 -- Line-84/RConn2 -- BUS-59/LConn2 -- Line-86/RConn2
  Line-89/RConn3 -- BUS-SG-10/RConn3 -- Line-84/RConn3 -- BUS-59/LConn3 -- Line-86/RConn3
  BUS-Load-49/LConn1 -- BUS-59/RConn1 -- Line-90/LConn1 -- Line-170/LConn1 -- Line-91/LConn1
  BUS-Load-49/LConn2 -- BUS-59/RConn2 -- Line-90/LConn2 -- Line-170/LConn2 -- Line-91/LConn2
  BUS-Load-49/LConn3 -- BUS-59/RConn3 -- Line-90/LConn3 -- Line-170/LConn3 -- Line-91/LConn3
  BUS-Load-49/RConn1 -- Load-49/LConn1
  BUS-Load-49/RConn2 -- Load-49/LConn2
  BUS-Load-49/RConn3 -- Load-49/LConn3
  BUS-SG-10/LConn1 -- SG-10/RConn1
  BUS-SG-10/LConn2 -- SG-10/RConn2
  BUS-SG-10/LConn3 -- SG-10/RConn3
  Line-90/RConn1 -- BUS-60/LConn1
  Line-90/RConn2 -- BUS-60/LConn2
  Line-90/RConn3 -- BUS-60/LConn3
  BUS-Load-50/LConn1 -- BUS-60/RConn1 -- Line-92/LConn1 -- Line-93/LConn1
  BUS-Load-50/LConn2 -- BUS-60/RConn2 -- Line-92/LConn2 -- Line-93/LConn2
  BUS-Load-50/LConn3 -- BUS-60/RConn3 -- Line-92/LConn3 -- Line-93/LConn3
  BUS-Load-50/RConn1 -- Load-50/LConn1
  BUS-Load-50/RConn2 -- Load-50/LConn2
  BUS-Load-50/RConn3 -- Load-50/LConn3
  BUS-61/LConn1 -- Line-92/RConn1 -- Line-91/RConn1
  BUS-61/LConn2 -- Line-92/RConn2 -- Line-91/RConn2
  BUS-61/LConn3 -- Line-92/RConn3 -- Line-91/RConn3
  Line-94/LConn1 -- BUS-61/RConn1 -- Line-171/LConn1
  Line-94/LConn2 -- BUS-61/RConn2 -- Line-171/LConn2
  Line-94/LConn3 -- BUS-61/RConn3 -- Line-171/LConn3
  BUS-62/LConn1 -- Line-94/RConn1 -- Line-93/RConn1
  BUS-62/LConn2 -- Line-94/RConn2 -- Line-93/RConn2
  BUS-62/LConn3 -- Line-94/RConn3 -- Line-93/RConn3
  BUS-Load-51/LConn1 -- BUS-62/RConn1 -- Line-95/LConn1 -- Line-96/LConn1
  BUS-Load-51/LConn2 -- BUS-62/RConn2 -- Line-95/LConn2 -- Line-96/LConn2
  BUS-Load-51/LConn3 -- BUS-62/RConn3 -- Line-95/LConn3 -- Line-96/LConn3
  BUS-Load-51/RConn1 -- Load-51/LConn1
  BUS-Load-51/RConn2 -- Load-51/LConn2
  BUS-Load-51/RConn3 -- Load-51/LConn3
  BUS-66/LConn1 -- Line-95/RConn1 -- Line-75/RConn1
  BUS-66/LConn2 -- Line-95/RConn2 -- Line-75/RConn2
  BUS-66/LConn3 -- Line-95/RConn3 -- Line-75/RConn3
  BUS-Load-52/LConn1 -- BUS-66/RConn1 -- Line-100/LConn1 -- Line-172/RConn1
  BUS-Load-52/LConn2 -- BUS-66/RConn2 -- Line-100/LConn2 -- Line-172/RConn2
  BUS-Load-52/LConn3 -- BUS-66/RConn3 -- Line-100/LConn3 -- Line-172/RConn3
  BUS-Load-52/RConn1 -- Load-52/LConn1
  BUS-Load-52/RConn2 -- Load-52/LConn2
  BUS-Load-52/RConn3 -- Load-52/LConn3
  BUS-67/LConn1 -- Line-100/RConn1 -- Line-96/RConn1
  BUS-67/LConn2 -- Line-100/RConn2 -- Line-96/RConn2
  BUS-67/LConn3 -- Line-100/RConn3 -- Line-96/RConn3
  BUS-67/RConn1 -- BUS-Load-53/LConn1
  BUS-67/RConn2 -- BUS-Load-53/LConn2
  BUS-67/RConn3 -- BUS-Load-53/LConn3
  BUS-Load-53/RConn1 -- Load-53/LConn1
  BUS-Load-53/RConn2 -- Load-53/LConn2
  BUS-Load-53/RConn3 -- Load-53/LConn3
  Line-172/LConn1 -- BUS-65/LConn1 -- Line-99/LConn1 -- Line-98/RConn1
  Line-172/LConn2 -- BUS-65/LConn2 -- Line-99/LConn2 -- Line-98/RConn2
  Line-172/LConn3 -- BUS-65/LConn3 -- Line-99/LConn3 -- Line-98/RConn3
  BUS-SG-11/RConn1 -- BUS-65/RConn1 -- Line-57/RConn1
  BUS-SG-11/RConn2 -- BUS-65/RConn2 -- Line-57/RConn2
  BUS-SG-11/RConn3 -- BUS-65/RConn3 -- Line-57/RConn3
  BUS-SG-11/LConn1 -- SG-11/RConn1
  BUS-SG-11/LConn2 -- SG-11/RConn2
  BUS-SG-11/LConn3 -- SG-11/RConn3
  Line-99/RConn1 -- BUS-68/RConn1
  Line-99/RConn2 -- BUS-68/RConn2
  Line-99/RConn3 -- BUS-68/RConn3
  Line-101/LConn1 -- BUS-68/LConn1 -- Line-173/LConn1
  Line-101/LConn2 -- BUS-68/LConn2 -- Line-173/LConn2
  Line-101/LConn3 -- BUS-68/LConn3 -- Line-173/LConn3
  Line-101/RConn1 -- BUS-81/RConn1
  Line-101/RConn2 -- BUS-81/RConn2
  Line-101/RConn3 -- BUS-81/RConn3
  Line-174/LConn1 -- BUS-80/RConn1 -- Line-120/LConn1 -- Line-121/LConn1 -- Line-122/LConn1 -- Line-123/LConn1
  Line-174/LConn2 -- BUS-80/RConn2 -- Line-120/LConn2 -- Line-121/LConn2 -- Line-122/LConn2 -- Line-123/LConn2
  Line-174/LConn3 -- BUS-80/RConn3 -- Line-120/LConn3 -- Line-121/LConn3 -- Line-122/LConn3 -- Line-123/LConn3
  Line-174/RConn1 -- BUS-81/LConn1
  Line-174/RConn2 -- BUS-81/LConn2
  Line-174/RConn3 -- BUS-81/LConn3
  BUS-Load-61/LConn1 -- BUS-80/LConn1 -- BUS-SG-17/RConn1 -- Line-119/RConn1 -- Line-116/RConn1
  BUS-Load-61/LConn2 -- BUS-80/LConn2 -- BUS-SG-17/RConn2 -- Line-119/RConn2 -- Line-116/RConn2
  BUS-Load-61/LConn3 -- BUS-80/LConn3 -- BUS-SG-17/RConn3 -- Line-119/RConn3 -- Line-116/RConn3
  BUS-Load-61/RConn1 -- Load-61/LConn1
  BUS-Load-61/RConn2 -- Load-61/LConn2
  BUS-Load-61/RConn3 -- Load-61/LConn3
  BUS-SG-17/LConn1 -- SG-17/RConn1
  BUS-SG-17/LConn2 -- SG-17/RConn2
  BUS-SG-17/LConn3 -- SG-17/RConn3
  BUS-96/LConn1 -- Line-120/RConn1 -- Line-125/RConn1
  BUS-96/LConn2 -- Line-120/RConn2 -- Line-125/RConn2
  BUS-96/LConn3 -- Line-120/RConn3 -- Line-125/RConn3
  BUS-Load-73/LConn1 -- BUS-96/RConn1 -- Line-146/LConn1 -- Line-145/RConn1 -- Line-143/RConn1
  BUS-Load-73/LConn2 -- BUS-96/RConn2 -- Line-146/LConn2 -- Line-145/RConn2 -- Line-143/RConn2
  BUS-Load-73/LConn3 -- BUS-96/RConn3 -- Line-146/LConn3 -- Line-145/RConn3 -- Line-143/RConn3
  BUS-Load-73/RConn1 -- Load-73/LConn1
  BUS-Load-73/RConn2 -- Load-73/LConn2
  BUS-Load-73/RConn3 -- Load-73/LConn3
  BUS-97/LConn1 -- Line-146/RConn1 -- Line-121/RConn1
  BUS-97/LConn2 -- Line-146/RConn2 -- Line-121/RConn2
  BUS-97/LConn3 -- Line-146/RConn3 -- Line-121/RConn3
  BUS-97/RConn1 -- BUS-Load-74/LConn1
  BUS-97/RConn2 -- BUS-Load-74/LConn2
  BUS-97/RConn3 -- BUS-Load-74/LConn3
  BUS-Load-74/RConn1 -- Load-74/LConn1
  BUS-Load-74/RConn2 -- Load-74/LConn2
  BUS-Load-74/RConn3 -- Load-74/LConn3
  Line-125/LConn1 -- BUS-82/RConn1 -- Line-117/RConn1
  Line-125/LConn2 -- BUS-82/RConn2 -- Line-117/RConn2
  Line-125/LConn3 -- BUS-82/RConn3 -- Line-117/RConn3
  BUS-Load-62/LConn1 -- BUS-82/LConn1 -- Line-124/LConn1
  BUS-Load-62/LConn2 -- BUS-82/LConn2 -- Line-124/LConn2
  BUS-Load-62/LConn3 -- BUS-82/LConn3 -- Line-124/LConn3
  BUS-Load-62/RConn1 -- Load-62/LConn1
  BUS-Load-62/RConn2 -- Load-62/LConn2
  BUS-Load-62/RConn3 -- Load-62/LConn3
  Line-124/RConn1 -- BUS-83/RConn1
  Line-124/RConn2 -- BUS-83/RConn2
  Line-124/RConn3 -- BUS-83/RConn3
  BUS-Load-63/LConn1 -- BUS-83/LConn1 -- Line-126/LConn1 -- Line-127/LConn1
  BUS-Load-63/LConn2 -- BUS-83/LConn2 -- Line-126/LConn2 -- Line-127/LConn2
  BUS-Load-63/LConn3 -- BUS-83/LConn3 -- Line-126/LConn3 -- Line-127/LConn3
  BUS-Load-63/RConn1 -- Load-63/LConn1
  BUS-Load-63/RConn2 -- Load-63/LConn2
  BUS-Load-63/RConn3 -- Load-63/LConn3
  BUS-84/RConn1 -- Line-126/RConn1 -- Line-128/LConn1
  BUS-84/RConn2 -- Line-126/RConn2 -- Line-128/LConn2
  BUS-84/RConn3 -- Line-126/RConn3 -- Line-128/LConn3
  BUS-84/LConn1 -- BUS-Load-64/LConn1
  BUS-84/LConn2 -- BUS-Load-64/LConn2
  BUS-84/LConn3 -- BUS-Load-64/LConn3
  BUS-Load-64/RConn1 -- Load-64/LConn1
  BUS-Load-64/RConn2 -- Load-64/LConn2
  BUS-Load-64/RConn3 -- Load-64/LConn3
  Line-128/RConn1 -- BUS-Load-65/LConn1 -- BUS-SG-18/RConn1 -- BUS-85/LConn1 -- Line-129/LConn1
  Line-128/RConn2 -- BUS-Load-65/LConn2 -- BUS-SG-18/RConn2 -- BUS-85/LConn2 -- Line-129/LConn2
  Line-128/RConn3 -- BUS-Load-65/LConn3 -- BUS-SG-18/RConn3 -- BUS-85/LConn3 -- Line-129/LConn3
  BUS-Load-65/RConn1 -- Load-65/LConn1
  BUS-Load-65/RConn2 -- Load-65/LConn2
  BUS-Load-65/RConn3 -- Load-65/LConn3
  BUS-SG-18/LConn1 -- SG-18/RConn1
  BUS-SG-18/LConn2 -- SG-18/RConn2
  BUS-SG-18/LConn3 -- SG-18/RConn3
  Line-129/RConn1 -- BUS-86/RConn1
  Line-129/RConn2 -- BUS-86/RConn2
  Line-129/RConn3 -- BUS-86/RConn3
  BUS-86/LConn1 -- BUS-Load-66/LConn1
  BUS-86/LConn2 -- BUS-Load-66/LConn2
  BUS-86/LConn3 -- BUS-Load-66/LConn3
  BUS-Load-66/RConn1 -- Load-66/LConn1
  BUS-Load-66/RConn2 -- Load-66/LConn2
  BUS-Load-66/RConn3 -- Load-66/LConn3
  Line-130/LConn1 -- BUS-85/RConn1 -- Line-131/LConn1 -- Line-127/RConn1
  Line-130/LConn2 -- BUS-85/RConn2 -- Line-131/LConn2 -- Line-127/RConn2
  Line-130/LConn3 -- BUS-85/RConn3 -- Line-131/LConn3 -- Line-127/RConn3
  BUS-88/LConn1 -- Line-130/RConn1 -- BUS-Load-67/LConn1
  BUS-88/LConn2 -- Line-130/RConn2 -- BUS-Load-67/LConn2
  BUS-88/LConn3 -- Line-130/RConn3 -- BUS-Load-67/LConn3
  BUS-Load-67/RConn1 -- Load-67/LConn1
  BUS-Load-67/RConn2 -- Load-67/LConn2
  BUS-Load-67/RConn3 -- Load-67/LConn3
  BUS-88/RConn1 -- Line-132/LConn1
  BUS-88/RConn2 -- Line-132/LConn2
  BUS-88/RConn3 -- Line-132/LConn3
